simulink model "DYN_03x"  (R2021a)
settings: Solver=FixedStepAuto  StartTime=0.0  StopTime=10  FixedStep=0.001  RelTol=1e-3
(part 2 of 9)

== matlab function DYN_03x/MATLAB Function ==
  data: t input; e input; dde output; de input; Pic input; I1 input; I2 input; I3 input; I4 input; I5 input; I6 input; c input; b input; Fe input
function dde = fcn(t,e,de,Pic,I1,I2,I3,I4,I5,I6,c,b,Fe)
e1 = e(1); e2 = e(2); e3 = e(3);
e4 = e(4); e5 = e(5); e6 = e(6);
de1 = de(1); de2 = de(2); de3 = de(3);
de4 = de(4); de5 = de(5); de6 = de(6);
x1 = Pic(1,1); y1 = Pic(1,2); z1 = Pic(1,3);
x2 = Pic(2,1); y2 = Pic(2,2); z2 = Pic(2,3);
x3 = Pic(3,1); y3 = Pic(3,2); z3 = Pic(3,3);
x4 = Pic(4,1); y4 = Pic(4,2); z4 = Pic(4,3);
x5 = Pic(5,1); y5 = Pic(5,2); z5 = Pic(5,3);
x6 = Pic(6,1); y6 = Pic(6,2); z6 = Pic(6,3);
I1xx = I1(1,1); I1xy = I1(1,2); I1xz = I1(1,3);
I1yx = I1(2,1); I1yy = I1(2,2); I1yz = I1(2,3);
I1zx = I1(3,1); I1zy = I1(3,2); I1zz = I1(3,3);

I2xx = I2(1,1); I2xy = I2(1,2); I2xz = I2(1,3);
I2yx = I2(2,1); I2yy = I2(2,2); I2yz = I2(2,3);
I2zx = I2(3,1); I2zy = I2(3,2); I2zz = I2(3,3);

I3xx = I3(1,1); I3xy = I3(1,2); I3xz = I3(1,3);
I3yx = I3(2,1); I3yy = I3(2,2); I3yz = I3(2,3);
I3zx = I3(3,1); I3zy = I3(3,2); I3zz = I3(3,3);

I4xx = I4(1,1); I4xy = I4(1,2); I4xz = I4(1,3);
I4yx = I4(2,1); I4yy = I4(2,2); I4yz = I4(2,3);
I4zx = I4(3,1); I4zy = I4(3,2); I4zz = I4(3,3);

I5xx = I5(1,1); I5xy = I5(1,2); I5xz = I5(1,3);
I5yx = I5(2,1); I5yy = I5(2,2); I5yz = I5(2,3);
I5zx = I5(3,1); I5zy = I5(3,2); I5zz = I5(3,3);

I6xx = I6(1,1); I6xy = I6(1,2); I6xz = I6(1,3);
I6yx = I6(2,1); I6yy = I6(2,2); I6yz = I6(2,3);
I6zx = I6(3,1); I6zy = I6(3,2); I6zz = I6(3,3);
a1=0.75; a2=2.70; a3=0.90; d1=3.35; d4=2.95; d7=0.80;
m0 = 7.2407; m1 = 5.6511; m2 = 4.6061; m3 = 4.2963; m4 = 1.9151; m5 = 0.3399; m6 = 0.0714;
g = 9.80665;
%% 
M = ...
[I1zz + m5*(a1*sin(e1) + z5*cos(e1)*cos(e4) + a2*sin(e1)*sin(e2) + d4*cos(e2)*cos(e3)*sin(e1) + a3*cos(e2)*sin(e1)*sin(e3) + a3*cos(e3)*sin(e1)*sin(e2) - x5*cos(e1)*cos(e5)*sin(e4) - d4*sin(e1)*sin(e2)*sin(e3) + y5*cos(e1)*sin(e4)*sin(e5) + y5*cos(e2)*cos(e3)*cos(e5)*sin(e1) + x5*cos(e2)*cos(e3)*sin(e1)*sin(e5) - y5*cos(e5)*sin(e1)*sin(e2)*sin(e3) + z5*cos(e2)*sin(e1)*sin(e3)*sin(e4) + z5*cos(e3)*sin(e1)*sin(e2)*sin(e4) - x5*sin(e1)*sin(e2)*sin(e3)*sin(e5) + x5*cos(e2)*cos(e4)*cos(e5)*sin(e1)*sin(e3) + x5*cos(e3)*cos(e4)*cos(e5)*sin(e1)*sin(e2) - y5*cos(e2)*cos(e4)*sin(e1)*sin(e3)*sin(e5) - y5*cos(e3)*cos(e4)*sin(e1)*sin(e2)*sin(e5))^2 + m6*(d4*cos(e1)*sin(e2)*sin(e3) - a2*cos(e1)*sin(e2) - d4*cos(e1)*cos(e2)*cos(e3) - a3*cos(e1)*cos(e2)*sin(e3) - a3*cos(e1)*cos(e3)*sin(e2) - a1*cos(e1) - y6*cos(e4)*cos(e6)*sin(e1) - x6*cos(e4)*sin(e1)*sin(e6) + z6*sin(e1)*sin(e4)*sin(e5) - x6*cos(e5)*cos(e6)*sin(e1)*sin(e4) + z6*cos(e1)*cos(e5)*sin(e2)*sin(e3) + y6*cos(e5)*sin(e1)*sin(e4)*sin(e6) - z6*cos(e1)*cos(e2)*cos(e3)*cos(e5) - y6*cos(e1)*sin(e2)*sin(e3)*sin(e5)*sin(e6) - x6*cos(e1)*cos(e2)*cos(e3)*cos(e6)*sin(e5) + y6*cos(e1)*cos(e2)*cos(e6)*sin(e3)*sin(e4) + y6*cos(e1)*cos(e3)*cos(e6)*sin(e2)*sin(e4) + y6*cos(e1)*cos(e2)*cos(e3)*sin(e5)*sin(e6) + z6*cos(e1)*cos(e2)*cos(e4)*sin(e3)*sin(e5) + z6*cos(e1)*cos(e3)*cos(e4)*sin(e2)*sin(e5) + x6*cos(e1)*cos(e2)*sin(e3)*sin(e4)*sin(e6) + x6*cos(e1)*cos(e3)*sin(e2)*sin(e4)*sin(e6) + x6*cos(e1)*cos(e6)*sin(e2)*sin(e3)*sin(e5) - x6*cos(e1)*cos(e2)*cos(e4)*cos(e5)*cos(e6)*sin(e3) - x6*cos(e1)*cos(e3)*cos(e4)*cos(e5)*cos(e6)*sin(e2) + y6*cos(e1)*cos(e2)*cos(e4)*cos(e5)*sin(e3)*sin(e6) + y6*cos(e1)*cos(e3)*cos(e4)*cos(e5)*sin(e2)*sin(e6))^2 + m6*(y6*cos(e1)*cos(e4)*cos(e6) - a2*sin(e1)*sin(e2) - d4*cos(e2)*cos(e3)*sin(e1) - a1*sin(e1) - a3*cos(e2)*sin(e1)*sin(e3) - a3*cos(e3)*sin(e1)*sin(e2) + x6*cos(e1)*cos(e4)*sin(e6) + d4*sin(e1)*sin(e2)*sin(e3) - z6*cos(e1)*sin(e4)*sin(e5) + x6*cos(e1)*cos(e5)*cos(e6)*sin(e4) - z6*cos(e2)*cos(e3)*cos(e5)*sin(e1) - y6*cos(e1)*cos(e5)*sin(e4)*sin(e6) + z6*cos(e5)*sin(e1)*sin(e2)*sin(e3) + x6*cos(e2)*sin(e1)*sin(e3)*sin(e4)*sin(e6) + x6*cos(e3)*sin(e1)*sin(e2)*sin(e4)*sin(e6) + x6*cos(e6)*sin(e1)*sin(e2)*sin(e3)*sin(e5) - y6*sin(e1)*sin(e2)*sin(e3)*sin(e5)*sin(e6) - x6*cos(e2)*cos(e3)*cos(e6)*sin(e1)*sin(e5) + y6*cos(e2)*cos(e6)*sin(e1)*sin(e3)*sin(e4) + y6*cos(e3)*cos(e6)*sin(e1)*sin(e2)*sin(e4) + y6*cos(e2)*cos(e3)*sin(e1)*sin(e5)*sin(e6) + z6*cos(e2)*cos(e4)*sin(e1)*sin(e3)*sin(e5) + z6*cos(e3)*cos(e4)*sin(e1)*sin(e2)*sin(e5) - x6*cos(e2)*cos(e4)*cos(e5)*cos(e6)*sin(e1)*sin(e3) - x6*cos(e3)*cos(e4)*cos(e5)*cos(e6)*sin(e1)*sin(e2) + y6*cos(e2)*cos(e4)*cos(e5)*sin(e1)*sin(e3)*sin(e6) + y6*cos(e3)*cos(e4)*cos(e5)*sin(e1)*sin(e2)*sin(e6))^2 + m3*(sin(e1)*(a1 + y3*cos(e2 + e3) + x3*sin(e2 + e3) + a2*sin(e2)) + z3*cos(e2 + e3)^2*cos(e1) + z3*sin(e2 + e3)^2*cos(e1))^2 + m3*(z3*cos(e2 + e3)^2*sin(e1) - cos(e1)*(a1 + y3*cos(e2 + e3) + x3*sin(e2 + e3) + a2*sin(e2)) + z3*sin(e2 + e3)^2*sin(e1))^2 + m5*(a1*cos(e1) + a2*cos(e1)*sin(e2) - z5*cos(e4)*sin(e1) + d4*cos(e1)*cos(e2)*cos(e3) + a3*cos(e1)*cos(e2)*sin(e3) + a3*cos(e1)*cos(e3)*sin(e2) - d4*cos(e1)*sin(e2)*sin(e3) + x5*cos(e5)*sin(e1)*sin(e4) - y5*sin(e1)*sin(e4)*sin(e5) + x5*cos(e1)*cos(e2)*cos(e3)*sin(e5) - y5*cos(e1)*cos(e5)*sin(e2)*sin(e3) + z5*cos(e1)*cos(e2)*sin(e3)*sin(e4) + z5*cos(e1)*cos(e3)*sin(e2)*sin(e4) - x5*cos(e1)*sin(e2)*sin(e3)*sin(e5) + y5*cos(e1)*cos(e2)*cos(e3)*cos(e5) + x5*cos(e1)*cos(e2)*cos(e4)*cos(e5)*sin(e3) + x5*cos(e1)*cos(e3)*cos(e4)*cos(e5)*sin(e2) - y5*cos(e1)*cos(e2)*cos(e4)*sin(e3)*sin(e5) - y5*cos(e1)*cos(e3)*cos(e4)*sin(e2)*sin(e5))^2 + m4*(a1*sin(e1) - y4*cos(e1)*cos(e4) + a2*sin(e1)*sin(e2) - x4*cos(e1)*sin(e4) + d4*cos(e2)*cos(e3)*sin(e1) + a3*cos(e2)*sin(e1)*sin(e3) + a3*cos(e3)*sin(e1)*sin(e2) + z4*cos(e2)*cos(e3)*sin(e1) - d4*sin(e1)*sin(e2)*sin(e3) - z4*sin(e1)*sin(e2)*sin(e3) + x4*cos(e2)*cos(e4)*sin(e1)*sin(e3) + x4*cos(e3)*cos(e4)*sin(e1)*sin(e2) - y4*cos(e2)*sin(e1)*sin(e3)*sin(e4) - y4*cos(e3)*sin(e1)*sin(e2)*sin(e4))^2 + I3xx*cos(e2 + e3)^2 + I3yy*sin(e2 + e3)^2 + I4zz*sin(e2 + e3)^2 + m2*(a1*cos(e1) - z2*sin(e1) + y2*cos(e1)*cos(e2) + x2*cos(e1)*sin(e2))^2 + I5xx*(sin(e2 + e3)*sin(e5) - cos(e2 + e3)*cos(e4)*cos(e5))^2 + I5yy*(sin(e2 + e3)*cos(e5) + cos(e2 + e3)*cos(e4)*sin(e5))^2 + I6zz*(sin(e2 + e3)*cos(e5) + cos(e2 + e3)*cos(e4)*sin(e5))^2 + m2*(a1*sin(e1) + z2*cos(e1) + y2*cos(e2)*sin(e1) + x2*sin(e1)*sin(e2))^2 + I2xx*cos(e2)^2 + m1*(y1*cos(e1) + x1*sin(e1))^2 + m1*(x1*cos(e1) - y1*sin(e1))^2 + I2yy*sin(e2)^2 + I6xx*(cos(e2 + e3)*sin(e4)*sin(e6) + sin(e2 + e3)*cos(e6)*sin(e5) - cos(e2 + e3)*cos(e4)*cos(e5)*cos(e6))^2 + m4*(a1*cos(e1) + a2*cos(e1)*sin(e2) + y4*cos(e4)*sin(e1) + x4*sin(e1)*sin(e4) + d4*cos(e1)*cos(e2)*cos(e3) + a3*cos(e1)*cos(e2)*sin(e3) + a3*cos(e1)*cos(e3)*sin(e2) + z4*cos(e1)*cos(e2)*cos(e3) - d4*cos(e1)*sin(e2)*sin(e3) - z4*cos(e1)*sin(e2)*sin(e3) + x4*cos(e1)*cos(e2)*cos(e4)*sin(e3) + x4*cos(e1)*cos(e3)*cos(e4)*sin(e2) - y4*cos(e1)*cos(e2)*sin(e3)*sin(e4) - y4*cos(e1)*cos(e3)*sin(e2)*sin(e4))^2 + I6yy*(cos(e2 + e3)*cos(e6)*sin(e4) - sin(e2 + e3)*sin(e5)*sin(e6) + cos(e2 + e3)*cos(e4)*cos(e5)*sin(e6))^2 + I4xx*cos(e2 + e3)^2*cos(e4)^2 + I4yy*cos(e2 + e3)^2*sin(e4)^2 + I5zz*cos(e2 + e3)^2*sin(e4)^2,m2*y2*z2*sin(e2) - m2*x2*z2*cos(e2) - a2*m3*z3*cos(e2) + a2*m4*y4*cos(e2)*cos(e4) - a2*m5*z5*cos(e2)*cos(e4) + a2*m4*x4*cos(e2)*sin(e4) - m4*x4*y4*cos(e2)*cos(e3) - m3*x3*z3*cos(e2)*cos(e3) + m3*y3*z3*cos(e2)*sin(e3) + m3*y3*z3*cos(e3)*sin(e2) + m4*x4*y4*sin(e2)*sin(e3) + m3*x3*z3*sin(e2)*sin(e3) - I4xx*cos(e2)*cos(e3)*cos(e4)*sin(e4) + I6xx*cos(e2)*cos(e3)*cos(e4)*sin(e4) + I4yy*cos(e2)*cos(e3)*cos(e4)*sin(e4) - I5yy*cos(e2)*cos(e3)*cos(e4)*sin(e4) + I5zz*cos(e2)*cos(e3)*cos(e4)*sin(e4) - I6zz*cos(e2)*cos(e3)*cos(e4)*sin(e4) + I4xx*cos(e4)*sin(e2)*sin(e3)*sin(e4) - I6xx*cos(e4)*sin(e2)*sin(e3)*sin(e4) - I4yy*cos(e4)*sin(e2)*sin(e3)*sin(e4) + I5yy*cos(e4)*sin(e2)*sin(e3)*sin(e4) - I5zz*cos(e4)*sin(e2)*sin(e3)*sin(e4) + I6zz*cos(e4)*sin(e2)*sin(e3)*sin(e4) - a3*m5*z5*cos(e2)*cos(e3)*cos(e4) - I5xx*cos(e2)*cos(e3)*cos(e4)*cos(e5)^2*sin(e4) - I6xx*cos(e2)*cos(e3)*cos(e4)*cos(e6)^2*sin(e4) + I5yy*cos(e2)*cos(e3)*cos(e4)*cos(e5)^2*sin(e4) - I6yy*cos(e2)*cos(e3)*cos(e4)*cos(e5)^2*sin(e4) + I6yy*cos(e2)*cos(e3)*cos(e4)*cos(e6)^2*sin(e4) + I6zz*cos(e2)*cos(e3)*cos(e4)*cos(e5)^2*sin(e4) + a3*m4*x4*cos(e2)*cos(e3)*sin(e4) + a2*m5*x5*cos(e2)*cos(e5)*sin(e4) + a2*m6*x6*cos(e2)*cos(e4)*sin(e6) - d4*m4*y4*cos(e2)*cos(e4)*sin(e3) - d4*m4*y4*cos(e3)*cos(e4)*sin(e2) + d4*m5*z5*cos(e2)*cos(e4)*sin(e3) + d4*m5*z5*cos(e3)*cos(e4)*sin(e2) + m6*x6*y6*cos(e2)*cos(e3)*cos(e5) + m5*x5*z5*cos(e2)*cos(e3)*cos(e5) - a3*m4*y4*cos(e4)*sin(e2)*sin(e3) - a2*m5*y5*cos(e2)*sin(e4)*sin(e5) + a3*m5*z5*cos(e4)*sin(e2)*sin(e3) - a2*m6*z6*cos(e2)*sin(e4)*sin(e5) - d4*m4*x4*cos(e2)*sin(e3)*sin(e4) - d4*m4*x4*cos(e3)*sin(e2)*sin(e4) + I5xx*cos(e4)*cos(e5)^2*sin(e2)*sin(e3)*sin(e4) + I6xx*cos(e4)*cos(e6)^2*sin(e2)*sin(e3)*sin(e4) - I5yy*cos(e4)*cos(e5)^2*sin(e2)*sin(e3)*sin(e4) + I6yy*cos(e4)*cos(e5)^2*sin(e2)*sin(e3)*sin(e4) - I6yy*cos(e4)*cos(e6)^2*sin(e2)*sin(e3)*sin(e4) - I6zz*cos(e4)*cos(e5)^2*sin(e2)*sin(e3)*sin(e4) - m4*y4*z4*cos(e2)*cos(e4)*sin(e3) - m4*y4*z4*cos(e3)*cos(e4)*sin(e2) - m5*y5*z5*cos(e2)*cos(e3)*sin(e5) - a3*m4*x4*sin(e2)*sin(e3)*sin(e4) + m5*x5*y5*cos(e2)*sin(e3)*sin(e4) + m5*x5*y5*cos(e3)*sin(e2)*sin(e4) - m6*x6*y6*cos(e5)*sin(e2)*sin(e3) - m4*x4*z4*cos(e2)*sin(e3)*sin(e4) - m4*x4*z4*cos(e3)*sin(e2)*sin(e4) - m5*x5*z5*cos(e5)*sin(e2)*sin(e3) + m5*y5*z5*sin(e2)*sin(e3)*sin(e5) + 2*m4*x4*y4*cos(e2)*cos(e3)*cos(e4)^2 - 2*m4*x4*y4*cos(e4)^2*sin(e2)*sin(e3) + I6xx*cos(e2)*cos(e3)*cos(e5)*cos(e6)*sin(e6) - I6yy*cos(e2)*cos(e3)*cos(e5)*cos(e6)*sin(e6) + I5xx*cos(e2)*cos(e5)*sin(e3)*sin(e4)*sin(e5) + I5xx*cos(e3)*cos(e5)*sin(e2)*sin(e4)*sin(e5) - I6xx*cos(e5)*cos(e6)*sin(e2)*sin(e3)*sin(e6) - I5yy*cos(e2)*cos(e5)*sin(e3)*sin(e4)*sin(e5) - I5yy*cos(e3)*cos(e5)*sin(e2)*sin(e4)*sin(e5) + I6yy*cos(e2)*cos(e5)*sin(e3)*sin(e4)*sin(e5) + I6yy*cos(e3)*cos(e5)*sin(e2)*sin(e4)*sin(e5) + I6yy*cos(e5)*cos(e6)*sin(e2)*sin(e3)*sin(e6) - I6zz*cos(e2)*cos(e5)*sin(e3)*sin(e4)*sin(e5) - I6zz*cos(e3)*cos(e5)*sin(e2)*sin(e4)*sin(e5) + m4*x4^2*cos(e2)*cos(e3)*cos(e4)*sin(e4) - m6*x6^2*cos(e2)*cos(e3)*cos(e4)*sin(e4) - m4*y4^2*cos(e2)*cos(e3)*cos(e4)*sin(e4) + m5*y5^2*cos(e2)*cos(e3)*cos(e4)*sin(e4) - m5*z5^2*cos(e2)*cos(e3)*cos(e4)*sin(e4) + m6*z6^2*cos(e2)*cos(e3)*cos(e4)*sin(e4) - m4*x4^2*cos(e4)*sin(e2)*sin(e3)*sin(e4) + m6*x6^2*cos(e4)*sin(e2)*sin(e3)*sin(e4) + m4*y4^2*cos(e4)*sin(e2)*sin(e3)*sin(e4) - m5*y5^2*cos(e4)*sin(e2)*sin(e3)*sin(e4) + m5*z5^2*cos(e4)*sin(e2)*sin(e3)*sin(e4) - m6*z6^2*cos(e4)*sin(e2)*sin(e3)*sin(e4) + a3*m4*y4*cos(e2)*cos(e3)*cos(e4) + a2*m6*y6*cos(e2)*cos(e4)*cos(e6) + m5*x5*z5*cos(e2)*cos(e4)*sin(e3)*sin(e5) + m5*x5*z5*cos(e3)*cos(e4)*sin(e2)*sin(e5) + m6*x6*z6*cos(e2)*cos(e6)*sin(e3)*sin(e4) + m6*x6*z6*cos(e3)*cos(e6)*sin(e2)*sin(e4) + m6*x6*z6*cos(e2)*cos(e3)*sin(e5)*sin(e6) + a3*m5*y5*sin(e2)*sin(e3)*sin(e4)*sin(e5) + a3*m6*z6*sin(e2)*sin(e3)*sin(e4)*sin(e5) - m6*y6*z6*cos(e2)*sin(e3)*sin(e4)*sin(e6) - m6*y6*z6*cos(e3)*sin(e2)*sin(e4)*sin(e6) - m6*y6*z6*cos(e6)*sin(e2)*sin(e3)*sin(e5) - m5*x5^2*cos(e4)*cos(e5)^2*sin(e2)*sin(e3)*sin(e4) - m6*x6^2*cos(e4)*cos(e6)^2*sin(e2)*sin(e3)*sin(e4) + m5*y5^2*cos(e4)*cos(e5)^2*sin(e2)*sin(e3)*sin(e4) - m6*y6^2*cos(e4)*cos(e5)^2*sin(e2)*sin(e3)*sin(e4) + m6*y6^2*cos(e4)*cos(e6)^2*sin(e2)*sin(e3)*sin(e4) + m6*z6^2*cos(e4)*cos(e5)^2*sin(e2)*sin(e3)*sin(e4) - m6*x6*z6*sin(e2)*sin(e3)*sin(e5)*sin(e6) - I6xx*cos(e2)*cos(e3)*cos(e4)*cos(e5)^2*cos(e6)^2*sin(e4) + I6yy*cos(e2)*cos(e3)*cos(e4)*cos(e5)^2*cos(e6)^2*sin(e4) - 2*m6*x6*y6*cos(e2)*cos(e3)*cos(e4)^2*cos(e5) - 2*m6*x6*y6*cos(e2)*cos(e3)*cos(e5)*cos(e6)^2 - 2*m5*x5*z5*cos(e2)*cos(e3)*cos(e4)^2*cos(e5) + I6xx*cos(e4)*cos(e5)^2*cos(e6)^2*sin(e2)*sin(e3)*sin(e4) - I6yy*cos(e4)*cos(e5)^2*cos(e6)^2*sin(e2)*sin(e3)*sin(e4) + 2*m5*y5*z5*cos(e2)*cos(e3)*cos(e4)^2*sin(e5) - 2*m5*x5*y5*cos(e2)*cos(e5)^2*sin(e3)*sin(e4) - 2*m5*x5*y5*cos(e3)*cos(e5)^2*sin(e2)*sin(e4) + 2*m6*x6*y6*cos(e4)^2*cos(e5)*sin(e2)*sin(e3) + 2*m6*x6*y6*cos(e5)*cos(e6)^2*sin(e2)*sin(e3) + 2*m5*x5*z5*cos(e4)^2*cos(e5)*sin(e2)*sin(e3) - 2*m5*y5*z5*cos(e4)^2*sin(e2)*sin(e3)*sin(e5) + I6xx*cos(e2)*cos(e4)*cos(e6)*sin(e3)*sin(e5)*sin(e6) + I6xx*cos(e3)*cos(e4)*cos(e6)*sin(e2)*sin(e5)*sin(e6) - I6yy*cos(e2)*cos(e4)*cos(e6)*sin(e3)*sin(e5)*sin(e6) - I6yy*cos(e3)*cos(e4)*cos(e6)*sin(e2)*sin(e5)*sin(e6) - m6*x6^2*cos(e2)*cos(e3)*cos(e5)*cos(e6)*sin(e6) + m6*y6^2*cos(e2)*cos(e3)*cos(e5)*cos(e6)*sin(e6) - m5*x5^2*cos(e2)*cos(e5)*sin(e3)*sin(e4)*sin(e5) - m5*x5^2*cos(e3)*cos(e5)*sin(e2)*sin(e4)*sin(e5) + m6*x6^2*cos(e5)*cos(e6)*sin(e2)*sin(e3)*sin(e6) + m5*y5^2*cos(e2)*cos(e5)*sin(e3)*sin(e4)*sin(e5) + m5*y5^2*cos(e3)*cos(e5)*sin(e2)*sin(e4)*sin(e5) - m6*y6^2*cos(e2)*cos(e5)*sin(e3)*sin(e4)*sin(e5) - m6*y6^2*cos(e3)*cos(e5)*sin(e2)*sin(e4)*sin(e5) - m6*y6^2*cos(e5)*cos(e6)*sin(e2)*sin(e3)*sin(e6) + m6*z6^2*cos(e2)*cos(e5)*sin(e3)*sin(e4)*sin(e5) + m6*z6^2*cos(e3)*cos(e5)*sin(e2)*sin(e4)*sin(e5) + a3*m6*y6*cos(e2)*cos(e3)*cos(e4)*cos(e6) - 2*I6xx*cos(e2)*cos(e3)*cos(e4)^2*cos(e5)*cos(e6)*sin(e6) + 2*I6yy*cos(e2)*cos(e3)*cos(e4)^2*cos(e5)*cos(e6)*sin(e6) + a3*m5*x5*cos(e2)*cos(e3)*cos(e5)*sin(e4) + a3*m6*x6*cos(e2)*cos(e3)*cos(e4)*sin(e6) + a2*m6*x6*cos(e2)*cos(e5)*cos(e6)*sin(e4) - d4*m6*y6*cos(e2)*cos(e4)*cos(e6)*sin(e3) - d4*m6*y6*cos(e3)*cos(e4)*cos(e6)*sin(e2) - a3*m5*y5*cos(e2)*cos(e3)*sin(e4)*sin(e5) - a3*m6*y6*cos(e4)*cos(e6)*sin(e2)*sin(e3) - a2*m6*y6*cos(e2)*cos(e5)*sin(e4)*sin(e6) - a3*m6*z6*cos(e2)*cos(e3)*sin(e4)*sin(e5) - d4*m5*x5*cos(e2)*cos(e5)*sin(e3)*sin(e4) - d4*m5*x5*cos(e3)*cos(e5)*sin(e2)*sin(e4) - d4*m6*x6*cos(e2)*cos(e4)*sin(e3)*sin(e6) - d4*m6*x6*cos(e3)*cos(e4)*sin(e2)*sin(e6) + I6xx*cos(e2)*cos(e5)*cos(e6)^2*sin(e3)*sin(e4)*sin(e5) + I6xx*cos(e3)*cos(e5)*cos(e6)^2*sin(e2)*sin(e4)*sin(e5) + 2*I6xx*cos(e4)^2*cos(e5)*cos(e6)*sin(e2)*sin(e3)*sin(e6) - I6yy*cos(e2)*cos(e5)*cos(e6)^2*sin(e3)*sin(e4)*sin(e5) - I6yy*cos(e3)*cos(e5)*cos(e6)^2*sin(e2)*sin(e4)*sin(e5) - 2*I6yy*cos(e4)^2*cos(e5)*cos(e6)*sin(e2)*sin(e3)*sin(e6) + m5*y5*z5*cos(e2)*cos(e4)*cos(e5)*sin(e3) + m5*y5*z5*cos(e3)*cos(e4)*cos(e5)*sin(e2) + m6*y6*z6*cos(e2)*cos(e3)*cos(e6)*sin(e5) - a3*m5*x5*cos(e5)*sin(e2)*sin(e3)*sin(e4) - a3*m6*x6*cos(e4)*sin(e2)*sin(e3)*sin(e6) + d4*m5*y5*cos(e2)*sin(e3)*sin(e4)*sin(e5) + d4*m5*y5*cos(e3)*sin(e2)*sin(e4)*sin(e5) + d4*m6*z6*cos(e2)*sin(e3)*sin(e4)*sin(e5) + d4*m6*z6*cos(e3)*sin(e2)*sin(e4)*sin(e5) + m5*x5^2*cos(e2)*cos(e3)*cos(e4)*cos(e5)^2*sin(e4) + m6*x6^2*cos(e2)*cos(e3)*cos(e4)*cos(e6)^2*sin(e4) - m5*y5^2*cos(e2)*cos(e3)*cos(e4)*cos(e5)^2*sin(e4) + m6*y6^2*cos(e2)*cos(e3)*cos(e4)*cos(e5)^2*sin(e4) - m6*y6^2*cos(e2)*cos(e3)*cos(e4)*cos(e6)^2*sin(e4) + m6*x6*y6*cos(e2)*cos(e4)*sin(e3)*sin(e5) + m6*x6*y6*cos(e3)*cos(e4)*sin(e2)*sin(e5) - m6*z6^2*cos(e2)*cos(e3)*cos(e4)*cos(e5)^2*sin(e4) - 2*m6*y6*z6*cos(e2)*cos(e3)*cos(e4)^2*cos(e6)*sin(e5) + m6*x6^2*cos(e2)*cos(e3)*cos(e4)*cos(e5)^2*cos(e6)^2*sin(e4) - m6*y6^2*cos(e2)*cos(e3)*cos(e4)*cos(e5)^2*cos(e6)^2*sin(e4) - 2*m6*x6*y6*cos(e2)*cos(e4)*cos(e6)^2*sin(e3)*sin(e5) - 2*m6*x6*y6*cos(e3)*cos(e4)*cos(e6)^2*sin(e2)*sin(e5) - 2*m6*x6*z6*cos(e2)*cos(e3)*cos(e4)^2*sin(e5)*sin(e6) - 2*m6*x6*z6*cos(e2)*cos(e5)^2*cos(e6)*sin(e3)*sin(e4) - 2*m6*x6*z6*cos(e3)*cos(e5)^2*cos(e6)*sin(e2)*sin(e4) + 2*m6*y6*z6*cos(e2)*cos(e5)^2*sin(e3)*sin(e4)*sin(e6) + 2*m6*y6*z6*cos(e3)*cos(e5)^2*sin(e2)*sin(e4)*sin(e6) + 2*m6*y6*z6*cos(e4)^2*cos(e6)*sin(e2)*sin(e3)*sin(e5) - m6*x6^2*cos(e4)*cos(e5)^2*cos(e6)^2*sin(e2)*sin(e3)*sin(e4) + m6*y6^2*cos(e4)*cos(e5)^2*cos(e6)^2*sin(e2)*sin(e3)*sin(e4) + 2*m6*x6*z6*cos(e4)^2*sin(e2)*sin(e3)*sin(e5)*sin(e6) + 4*m6*x6*y6*cos(e2)*cos(e3)*cos(e4)^2*cos(e5)*cos(e6)^2 - m6*x6^2*cos(e2)*cos(e4)*cos(e6)*sin(e3)*sin(e5)*sin(e6) - m6*x6^2*cos(e3)*cos(e4)*cos(e6)*sin(e2)*sin(e5)*sin(e6) - 4*m6*x6*y6*cos(e4)^2*cos(e5)*cos(e6)^2*sin(e2)*sin(e3) + m6*y6^2*cos(e2)*cos(e4)*cos(e6)*sin(e3)*sin(e5)*sin(e6) + m6*y6^2*cos(e3)*cos(e4)*cos(e6)*sin(e2)*sin(e5)*sin(e6) + a3*m6*x6*cos(e2)*cos(e3)*cos(e5)*cos(e6)*sin(e4) - a3*m6*y6*cos(e2)*cos(e3)*cos(e5)*sin(e4)*sin(e6) - d4*m6*x6*cos(e2)*cos(e5)*cos(e6)*sin(e3)*sin(e4) - d4*m6*x6*cos(e3)*cos(e5)*cos(e6)*sin(e2)*sin(e4) - m6*y6*z6*cos(e2)*cos(e4)*cos(e5)*cos(e6)*sin(e3) - m6*y6*z6*cos(e3)*cos(e4)*cos(e5)*cos(e6)*sin(e2) - a3*m6*x6*cos(e5)*cos(e6)*sin(e2)*sin(e3)*sin(e4) + d4*m6*y6*cos(e2)*cos(e5)*sin(e3)*sin(e4)*sin(e6) + d4*m6*y6*cos(e3)*cos(e5)*sin(e2)*sin(e4)*sin(e6) + 2*m6*x6^2*cos(e2)*cos(e3)*cos(e4)^2*cos(e5)*cos(e6)*sin(e6) - 2*m6*y6^2*cos(e2)*cos(e3)*cos(e4)^2*cos(e5)*cos(e6)*sin(e6) - m6*x6*z6*cos(e2)*cos(e4)*cos(e5)*sin(e3)*sin(e6) - m6*x6*z6*cos(e3)*cos(e4)*cos(e5)*sin(e2)*sin(e6) + a3*m6*y6*cos(e5)*sin(e2)*sin(e3)*sin(e4)*sin(e6) - m6*x6^2*cos(e2)*cos(e5)*cos(e6)^2*sin(e3)*sin(e4)*sin(e5) - m6*x6^2*cos(e3)*cos(e5)*cos(e6)^2*sin(e2)*sin(e4)*sin(e5) - 2*m6*x6^2*cos(e4)^2*cos(e5)*cos(e6)*sin(e2)*sin(e3)*sin(e6) + m6*y6^2*cos(e2)*cos(e5)*cos(e6)^2*sin(e3)*sin(e4)*sin(e5) + m6*y6^2*cos(e3)*cos(e5)*cos(e6)^2*sin(e2)*sin(e4)*sin(e5) + 2*m6*y6^2*cos(e4)^2*cos(e5)*cos(e6)*sin(e2)*sin(e3)*sin(e6) - 2*m5*x5*y5*cos(e2)*cos(e3)*cos(e4)*cos(e5)*sin(e4)*sin(e5) - 2*m6*x6*y6*cos(e2)*cos(e3)*cos(e4)*cos(e6)*sin(e4)*sin(e6) + 2*m5*x5*y5*cos(e4)*cos(e5)*sin(e2)*sin(e3)*sin(e4)*sin(e5) + 2*m6*x6*y6*cos(e4)*cos(e6)*sin(e2)*sin(e3)*sin(e4)*sin(e6) - 2*m6*x6*z6*cos(e2)*cos(e3)*cos(e4)*cos(e5)*cos(e6)*sin(e4)*sin(e5) + 2*m6*y6*z6*cos(e2)*cos(e3)*cos(e4)*cos(e5)*sin(e4)*sin(e5)*sin(e6) + 2*m6*x6*y6*cos(e2)*cos(e5)*cos(e6)*sin(e3)*sin(e4)*sin(e5)*sin(e6) + 2*m6*x6*y6*cos(e3)*cos(e5)*cos(e6)*sin(e2)*sin(e4)*sin(e5)*sin(e6) + 2*m6*x6*z6*cos(e4)*cos(e5)*cos(e6)*sin(e2)*sin(e3)*sin(e4)*sin(e5) - 2*m6*y6*z6*cos(e4)*cos(e5)*sin(e2)*sin(e3)*sin(e4)*sin(e5)*sin(e6) - 2*m6*x6*y6*cos(e2)*cos(e3)*cos(e4)*cos(e5)^2*cos(e6)*sin(e4)*sin(e6) + 2*m6*x6*y6*cos(e4)*cos(e5)^2*cos(e6)*sin(e2)*sin(e3)*sin(e4)*sin(e6),m3*y3*z3*cos(e2)*sin(e3) - m3*x3*z3*cos(e2)*cos(e3) - m4*x4*y4*cos(e2)*cos(e3) + m3*y3*z3*cos(e3)*sin(e2) + m4*x4*y4*sin(e2)*sin(e3) + m3*x3*z3*sin(e2)*sin(e3) - I4xx*cos(e2)*cos(e3)*cos(e4)*sin(e4) + I6xx*cos(e2)*cos(e3)*cos(e4)*sin(e4) + I4yy*cos(e2)*cos(e3)*cos(e4)*sin(e4) - I5yy*cos(e2)*cos(e3)*cos(e4)*sin(e4) + I5zz*cos(e2)*cos(e3)*cos(e4)*sin(e4) - I6zz*cos(e2)*cos(e3)*cos(e4)*sin(e4) + I4xx*cos(e4)*sin(e2)*sin(e3)*sin(e4) - I6xx*cos(e4)*sin(e2)*sin(e3)*sin(e4) - I4yy*cos(e4)*sin(e2)*sin(e3)*sin(e4) + I5yy*cos(e4)*sin(e2)*sin(e3)*sin(e4) - I5zz*cos(e4)*sin(e2)*sin(e3)*sin(e4) + I6zz*cos(e4)*sin(e2)*sin(e3)*sin(e4) - a3*m5*z5*cos(e2)*cos(e3)*cos(e4) - I5xx*cos(e2)*cos(e3)*cos(e4)*cos(e5)^2*sin(e4) - I6xx*cos(e2)*cos(e3)*cos(e4)*cos(e6)^2*sin(e4) + I5yy*cos(e2)*cos(e3)*cos(e4)*cos(e5)^2*sin(e4) - I6yy*cos(e2)*cos(e3)*cos(e4)*cos(e5)^2*sin(e4) + I6yy*cos(e2)*cos(e3)*cos(e4)*cos(e6)^2*sin(e4) + I6zz*cos(e2)*cos(e3)*cos(e4)*cos(e5)^2*sin(e4) + a3*m4*x4*cos(e2)*cos(e3)*sin(e4) - d4*m4*y4*cos(e2)*cos(e4)*sin(e3) - d4*m4*y4*cos(e3)*cos(e4)*sin(e2) + d4*m5*z5*cos(e2)*cos(e4)*sin(e3) + d4*m5*z5*cos(e3)*cos(e4)*sin(e2) + m6*x6*y6*cos(e2)*cos(e3)*cos(e5) + m5*x5*z5*cos(e2)*cos(e3)*cos(e5) - a3*m4*y4*cos(e4)*sin(e2)*sin(e3) + a3*m5*z5*cos(e4)*sin(e2)*sin(e3) - d4*m4*x4*cos(e2)*sin(e3)*sin(e4) - d4*m4*x4*cos(e3)*sin(e2)*sin(e4) + I5xx*cos(e4)*cos(e5)^2*sin(e2)*sin(e3)*sin(e4) + I6xx*cos(e4)*cos(e6)^2*sin(e2)*sin(e3)*sin(e4) - I5yy*cos(e4)*cos(e5)^2*sin(e2)*sin(e3)*sin(e4) + I6yy*cos(e4)*cos(e5)^2*sin(e2)*sin(e3)*sin(e4) - I6yy*cos(e4)*cos(e6)^2*sin(e2)*sin(e3)*sin(e4) - I6zz*cos(e4)*cos(e5)^2*sin(e2)*sin(e3)*sin(e4) - m4*y4*z4*cos(e2)*cos(e4)*sin(e3) - m4*y4*z4*cos(e3)*cos(e4)*sin(e2) - m5*y5*z5*cos(e2)*cos(e3)*sin(e5) - a3*m4*x4*sin(e2)*sin(e3)*sin(e4) + m5*x5*y5*cos(e2)*sin(e3)*sin(e4) + m5*x5*y5*cos(e3)*sin(e2)*sin(e4) - m6*x6*y6*cos(e5)*sin(e2)*sin(e3) - m4*x4*z4*cos(e2)*sin(e3)*sin(e4) - m4*x4*z4*cos(e3)*sin(e2)*sin(e4) - m5*x5*z5*cos(e5)*sin(e2)*sin(e3) + m5*y5*z5*sin(e2)*sin(e3)*sin(e5) + 2*m4*x4*y4*cos(e2)*cos(e3)*cos(e4)^2 - 2*m4*x4*y4*cos(e4)^2*sin(e2)*sin(e3) + I6xx*cos(e2)*cos(e3)*cos(e5)*cos(e6)*sin(e6) - I6yy*cos(e2)*cos(e3)*cos(e5)*cos(e6)*sin(e6) + I5xx*cos(e2)*cos(e5)*sin(e3)*sin(e4)*sin(e5) + I5xx*cos(e3)*cos(e5)*sin(e2)*sin(e4)*sin(e5) - I6xx*cos(e5)*cos(e6)*sin(e2)*sin(e3)*sin(e6) - I5yy*cos(e2)*cos(e5)*sin(e3)*sin(e4)*sin(e5) - I5yy*cos(e3)*cos(e5)*sin(e2)*sin(e4)*sin(e5) + I6yy*cos(e2)*cos(e5)*sin(e3)*sin(e4)*sin(e5) + I6yy*cos(e3)*cos(e5)*sin(e2)*sin(e4)*sin(e5) + I6yy*cos(e5)*cos(e6)*sin(e2)*sin(e3)*sin(e6) - I6zz*cos(e2)*cos(e5)*sin(e3)*sin(e4)*sin(e5) - I6zz*cos(e3)*cos(e5)*sin(e2)*sin(e4)*sin(e5) + m4*x4^2*cos(e2)*cos(e3)*cos(e4)*sin(e4) - m6*x6^2*cos(e2)*cos(e3)*cos(e4)*sin(e4) - m4*y4^2*cos(e2)*cos(e3)*cos(e4)*sin(e4) + m5*y5^2*cos(e2)*cos(e3)*cos(e4)*sin(e4) - m5*z5^2*cos(e2)*cos(e3)*cos(e4)*sin(e4) + m6*z6^2*cos(e2)*cos(e3)*cos(e4)*sin(e4) - m4*x4^2*cos(e4)*sin(e2)*sin(e3)*sin(e4) + m6*x6^2*cos(e4)*sin(e2)*sin(e3)*sin(e4) + m4*y4^2*cos(e4)*sin(e2)*sin(e3)*sin(e4) - m5*y5^2*cos(e4)*sin(e2)*sin(e3)*sin(e4) + m5*z5^2*cos(e4)*sin(e2)*sin(e3)*sin(e4) - m6*z6^2*cos(e4)*sin(e2)*sin(e3)*sin(e4) + a3*m4*y4*cos(e2)*cos(e3)*cos(e4) + m5*x5*z5*cos(e2)*cos(e4)*sin(e3)*sin(e5) + m5*x5*z5*cos(e3)*cos(e4)*sin(e2)*sin(e5) + m6*x6*z6*cos(e2)*cos(e6)*sin(e3)*sin(e4) + m6*x6*z6*cos(e3)*cos(e6)*sin(e2)*sin(e4) + m6*x6*z6*cos(e2)*cos(e3)*sin(e5)*sin(e6) + a3*m5*y5*sin(e2)*sin(e3)*sin(e4)*sin(e5) + a3*m6*z6*sin(e2)*sin(e3)*sin(e4)*sin(e5) - m6*y6*z6*cos(e2)*sin(e3)*sin(e4)*sin(e6) - m6*y6*z6*cos(e3)*sin(e2)*sin(e4)*sin(e6) - m6*y6*z6*cos(e6)*sin(e2)*sin(e3)*sin(e5) - m5*x5^2*cos(e4)*cos(e5)^2*sin(e2)*sin(e3)*sin(e4) - m6*x6^2*cos(e4)*cos(e6)^2*sin(e2)*sin(e3)*sin(e4) + m5*y5^2*cos(e4)*cos(e5)^2*sin(e2)*sin(e3)*sin(e4) - m6*y6^2*cos(e4)*cos(e5)^2*sin(e2)*sin(e3)*sin(e4) + m6*y6^2*cos(e4)*cos(e6)^2*sin(e2)*sin(e3)*sin(e4) + m6*z6^2*cos(e4)*cos(e5)^2*sin(e2)*sin(e3)*sin(e4) - m6*x6*z6*sin(e2)*sin(e3)*sin(e5)*sin(e6) - I6xx*cos(e2)*cos(e3)*cos(e4)*cos(e5)^2*cos(e6)^2*sin(e4) + I6yy*cos(e2)*cos(e3)*cos(e4)*cos(e5)^2*cos(e6)^2*sin(e4) - 2*m6*x6*y6*cos(e2)*cos(e3)*cos(e4)^2*cos(e5) - 2*m6*x6*y6*cos(e2)*cos(e3)*cos(e5)*cos(e6)^2 - 2*m5*x5*z5*cos(e2)*cos(e3)*cos(e4)^2*cos(e5) + I6xx*cos(e4)*cos(e5)^2*cos(e6)^2*sin(e2)*sin(e3)*sin(e4) - I6yy*cos(e4)*cos(e5)^2*cos(e6)^2*sin(e2)*sin(e3)*sin(e4) + 2*m5*y5*z5*cos(e2)*cos(e3)*cos(e4)^2*sin(e5) - 2*m5*x5*y5*cos(e2)*cos(e5)^2*sin(e3)*sin(e4) - 2*m5*x5*y5*cos(e3)*cos(e5)^2*sin(e2)*sin(e4) + 2*m6*x6*y6*cos(e4)^2*cos(e5)*sin(e2)*sin(e3) + 2*m6*x6*y6*cos(e5)*cos(e6)^2*sin(e2)*sin(e3) + 2*m5*x5*z5*cos(e4)^2*cos(e5)*sin(e2)*sin(e3) - 2*m5*y5*z5*cos(e4)^2*sin(e2)*sin(e3)*sin(e5) + I6xx*cos(e2)*cos(e4)*cos(e6)*sin(e3)*sin(e5)*sin(e6) + I6xx*cos(e3)*cos(e4)*cos(e6)*sin(e2)*sin(e5)*sin(e6) - I6yy*cos(e2)*cos(e4)*cos(e6)*sin(e3)*sin(e5)*sin(e6) - I6yy*cos(e3)*cos(e4)*cos(e6)*sin(e2)*sin(e5)*sin(e6) - m6*x6^2*cos(e2)*cos(e3)*cos(e5)*cos(e6)*sin(e6) + m6*y6^2*cos(e2)*cos(e3)*cos(e5)*cos(e6)*sin(e6) - m5*x5^2*cos(e2)*cos(e5)*sin(e3)*sin(e4)*sin(e5) - m5*x5^2*cos(e3)*cos(e5)*sin(e2)*sin(e4)*sin(e5) + m6*x6^2*cos(e5)*cos(e6)*sin(e2)*sin(e3)*sin(e6) + m5*y5^2*cos(e2)*cos(e5)*sin(e3)*sin(e4)*sin(e5) + m5*y5^2*cos(e3)*cos(e5)*sin(e2)*sin(e4)*sin(e5) - m6*y6^2*cos(e2)*cos(e5)*sin(e3)*sin(e4)*sin(e5) - m6*y6^2*cos(e3)*cos(e5)*sin(e2)*sin(e4)*sin(e5) - m6*y6^2*cos(e5)*cos(e6)*sin(e2)*sin(e3)*sin(e6) + m6*z6^2*cos(e2)*cos(e5)*sin(e3)*sin(e4)*sin(e5) + m6*z6^2*cos(e3)*cos(e5)*sin(e2)*sin(e4)*sin(e5) + a3*m6*y6*cos(e2)*cos(e3)*cos(e4)*cos(e6) - 2*I6xx*cos(e2)*cos(e3)*cos(e4)^2*cos(e5)*cos(e6)*sin(e6) + 2*I6yy*cos(e2)*cos(e3)*cos(e4)^2*cos(e5)*cos(e6)*sin(e6) + a3*m5*x5*cos(e2)*cos(e3)*cos(e5)*sin(e4) + a3*m6*x6*cos(e2)*cos(e3)*cos(e4)*sin(e6) - d4*m6*y6*cos(e2)*cos(e4)*cos(e6)*sin(e3) - d4*m6*y6*cos(e3)*cos(e4)*cos(e6)*sin(e2) - a3*m5*y5*cos(e2)*cos(e3)*sin(e4)*sin(e5) - a3*m6*y6*cos(e4)*cos(e6)*sin(e2)*sin(e3) - a3*m6*z6*cos(e2)*cos(e3)*sin(e4)*sin(e5) - d4*m5*x5*cos(e2)*cos(e5)*sin(e3)*sin(e4) - d4*m5*x5*cos(e3)*cos(e5)*sin(e2)*sin(e4) - d4*m6*x6*cos(e2)*cos(e4)*sin(e3)*sin(e6) - d4*m6*x6*cos(e3)*cos(e4)*sin(e2)*sin(e6) + I6xx*cos(e2)*cos(e5)*cos(e6)^2*sin(e3)*sin(e4)*sin(e5) + I6xx*cos(e3)*cos(e5)*cos(e6)^2*sin(e2)*sin(e4)*sin(e5) + 2*I6xx*cos(e4)^2*cos(e5)*cos(e6)*sin(e2)*sin(e3)*sin(e6) - I6yy*cos(e2)*cos(e5)*cos(e6)^2*sin(e3)*sin(e4)*sin(e5) - I6yy*cos(e3)*cos(e5)*cos(e6)^2*sin(e2)*sin(e4)*sin(e5) - 2*I6yy*cos(e4)^2*cos(e5)*cos(e6)*sin(e2)*sin(e3)*sin(e6) + m5*y5*z5*cos(e2)*cos(e4)*cos(e5)*sin(e3) + m5*y5*z5*cos(e3)*cos(e4)*cos(e5)*sin(e2) + m6*y6*z6*cos(e2)*cos(e3)*cos(e6)*sin(e5) - a3*m5*x5*cos(e5)*sin(e2)*sin(e3)*sin(e4) - a3*m6*x6*cos(e4)*sin(e2)*sin(e3)*sin(e6) + d4*m5*y5*cos(e2)*sin(e3)*sin(e4)*sin(e5) + d4*m5*y5*cos(e3)*sin(e2)*sin(e4)*sin(e5) + d4*m6*z6*cos(e2)*sin(e3)*sin(e4)*sin(e5) + d4*m6*z6*cos(e3)*sin(e2)*sin(e4)*sin(e5) + m5*x5^2*cos(e2)*cos(e3)*cos(e4)*cos(e5)^2*sin(e4) + m6*x6^2*cos(e2)*cos(e3)*cos(e4)*cos(e6)^2*sin(e4) - m5*y5^2*cos(e2)*cos(e3)*cos(e4)*cos(e5)^2*sin(e4) + m6*y6^2*cos(e2)*cos(e3)*cos(e4)*cos(e5)^2*sin(e4) - m6*y6^2*cos(e2)*cos(e3)*cos(e4)*cos(e6)^2*sin(e4) + m6*x6*y6*cos(e2)*cos(e4)*sin(e3)*sin(e5) + m6*x6*y6*cos(e3)*cos(e4)*sin(e2)*sin(e5) - m6*z6^2*cos(e2)*cos(e3)*cos(e4)*cos(e5)^2*sin(e4) - 2*m6*y6*z6*cos(e2)*cos(e3)*cos(e4)^2*cos(e6)*sin(e5) + m6*x6^2*cos(e2)*cos(e3)*cos(e4)*cos(e5)^2*cos(e6)^2*sin(e4) - m6*y6^2*cos(e2)*cos(e3)*cos(e4)*cos(e5)^2*cos(e6)^2*sin(e4) - 2*m6*x6*y6*cos(e2)*cos(e4)*cos(e6)^2*sin(e3)*sin(e5) - 2*m6*x6*y6*cos(e3)*cos(e4)*cos(e6)^2*sin(e2)*sin(e5) - 2*m6*x6*z6*cos(e2)*cos(e3)*cos(e4)^2*sin(e5)*sin(e6) - 2*m6*x6*z6*cos(e2)*cos(e5)^2*cos(e6)*sin(e3)*sin(e4) - 2*m6*x6*z6*cos(e3)*cos(e5)^2*cos(e6)*sin(e2)*sin(e4) + 2*m6*y6*z6*cos(e2)*cos(e5)^2*sin(e3)*sin(e4)*sin(e6) + 2*m6*y6*z6*cos(e3)*cos(e5)^2*sin(e2)*sin(e4)*sin(e6) + 2*m6*y6*z6*cos(e4)^2*cos(e6)*sin(e2)*sin(e3)*sin(e5) - m6*x6^2*cos(e4)*cos(e5)^2*cos(e6)^2*sin(e2)*sin(e3)*sin(e4) + m6*y6^2*cos(e4)*cos(e5)^2*cos(e6)^2*sin(e2)*sin(e3)*sin(e4) + 2*m6*x6*z6*cos(e4)^2*sin(e2)*sin(e3)*sin(e5)*sin(e6) + 4*m6*x6*y6*cos(e2)*cos(e3)*cos(e4)^2*cos(e5)*cos(e6)^2 - m6*x6^2*cos(e2)*cos(e4)*cos(e6)*sin(e3)*sin(e5)*sin(e6) - m6*x6^2*cos(e3)*cos(e4)*cos(e6)*sin(e2)*sin(e5)*sin(e6) - 4*m6*x6*y6*cos(e4)^2*cos(e5)*cos(e6)^2*sin(e2)*sin(e3) + m6*y6^2*cos(e2)*cos(e4)*cos(e6)*sin(e3)*sin(e5)*sin(e6) + m6*y6^2*cos(e3)*cos(e4)*cos(e6)*sin(e2)*sin(e5)*sin(e6) + a3*m6*x6*cos(e2)*cos(e3)*cos(e5)*cos(e6)*sin(e4) - a3*m6*y6*cos(e2)*cos(e3)*cos(e5)*sin(e4)*sin(e6) - d4*m6*x6*cos(e2)*cos(e5)*cos(e6)*sin(e3)*sin(e4) - d4*m6*x6*cos(e3)*cos(e5)*cos(e6)*sin(e2)*sin(e4) - m6*y6*z6*cos(e2)*cos(e4)*cos(e5)*cos(e6)*sin(e3) - m6*y6*z6*cos(e3)*cos(e4)*cos(e5)*cos(e6)*sin(e2) - a3*m6*x6*cos(e5)*cos(e6)*sin(e2)*sin(e3)*sin(e4) + d4*m6*y6*cos(e2)*cos(e5)*sin(e3)*sin(e4)*sin(e6) + d4*m6*y6*cos(e3)*cos(e5)*sin(e2)*sin(e4)*sin(e6) + 2*m6*x6^2*cos(e2)*cos(e3)*cos(e4)^2*cos(e5)*cos(e6)*sin(e6) - 2*m6*y6^2*cos(e2)*cos(e3)*cos(e4)^2*cos(e5)*cos(e6)*sin(e6) - m6*x6*z6*cos(e2)*cos(e4)*cos(e5)*sin(e3)*sin(e6) - m6*x6*z6*cos(e3)*cos(e4)*cos(e5)*sin(e2)*sin(e6) + a3*m6*y6*cos(e5)*sin(e2)*sin(e3)*sin(e4)*sin(e6) - m6*x6^2*cos(e2)*cos(e5)*cos(e6)^2*sin(e3)*sin(e4)*sin(e5) - m6*x6^2*cos(e3)*cos(e5)*cos(e6)^2*sin(e2)*sin(e4)*sin(e5) - 2*m6*x6^2*cos(e4)^2*cos(e5)*cos(e6)*sin(e2)*sin(e3)*sin(e6) + m6*y6^2*cos(e2)*cos(e5)*cos(e6)^2*sin(e3)*sin(e4)*sin(e5) + m6*y6^2*cos(e3)*cos(e5)*cos(e6)^2*sin(e2)*sin(e4)*sin(e5) + 2*m6*y6^2*cos(e4)^2*cos(e5)*cos(e6)*sin(e2)*sin(e3)*sin(e6) - 2*m5*x5*y5*cos(e2)*cos(e3)*cos(e4)*cos(e5)*sin(e4)*sin(e5) - 2*m6*x6*y6*cos(e2)*cos(e3)*cos(e4)*cos(e6)*sin(e4)*sin(e6) + 2*m5*x5*y5*cos(e4)*cos(e5)*sin(e2)*sin(e3)*sin(e4)*sin(e5) + 2*m6*x6*y6*cos(e4)*cos(e6)*sin(e2)*sin(e3)*sin(e4)*sin(e6) - 2*m6*x6*z6*cos(e2)*cos(e3)*cos(e4)*cos(e5)*cos(e6)*sin(e4)*sin(e5) + 2*m6*y6*z6*cos(e2)*cos(e3)*cos(e4)*cos(e5)*sin(e4)*sin(e5)*sin(e6) + 2*m6*x6*y6*cos(e2)*cos(e5)*cos(e6)*sin(e3)*sin(e4)*sin(e5)*sin(e6) + 2*m6*x6*y6*cos(e3)*cos(e5)*cos(e6)*sin(e2)*sin(e4)*sin(e5)*sin(e6) + 2*m6*x6*z6*cos(e4)*cos(e5)*cos(e6)*sin(e2)*sin(e3)*sin(e4)*sin(e5) - 2*m6*y6*z6*cos(e4)*cos(e5)*sin(e2)*sin(e3)*sin(e4)*sin(e5)*sin(e6) - 2*m6*x6*y6*cos(e2)*cos(e3)*cos(e4)*cos(e5)^2*cos(e6)*sin(e4)*sin(e6) + 2*m6*x6*y6*cos(e4)*cos(e5)^2*cos(e6)*sin(e2)*sin(e3)*sin(e4)*sin(e6),I5xx*cos(e2)*cos(e5)^2*sin(e3) - I5xx*cos(e3)*sin(e2) - I6yy*cos(e2)*sin(e3) - I6yy*cos(e3)*sin(e2) - I4zz*cos(e2)*sin(e3) - I4zz*cos(e3)*sin(e2) - m4*x4^2*cos(e2)*sin(e3) - m4*x4^2*cos(e3)*sin(e2) - m6*x6^2*cos(e2)*sin(e3) - m6*x6^2*cos(e3)*sin(e2) - m4*y4^2*cos(e2)*sin(e3) - m4*y4^2*cos(e3)*sin(e2) - m5*y5^2*cos(e2)*sin(e3) - m5*y5^2*cos(e3)*sin(e2) - m5*z5^2*cos(e2)*sin(e3) - m5*z5^2*cos(e3)*sin(e2) - m6*z6^2*cos(e2)*sin(e3) - m6*z6^2*cos(e3)*sin(e2) - a1*m4*x4*cos(e4) - I5xx*cos(e2)*sin(e3) + I5xx*cos(e3)*cos(e5)^2*sin(e2) - I6xx*cos(e2)*cos(e6)^2*sin(e3) - I6xx*cos(e3)*cos(e6)^2*sin(e2) - I5yy*cos(e2)*cos(e5)^2*sin(e3) - I5yy*cos(e3)*cos(e5)^2*sin(e2) + I6yy*cos(e2)*cos(e5)^2*sin(e3) + I6yy*cos(e3)*cos(e5)^2*sin(e2) + I6yy*cos(e2)*cos(e6)^2*sin(e3) + I6yy*cos(e3)*cos(e6)^2*sin(e2) - I6zz*cos(e2)*cos(e5)^2*sin(e3) - I6zz*cos(e3)*cos(e5)^2*sin(e2) + a1*m4*y4*sin(e4) - a1*m5*z5*sin(e4) - a1*m5*x5*cos(e4)*cos(e5) - a2*m4*x4*cos(e4)*sin(e2) + a1*m5*y5*cos(e4)*sin(e5) + a1*m6*y6*cos(e6)*sin(e4) + a1*m6*z6*cos(e4)*sin(e5) + a1*m6*x6*sin(e4)*sin(e6) + a2*m4*y4*sin(e2)*sin(e4) - a2*m5*z5*sin(e2)*sin(e4) - m5*x5^2*cos(e2)*cos(e5)^2*sin(e3) - m5*x5^2*cos(e3)*cos(e5)^2*sin(e2) + m6*x6^2*cos(e2)*cos(e6)^2*sin(e3) + m6*x6^2*cos(e3)*cos(e6)^2*sin(e2) + m5*y5^2*cos(e2)*cos(e5)^2*sin(e3) + m5*y5^2*cos(e3)*cos(e5)^2*sin(e2) - m6*y6^2*cos(e2)*cos(e5)^2*sin(e3) - m6*y6^2*cos(e3)*cos(e5)^2*sin(e2) - m6*y6^2*cos(e2)*cos(e6)^2*sin(e3) - m6*y6^2*cos(e3)*cos(e6)^2*sin(e2) + m6*z6^2*cos(e2)*cos(e5)^2*sin(e3) + m6*z6^2*cos(e3)*cos(e5)^2*sin(e2) + I6xx*cos(e2)*cos(e5)^2*cos(e6)^2*sin(e3) + I6xx*cos(e3)*cos(e5)^2*cos(e6)^2*sin(e2) - I6yy*cos(e2)*cos(e5)^2*cos(e6)^2*sin(e3) - I6yy*cos(e3)*cos(e5)^2*cos(e6)^2*sin(e2) - d4*m4*x4*cos(e2)*cos(e3)*cos(e4) - a3*m4*x4*cos(e2)*cos(e4)*sin(e3) - a3*m4*x4*cos(e3)*cos(e4)*sin(e2) - a2*m5*x5*cos(e4)*cos(e5)*sin(e2) + a1*m6*y6*cos(e4)*cos(e5)*sin(e6) + d4*m4*y4*cos(e2)*cos(e3)*sin(e4) - d4*m5*z5*cos(e2)*cos(e3)*sin(e4) + m5*x5*y5*cos(e2)*cos(e3)*cos(e4) - m4*x4*z4*cos(e2)*cos(e3)*cos(e4) + a3*m4*y4*cos(e2)*sin(e3)*sin(e4) + a3*m4*y4*cos(e3)*sin(e2)*sin(e4) + a2*m5*y5*cos(e4)*sin(e2)*sin(e5) + a2*m6*y6*cos(e6)*sin(e2)*sin(e4) - a3*m5*z5*cos(e2)*sin(e3)*sin(e4) - a3*m5*z5*cos(e3)*sin(e2)*sin(e4) + a2*m6*z6*cos(e4)*sin(e2)*sin(e5) + d4*m4*x4*cos(e4)*sin(e2)*sin(e3) + m4*y4*z4*cos(e2)*cos(e3)*sin(e4) + a2*m6*x6*sin(e2)*sin(e4)*sin(e6) - d4*m4*y4*sin(e2)*sin(e3)*sin(e4) + d4*m5*z5*sin(e2)*sin(e3)*sin(e4) - m5*x5*y5*cos(e4)*sin(e2)*sin(e3) + m4*x4*z4*cos(e4)*sin(e2)*sin(e3) - m4*y4*z4*sin(e2)*sin(e3)*sin(e4) - m6*x6^2*cos(e2)*cos(e5)^2*cos(e6)^2*sin(e3) - m6*x6^2*cos(e3)*cos(e5)^2*cos(e6)^2*sin(e2) + m6*y6^2*cos(e2)*cos(e5)^2*cos(e6)^2*sin(e3) + m6*y6^2*cos(e3)*cos(e5)^2*cos(e6)^2*sin(e2) + I5xx*cos(e2)*cos(e3)*cos(e4)*cos(e5)*sin(e5) - I5yy*cos(e2)*cos(e3)*cos(e4)*cos(e5)*sin(e5) + I6yy*cos(e2)*cos(e3)*cos(e4)*cos(e5)*sin(e5) - I6zz*cos(e2)*cos(e3)*cos(e4)*cos(e5)*sin(e5) - I5xx*cos(e4)*cos(e5)*sin(e2)*sin(e3)*sin(e5) + I5yy*cos(e4)*cos(e5)*sin(e2)*sin(e3)*sin(e5) - I6yy*cos(e4)*cos(e5)*sin(e2)*sin(e3)*sin(e5) + I6zz*cos(e4)*cos(e5)*sin(e2)*sin(e3)*sin(e5) - a1*m6*x6*cos(e4)*cos(e5)*cos(e6) - m5*x5*z5*cos(e2)*cos(e3)*sin(e4)*sin(e5) - m6*x6*z6*cos(e4)*cos(e6)*sin(e2)*sin(e3) - d4*m6*x6*sin(e2)*sin(e3)*sin(e4)*sin(e6) + m5*y5*z5*cos(e5)*sin(e2)*sin(e3)*sin(e4) + m6*y6*z6*cos(e4)*sin(e2)*sin(e3)*sin(e6) + m6*x6*y6*sin(e2)*sin(e3)*sin(e4)*sin(e5) + m5*x5*z5*sin(e2)*sin(e3)*sin(e4)*sin(e5) - 2*m5*x5*y5*cos(e2)*cos(e3)*cos(e4)*cos(e5)^2 + 2*m5*x5*y5*cos(e4)*cos(e5)^2*sin(e2)*sin(e3) - I6xx*cos(e2)*cos(e3)*cos(e6)*sin(e4)*sin(e5)*sin(e6) + I6yy*cos(e2)*cos(e3)*cos(e6)*sin(e4)*sin(e5)*sin(e6) - m5*x5^2*cos(e2)*cos(e3)*cos(e4)*cos(e5)*sin(e5) + m5*y5^2*cos(e2)*cos(e3)*cos(e4)*cos(e5)*sin(e5) - m6*y6^2*cos(e2)*cos(e3)*cos(e4)*cos(e5)*sin(e5) + m6*z6^2*cos(e2)*cos(e3)*cos(e4)*cos(e5)*sin(e5) + I6xx*cos(e6)*sin(e2)*sin(e3)*sin(e4)*sin(e5)*sin(e6) - I6yy*cos(e6)*sin(e2)*sin(e3)*sin(e4)*sin(e5)*sin(e6) + m5*x5^2*cos(e4)*cos(e5)*sin(e2)*sin(e3)*sin(e5) - m5*y5^2*cos(e4)*cos(e5)*sin(e2)*sin(e3)*sin(e5) + m6*y6^2*cos(e4)*cos(e5)*sin(e2)*sin(e3)*sin(e5) - m6*z6^2*cos(e4)*cos(e5)*sin(e2)*sin(e3)*sin(e5) - d4*m5*x5*cos(e2)*cos(e3)*cos(e4)*cos(e5) + I6xx*cos(e2)*cos(e3)*cos(e4)*cos(e5)*cos(e6)^2*sin(e5) - I6yy*cos(e2)*cos(e3)*cos(e4)*cos(e5)*cos(e6)^2*sin(e5) - a3*m5*x5*cos(e2)*cos(e4)*cos(e5)*sin(e3) - a3*m5*x5*cos(e3)*cos(e4)*cos(e5)*sin(e2) - a2*m6*x6*cos(e4)*cos(e5)*cos(e6)*sin(e2) + d4*m5*y5*cos(e2)*cos(e3)*cos(e4)*sin(e5) + d4*m6*y6*cos(e2)*cos(e3)*cos(e6)*sin(e4) + d4*m6*z6*cos(e2)*cos(e3)*cos(e4)*sin(e5) + m6*x6*z6*cos(e2)*cos(e3)*cos(e4)*cos(e6) + a3*m5*y5*cos(e2)*cos(e4)*sin(e3)*sin(e5) + a3*m5*y5*cos(e3)*cos(e4)*sin(e2)*sin(e5) + a3*m6*y6*cos(e2)*cos(e6)*sin(e3)*sin(e4) + a3*m6*y6*cos(e3)*cos(e6)*sin(e2)*sin(e4) + a2*m6*y6*cos(e4)*cos(e5)*sin(e2)*sin(e6) + a3*m6*z6*cos(e2)*cos(e4)*sin(e3)*sin(e5) + a3*m6*z6*cos(e3)*cos(e4)*sin(e2)*sin(e5) + d4*m5*x5*cos(e4)*cos(e5)*sin(e2)*sin(e3) + d4*m6*x6*cos(e2)*cos(e3)*sin(e4)*sin(e6) - I6xx*cos(e4)*cos(e5)*cos(e6)^2*sin(e2)*sin(e3)*sin(e5) + I6yy*cos(e4)*cos(e5)*cos(e6)^2*sin(e2)*sin(e3)*sin(e5) - m5*y5*z5*cos(e2)*cos(e3)*cos(e5)*sin(e4) - m6*y6*z6*cos(e2)*cos(e3)*cos(e4)*sin(e6) + a3*m6*x6*cos(e2)*sin(e3)*sin(e4)*sin(e6) + a3*m6*x6*cos(e3)*sin(e2)*sin(e4)*sin(e6) - d4*m5*y5*cos(e4)*sin(e2)*sin(e3)*sin(e5) - d4*m6*y6*cos(e6)*sin(e2)*sin(e3)*sin(e4) - d4*m6*z6*cos(e4)*sin(e2)*sin(e3)*sin(e5) + 2*m5*x5*y5*cos(e2)*cos(e5)*sin(e3)*sin(e5) + 2*m5*x5*y5*cos(e3)*cos(e5)*sin(e2)*sin(e5) - m6*x6*y6*cos(e2)*cos(e3)*sin(e4)*sin(e5) - 2*m6*x6*y6*cos(e2)*cos(e6)*sin(e3)*sin(e6) - 2*m6*x6*y6*cos(e3)*cos(e6)*sin(e2)*sin(e6) - 2*m6*x6*z6*cos(e2)*cos(e3)*cos(e4)*cos(e5)^2*cos(e6) + 2*m6*y6*z6*cos(e2)*cos(e3)*cos(e4)*cos(e5)^2*sin(e6) + 2*m6*x6*y6*cos(e2)*cos(e3)*cos(e6)^2*sin(e4)*sin(e5) + 2*m6*x6*y6*cos(e2)*cos(e5)^2*cos(e6)*sin(e3)*sin(e6) + 2*m6*x6*y6*cos(e3)*cos(e5)^2*cos(e6)*sin(e2)*sin(e6) + 2*m6*x6*z6*cos(e4)*cos(e5)^2*cos(e6)*sin(e2)*sin(e3) - 2*m6*y6*z6*cos(e4)*cos(e5)^2*sin(e2)*sin(e3)*sin(e6) - 2*m6*x6*y6*cos(e6)^2*sin(e2)*sin(e3)*sin(e4)*sin(e5) + m6*x6^2*cos(e2)*cos(e3)*cos(e6)*sin(e4)*sin(e5)*sin(e6) - m6*y6^2*cos(e2)*cos(e3)*cos(e6)*sin(e4)*sin(e5)*sin(e6) - d4*m6*x6*cos(e2)*cos(e3)*cos(e4)*cos(e5)*cos(e6) - a3*m6*x6*cos(e2)*cos(e4)*cos(e5)*cos(e6)*sin(e3) - a3*m6*x6*cos(e3)*cos(e4)*cos(e5)*cos(e6)*sin(e2) + d4*m6*y6*cos(e2)*cos(e3)*cos(e4)*cos(e5)*sin(e6) - m6*x6^2*cos(e6)*sin(e2)*sin(e3)*sin(e4)*sin(e5)*sin(e6) + m6*y6^2*cos(e6)*sin(e2)*sin(e3)*sin(e4)*sin(e5)*sin(e6) + a3*m6*y6*cos(e2)*cos(e4)*cos(e5)*sin(e3)*sin(e6) + a3*m6*y6*cos(e3)*cos(e4)*cos(e5)*sin(e2)*sin(e6) + d4*m6*x6*cos(e4)*cos(e5)*cos(e6)*sin(e2)*sin(e3) + m6*y6*z6*cos(e2)*cos(e3)*cos(e5)*cos(e6)*sin(e4) - d4*m6*y6*cos(e4)*cos(e5)*sin(e2)*sin(e3)*sin(e6) - m6*x6^2*cos(e2)*cos(e3)*cos(e4)*cos(e5)*cos(e6)^2*sin(e5) + m6*y6^2*cos(e2)*cos(e3)*cos(e4)*cos(e5)*cos(e6)^2*sin(e5) + m6*x6*z6*cos(e2)*cos(e3)*cos(e5)*sin(e4)*sin(e6) + 2*m6*x6*z6*cos(e2)*cos(e5)*cos(e6)*sin(e3)*sin(e5) + 2*m6*x6*z6*cos(e3)*cos(e5)*cos(e6)*sin(e2)*sin(e5) - m6*y6*z6*cos(e5)*cos(e6)*sin(e2)*sin(e3)*sin(e4) - 2*m6*y6*z6*cos(e2)*cos(e5)*sin(e3)*sin(e5)*sin(e6) - 2*m6*y6*z6*cos(e3)*cos(e5)*sin(e2)*sin(e5)*sin(e6) + m6*x6^2*cos(e4)*cos(e5)*cos(e6)^2*sin(e2)*sin(e3)*sin(e5) - m6*y6^2*cos(e4)*cos(e5)*cos(e6)^2*sin(e2)*sin(e3)*sin(e5) - m6*x6*z6*cos(e5)*sin(e2)*sin(e3)*sin(e4)*sin(e6) + 2*m6*x6*y6*cos(e2)*cos(e3)*cos(e4)*cos(e5)*cos(e6)*sin(e5)*sin(e6) - 2*m6*x6*y6*cos(e4)*cos(e5)*cos(e6)*sin(e2)*sin(e3)*sin(e5)*sin(e6),I6xx*cos(e2)*cos(e3)*sin(e4) + I5zz*cos(e2)*cos(e3)*sin(e4) - I6xx*sin(e2)*sin(e3)*sin(e4) - I5zz*sin(e2)*sin(e3)*sin(e4) + m5*x5^2*cos(e2)*cos(e3)*sin(e4) + m5*y5^2*cos(e2)*cos(e3)*sin(e4) + m6*y6^2*cos(e2)*cos(e3)*sin(e4) + m6*z6^2*cos(e2)*cos(e3)*sin(e4) - m5*x5^2*sin(e2)*sin(e3)*sin(e4) - m5*y5^2*sin(e2)*sin(e3)*sin(e4) - m6*y6^2*sin(e2)*sin(e3)*sin(e4) - m6*z6^2*sin(e2)*sin(e3)*sin(e4) - I6xx*cos(e2)*cos(e3)*cos(e6)^2*sin(e4) + I6yy*cos(e2)*cos(e3)*cos(e6)^2*sin(e4) + a1*m5*y5*cos(e5)*sin(e4) + a1*m6*z6*cos(e5)*sin(e4) + a1*m5*x5*sin(e4)*sin(e5) + I6xx*cos(e6)^2*sin(e2)*sin(e3)*sin(e4) - I6yy*cos(e6)^2*sin(e2)*sin(e3)*sin(e4) + a1*m6*x6*cos(e6)*sin(e4)*sin(e5) + a2*m5*y5*cos(e5)*sin(e2)*sin(e4) + a2*m6*z6*cos(e5)*sin(e2)*sin(e4) + m5*y5*z5*cos(e2)*cos(e5)*sin(e3) + m5*y5*z5*cos(e3)*cos(e5)*sin(e2) + a2*m5*x5*sin(e2)*sin(e4)*sin(e5) - a1*m6*y6*sin(e4)*sin(e5)*sin(e6) + m6*x6^2*cos(e2)*cos(e3)*cos(e6)^2*sin(e4) - m6*y6^2*cos(e2)*cos(e3)*cos(e6)^2*sin(e4) + m6*x6*y6*cos(e2)*sin(e3)*sin(e5) + m6*x6*y6*cos(e3)*sin(e2)*sin(e5) + m5*x5*z5*cos(e2)*sin(e3)*sin(e5) + m5*x5*z5*cos(e3)*sin(e2)*sin(e5) - m6*x6^2*cos(e6)^2*sin(e2)*sin(e3)*sin(e4) + m6*y6^2*cos(e6)^2*sin(e2)*sin(e3)*sin(e4) + I6xx*cos(e2)*cos(e6)*sin(e3)*sin(e5)*sin(e6) + I6xx*cos(e3)*cos(e6)*sin(e2)*sin(e5)*sin(e6) - I6yy*cos(e2)*cos(e6)*sin(e3)*sin(e5)*sin(e6) - I6yy*cos(e3)*cos(e6)*sin(e2)*sin(e5)*sin(e6) + m5*x5*z5*cos(e4)*cos(e5)*sin(e2)*sin(e3) - m6*x6*z6*cos(e2)*cos(e5)*sin(e3)*sin(e6) - m6*x6*z6*cos(e3)*cos(e5)*sin(e2)*sin(e6) - a2*m6*y6*sin(e2)*sin(e4)*sin(e5)*sin(e6) - d4*m5*x5*sin(e2)*sin(e3)*sin(e4)*sin(e5) - m5*y5*z5*cos(e4)*sin(e2)*sin(e3)*sin(e5) - 2*m6*x6*y6*cos(e2)*cos(e6)^2*sin(e3)*sin(e5) - 2*m6*x6*y6*cos(e3)*cos(e6)^2*sin(e2)*sin(e5) - I6xx*cos(e2)*cos(e3)*cos(e4)*cos(e5)*cos(e6)*sin(e6) + I6yy*cos(e2)*cos(e3)*cos(e4)*cos(e5)*cos(e6)*sin(e6) + I6xx*cos(e4)*cos(e5)*cos(e6)*sin(e2)*sin(e3)*sin(e6) - I6yy*cos(e4)*cos(e5)*cos(e6)*sin(e2)*sin(e3)*sin(e6) - m6*x6^2*cos(e2)*cos(e6)*sin(e3)*sin(e5)*sin(e6) - m6*x6^2*cos(e3)*cos(e6)*sin(e2)*sin(e5)*sin(e6) + m6*y6^2*cos(e2)*cos(e6)*sin(e3)*sin(e5)*sin(e6) + m6*y6^2*cos(e3)*cos(e6)*sin(e2)*sin(e5)*sin(e6) + d4*m5*y5*cos(e2)*cos(e3)*cos(e5)*sin(e4) + d4*m6*z6*cos(e2)*cos(e3)*cos(e5)*sin(e4) - m6*x6*y6*cos(e2)*cos(e3)*cos(e4)*cos(e5) - m5*x5*z5*cos(e2)*cos(e3)*cos(e4)*cos(e5) + a3*m5*y5*cos(e2)*cos(e5)*sin(e3)*sin(e4) + a3*m5*y5*cos(e3)*cos(e5)*sin(e2)*sin(e4) + a3*m6*z6*cos(e2)*cos(e5)*sin(e3)*sin(e4) + a3*m6*z6*cos(e3)*cos(e5)*sin(e2)*sin(e4) + d4*m5*x5*cos(e2)*cos(e3)*sin(e4)*sin(e5) + m5*y5*z5*cos(e2)*cos(e3)*cos(e4)*sin(e5) - m6*y6*z6*cos(e2)*cos(e5)*cos(e6)*sin(e3) - m6*y6*z6*cos(e3)*cos(e5)*cos(e6)*sin(e2) + a3*m5*x5*cos(e2)*sin(e3)*sin(e4)*sin(e5) + a3*m5*x5*cos(e3)*sin(e2)*sin(e4)*sin(e5) + a2*m6*x6*cos(e6)*sin(e2)*sin(e4)*sin(e5) - d4*m5*y5*cos(e5)*sin(e2)*sin(e3)*sin(e4) - d4*m6*z6*cos(e5)*sin(e2)*sin(e3)*sin(e4) + m6*x6*y6*cos(e4)*cos(e5)*sin(e2)*sin(e3) + 2*m6*x6*y6*cos(e2)*cos(e3)*cos(e4)*cos(e5)*cos(e6)^2 - 2*m6*x6*y6*cos(e4)*cos(e5)*cos(e6)^2*sin(e2)*sin(e3) + m6*x6^2*cos(e2)*cos(e3)*cos(e4)*cos(e5)*cos(e6)*sin(e6) - m6*y6^2*cos(e2)*cos(e3)*cos(e4)*cos(e5)*cos(e6)*sin(e6) - m6*x6^2*cos(e4)*cos(e5)*cos(e6)*sin(e2)*sin(e3)*sin(e6) + m6*y6^2*cos(e4)*cos(e5)*cos(e6)*sin(e2)*sin(e3)*sin(e6) + d4*m6*x6*cos(e2)*cos(e3)*cos(e6)*sin(e4)*sin(e5) - m6*y6*z6*cos(e2)*cos(e3)*cos(e4)*cos(e6)*sin(e5) + a3*m6*x6*cos(e2)*cos(e6)*sin(e3)*sin(e4)*sin(e5) + a3*m6*x6*cos(e3)*cos(e6)*sin(e2)*sin(e4)*sin(e5) - d4*m6*y6*cos(e2)*cos(e3)*sin(e4)*sin(e5)*sin(e6) - 2*m6*x6*y6*cos(e2)*cos(e3)*cos(e6)*sin(e4)*sin(e6) - m6*x6*z6*cos(e2)*cos(e3)*cos(e4)*sin(e5)*sin(e6) - a3*m6*y6*cos(e2)*sin(e3)*sin(e4)*sin(e5)*sin(e6) - a3*m6*y6*cos(e3)*sin(e2)*sin(e4)*sin(e5)*sin(e6) - d4*m6*x6*cos(e6)*sin(e2)*sin(e3)*sin(e4)*sin(e5) + m6*y6*z6*cos(e4)*cos(e6)*sin(e2)*sin(e3)*sin(e5) + d4*m6*y6*sin(e2)*sin(e3)*sin(e4)*sin(e5)*sin(e6) + 2*m6*x6*y6*cos(e6)*sin(e2)*sin(e3)*sin(e4)*sin(e6) + m6*x6*z6*cos(e4)*sin(e2)*sin(e3)*sin(e5)*sin(e6),a1*m6*y6*cos(e4)*sin(e6) - I6zz*cos(e3)*cos(e5)*sin(e2) - m6*x6^2*cos(e2)*cos(e5)*sin(e3) - m6*x6^2*cos(e3)*cos(e5)*sin(e2) - m6*y6^2*cos(e2)*cos(e5)*sin(e3) - m6*y6^2*cos(e3)*cos(e5)*sin(e2) - a1*m6*x6*cos(e4)*cos(e6) - I6zz*cos(e2)*cos(e5)*sin(e3) - I6zz*cos(e2)*cos(e3)*cos(e4)*sin(e5) + I6zz*cos(e4)*sin(e2)*sin(e3)*sin(e5) - a2*m6*x6*cos(e4)*cos(e6)*sin(e2) + a1*m6*y6*cos(e5)*cos(e6)*sin(e4) + a1*m6*x6*cos(e5)*sin(e4)*sin(e6) + a2*m6*y6*cos(e4)*sin(e2)*sin(e6) - m6*x6^2*cos(e2)*cos(e3)*cos(e4)*sin(e5) - m6*y6^2*cos(e2)*cos(e3)*cos(e4)*sin(e5) + m6*x6^2*cos(e4)*sin(e2)*sin(e3)*sin(e5) + m6*y6^2*cos(e4)*sin(e2)*sin(e3)*sin(e5) + m6*x6*z6*cos(e2)*cos(e3)*sin(e4)*sin(e6) + m6*x6*z6*cos(e2)*cos(e6)*sin(e3)*sin(e5) + m6*x6*z6*cos(e3)*cos(e6)*sin(e2)*sin(e5) - m6*y6*z6*cos(e6)*sin(e2)*sin(e3)*sin(e4) - m6*y6*z6*cos(e2)*sin(e3)*sin(e5)*sin(e6) - m6*y6*z6*cos(e3)*sin(e2)*sin(e5)*sin(e6) - m6*x6*z6*sin(e2)*sin(e3)*sin(e4)*sin(e6) - d4*m6*x6*cos(e2)*cos(e3)*cos(e4)*cos(e6) - a3*m6*x6*cos(e2)*cos(e4)*cos(e6)*sin(e3) - a3*m6*x6*cos(e3)*cos(e4)*cos(e6)*sin(e2) + d4*m6*y6*cos(e2)*cos(e3)*cos(e4)*sin(e6) + a3*m6*y6*cos(e2)*cos(e4)*sin(e3)*sin(e6) + a3*m6*y6*cos(e3)*cos(e4)*sin(e2)*sin(e6) + a2*m6*y6*cos(e5)*cos(e6)*sin(e2)*sin(e4) + d4*m6*x6*cos(e4)*cos(e6)*sin(e2)*sin(e3) + m6*y6*z6*cos(e2)*cos(e3)*cos(e6)*sin(e4) + a2*m6*x6*cos(e5)*sin(e2)*sin(e4)*sin(e6) - d4*m6*y6*cos(e4)*sin(e2)*sin(e3)*sin(e6) + d4*m6*y6*cos(e2)*cos(e3)*cos(e5)*cos(e6)*sin(e4) - m6*x6*z6*cos(e2)*cos(e3)*cos(e4)*cos(e5)*cos(e6) + a3*m6*y6*cos(e2)*cos(e5)*cos(e6)*sin(e3)*sin(e4) + a3*m6*y6*cos(e3)*cos(e5)*cos(e6)*sin(e2)*sin(e4) + d4*m6*x6*cos(e2)*cos(e3)*cos(e5)*sin(e4)*sin(e6) + m6*y6*z6*cos(e2)*cos(e3)*cos(e4)*cos(e5)*sin(e6) + a3*m6*x6*cos(e2)*cos(e5)*sin(e3)*sin(e4)*sin(e6) + a3*m6*x6*cos(e3)*cos(e5)*sin(e2)*sin(e4)*sin(e6) - d4*m6*y6*cos(e5)*cos(e6)*sin(e2)*sin(e3)*sin(e4) + m6*x6*z6*cos(e4)*cos(e5)*cos(e6)*sin(e2)*sin(e3) - d4*m6*x6*cos(e5)*sin(e2)*sin(e3)*sin(e4)*sin(e6) - m6*y6*z6*cos(e4)*cos(e5)*sin(e2)*sin(e3)*sin(e6);
 m2*y2*z2*sin(e2) - m2*x2*z2*cos(e2) - a2*m3*z3*cos(e2) + a2*m4*y4*cos(e2)*cos(e4) - a2*m5*z5*cos(e2)*cos(e4) + a2*m4*x4*cos(e2)*sin(e4) - m4*x4*y4*cos(e2)*cos(e3) - m3*x3*z3*cos(e2)*cos(e3) + m3*y3*z3*cos(e2)*sin(e3) + m3*y3*z3*cos(e3)*sin(e2) + m4*x4*y4*sin(e2)*sin(e3) + m3*x3*z3*sin(e2)*sin(e3) - I4xx*cos(e2)*cos(e3)*cos(e4)*sin(e4) + I6xx*cos(e2)*cos(e3)*cos(e4)*sin(e4) + I4yy*cos(e2)*cos(e3)*cos(e4)*sin(e4) - I5yy*cos(e2)*cos(e3)*cos(e4)*sin(e4) + I5zz*cos(e2)*cos(e3)*cos(e4)*sin(e4) - I6zz*cos(e2)*cos(e3)*cos(e4)*sin(e4) + I4xx*cos(e4)*sin(e2)*sin(e3)*sin(e4) - I6xx*cos(e4)*sin(e2)*sin(e3)*sin(e4) - I4yy*cos(e4)*sin(e2)*sin(e3)*sin(e4) + I5yy*cos(e4)*sin(e2)*sin(e3)*sin(e4) - I5zz*cos(e4)*sin(e2)*sin(e3)*sin(e4) + I6zz*cos(e4)*sin(e2)*sin(e3)*sin(e4) - a3*m5*z5*cos(e2)*cos(e3)*cos(e4) - I5xx*cos(e2)*cos(e3)*cos(e4)*cos(e5)^2*sin(e4) - I6xx*cos(e2)*cos(e3)*cos(e4)*cos(e6)^2*sin(e4) + I5yy*cos(e2)*cos(e3)*cos(e4)*cos(e5)^2*sin(e4) - I6yy*cos(e2)*cos(e3)*cos(e4)*cos(e5)^2*sin(e4) + I6yy*cos(e2)*cos(e3)*cos(e4)*cos(e6)^2*sin(e4) + I6zz*cos(e2)*cos(e3)*cos(e4)*cos(e5)^2*sin(e4) + a3*m4*x4*cos(e2)*cos(e3)*sin(e4) + a2*m5*x5*cos(e2)*cos(e5)*sin(e4) + a2*m6*x6*cos(e2)*cos(e4)*sin(e6) - d4*m4*y4*cos(e2)*cos(e4)*sin(e3) - d4*m4*y4*cos(e3)*cos(e4)*sin(e2) + d4*m5*z5*cos(e2)*cos(e4)*sin(e3) + d4*m5*z5*cos(e3)*cos(e4)*sin(e2) + m6*x6*y6*cos(e2)*cos(e3)*cos(e5) + m5*x5*z5*cos(e2)*cos(e3)*cos(e5) - a3*m4*y4*cos(e4)*sin(e2)*sin(e3) - a2*m5*y5*cos(e2)*sin(e4)*sin(e5) + a3*m5*z5*cos(e4)*sin(e2)*sin(e3) - a2*m6*z6*cos(e2)*sin(e4)*sin(e5) - d4*m4*x4*cos(e2)*sin(e3)*sin(e4) - d4*m4*x4*cos(e3)*sin(e2)*sin(e4) + I5xx*cos(e4)*cos(e5)^2*sin(e2)*sin(e3)*sin(e4) + I6xx*cos(e4)*cos(e6)^2*sin(e2)*sin(e3)*sin(e4) - I5yy*cos(e4)*cos(e5)^2*sin(e2)*sin(e3)*sin(e4) + I6yy*cos(e4)*cos(e5)^2*sin(e2)*sin(e3)*sin(e4) - I6yy*cos(e4)*cos(e6)^2*sin(e2)*sin(e3)*sin(e4) - I6zz*cos(e4)*cos(e5)^2*sin(e2)*sin(e3)*sin(e4) - m4*y4*z4*cos(e2)*cos(e4)*sin(e3) - m4*y4*z4*cos(e3)*cos(e4)*sin(e2) - m5*y5*z5*cos(e2)*cos(e3)*sin(e5) - a3*m4*x4*sin(e2)*sin(e3)*sin(e4) + m5*x5*y5*cos(e2)*sin(e3)*sin(e4) + m5*x5*y5*cos(e3)*sin(e2)*sin(e4) - m6*x6*y6*cos(e5)*sin(e2)*sin(e3) - m4*x4*z4*cos(e2)*sin(e3)*sin(e4) - m4*x4*z4*cos(e3)*sin(e2)*sin(e4) - m5*x5*z5*cos(e5)*sin(e2)*sin(e3) + m5*y5*z5*sin(e2)*sin(e3)*sin(e5) + 2*m4*x4*y4*cos(e2)*cos(e3)*cos(e4)^2 - 2*m4*x4*y4*cos(e4)^2*sin(e2)*sin(e3) + I6xx*cos(e2)*cos(e3)*cos(e5)*cos(e6)*sin(e6) - I6yy*cos(e2)*cos(e3)*cos(e5)*cos(e6)*sin(e6) + I5xx*cos(e2)*cos(e5)*sin(e3)*sin(e4)*sin(e5) + I5xx*cos(e3)*cos(e5)*sin(e2)*sin(e4)*sin(e5) - I6xx*cos(e5)*cos(e6)*sin(e2)*sin(e3)*sin(e6) - I5yy*cos(e2)*cos(e5)*sin(e3)*sin(e4)*sin(e5) - I5yy*cos(e3)*cos(e5)*sin(e2)*sin(e4)*sin(e5) + I6yy*cos(e2)*cos(e5)*sin(e3)*sin(e4)*sin(e5) + I6yy*cos(e3)*cos(e5)*sin(e2)*sin(e4)*sin(e5) + I6yy*cos(e5)*cos(e6)*sin(e2)*sin(e3)*sin(e6) - I6zz*cos(e2)*cos(e5)*sin(e3)*sin(e4)*sin(e5) - I6zz*cos(e3)*cos(e5)*sin(e2)*sin(e4)*sin(e5) + m4*x4^2*cos(e2)*cos(e3)*cos(e4)*sin(e4) - m6*x6^2*cos(e2)*cos(e3)*cos(e4)*sin(e4) - m4*y4^2*cos(e2)*cos(e3)*cos(e4)*sin(e4) + m5*y5^2*cos(e2)*cos(e3)*cos(e4)*sin(e4) - m5*z5^2*cos(e2)*cos(e3)*cos(e4)*sin(e4) + m6*z6^2*cos(e2)*cos(e3)*cos(e4)*sin(e4) - m4*x4^2*cos(e4)*sin(e2)*sin(e3)*sin(e4) + m6*x6^2*cos(e4)*sin(e2)*sin(e3)*sin(e4) + m4*y4^2*cos(e4)*sin(e2)*sin(e3)*sin(e4) - m5*y5^2*cos(e4)*sin(e2)*sin(e3)*sin(e4) + m5*z5^2*cos(e4)*sin(e2)*sin(e3)*sin(e4) - m6*z6^2*cos(e4)*sin(e2)*sin(e3)*sin(e4) + a3*m4*y4*cos(e2)*cos(e3)*cos(e4) + a2*m6*y6*cos(e2)*cos(e4)*cos(e6) + m5*x5*z5*cos(e2)*cos(e4)*sin(e3)*sin(e5) + m5*x5*z5*cos(e3)*cos(e4)*sin(e2)*sin(e5) + m6*x6*z6*cos(e2)*cos(e6)*sin(e3)*sin(e4) + m6*x6*z6*cos(e3)*cos(e6)*sin(e2)*sin(e4) + m6*x6*z6*cos(e2)*cos(e3)*sin(e5)*sin(e6) + a3*m5*y5*sin(e2)*sin(e3)*sin(e4)*sin(e5) + a3*m6*z6*sin(e2)*sin(e3)*sin(e4)*sin(e5) - m6*y6*z6*cos(e2)*sin(e3)*sin(e4)*sin(e6) - m6*y6*z6*cos(e3)*sin(e2)*sin(e4)*sin(e6) - m6*y6*z6*cos(e6)*sin(e2)*sin(e3)*sin(e5) - m5*x5^2*cos(e4)*cos(e5)^2*sin(e2)*sin(e3)*sin(e4) - m6*x6^2*cos(e4)*cos(e6)^2*sin(e2)*sin(e3)*sin(e4) + m5*y5^2*cos(e4)*cos(e5)^2*sin(e2)*sin(e3)*sin(e4) - m6*y6^2*cos(e4)*cos(e5)^2*sin(e2)*sin(e3)*sin(e4) + m6*y6^2*cos(e4)*cos(e6)^2*sin(e2)*sin(e3)*sin(e4) + m6*z6^2*cos(e4)*cos(e5)^2*sin(e2)*sin(e3)*sin(e4) - m6*x6*z6*sin(e2)*sin(e3)*sin(e5)*sin(e6) - I6xx*cos(e2)*cos(e3)*cos(e4)*cos(e5)^2*cos(e6)^2*sin(e4) + I6yy*cos(e2)*cos(e3)*cos(e4)*cos(e5)^2*cos(e6)^2*sin(e4) - 2*m6*x6*y6*cos(e2)*cos(e3)*cos(e4)^2*cos(e5) - 2*m6*x6*y6*cos(e2)*cos(e3)*cos(e5)*cos(e6)^2 - 2*m5*x5*z5*cos(e2)*cos(e3)*cos(e4)^2*cos(e5) + I6xx*cos(e4)*cos(e5)^2*cos(e6)^2*sin(e2)*sin(e3)*sin(e4) - I6yy*cos(e4)*cos(e5)^2*cos(e6)^2*sin(e2)*sin(e3)*sin(e4) + 2*m5*y5*z5*cos(e2)*cos(e3)*cos(e4)^2*sin(e5) - 2*m5*x5*y5*cos(e2)*cos(e5)^2*sin(e3)*sin(e4) - 2*m5*x5*y5*cos(e3)*cos(e5)^2*sin(e2)*sin(e4) + 2*m6*x6*y6*cos(e4)^2*cos(e5)*sin(e2)*sin(e3) + 2*m6*x6*y6*cos(e5)*cos(e6)^2*sin(e2)*sin(e3) + 2*m5*x5*z5*cos(e4)^2*cos(e5)*sin(e2)*sin(e3) - 2*m5*y5*z5*cos(e4)^2*sin(e2)*sin(e3)*sin(e5) + I6xx*cos(e2)*cos(e4)*cos(e6)*sin(e3)*sin(e5)*sin(e6) + I6xx*cos(e3)*cos(e4)*cos(e6)*sin(e2)*sin(e5)*sin(e6) - I6yy*cos(e2)*cos(e4)*cos(e6)*sin(e3)*sin(e5)*sin(e6) - I6yy*cos(e3)*cos(e4)*cos(e6)*sin(e2)*sin(e5)*sin(e6) - m6*x6^2*cos(e2)*cos(e3)*cos(e5)*cos(e6)*sin(e6) + m6*y6^2*cos(e2)*cos(e3)*cos(e5)*cos(e6)*sin(e6) - m5*x5^2*cos(e2)*cos(e5)*sin(e3)*sin(e4)*sin(e5) - m5*x5^2*cos(e3)*cos(e5)*sin(e2)*sin(e4)*sin(e5) + m6*x6^2*cos(e5)*cos(e6)*sin(e2)*sin(e3)*sin(e6) + m5*y5^2*cos(e2)*cos(e5)*sin(e3)*sin(e4)*sin(e5) + m5*y5^2*cos(e3)*cos(e5)*sin(e2)*sin(e4)*sin(e5) - m6*y6^2*cos(e2)*cos(e5)*sin(e3)*sin(e4)*sin(e5) - m6*y6^2*cos(e3)*cos(e5)*sin(e2)*sin(e4)*sin(e5) - m6*y6^2*cos(e5)*cos(e6)*sin(e2)*sin(e3)*sin(e6) + m6*z6^2*cos(e2)*cos(e5)*sin(e3)*sin(e4)*sin(e5) + m6*z6^2*cos(e3)*cos(e5)*sin(e2)*sin(e4)*sin(e5) + a3*m6*y6*cos(e2)*cos(e3)*cos(e4)*cos(e6) - 2*I6xx*cos(e2)*cos(e3)*cos(e4)^2*cos(e5)*cos(e6)*sin(e6) + 2*I6yy*cos(e2)*cos(e3)*cos(e4)^2*cos(e5)*cos(e6)*sin(e6) + a3*m5*x5*cos(e2)*cos(e3)*cos(e5)*sin(e4) + a3*m6*x6*cos(e2)*cos(e3)*cos(e4)*sin(e6) + a2*m6*x6*cos(e2)*cos(e5)*cos(e6)*sin(e4) - d4*m6*y6*cos(e2)*cos(e4)*cos(e6)*sin(e3) - d4*m6*y6*cos(e3)*cos(e4)*cos(e6)*sin(e2) - a3*m5*y5*cos(e2)*cos(e3)*sin(e4)*sin(e5) - a3*m6*y6*cos(e4)*cos(e6)*sin(e2)*sin(e3) - a2*m6*y6*cos(e2)*cos(e5)*sin(e4)*sin(e6) - a3*m6*z6*cos(e2)*cos(e3)*sin(e4)*sin(e5) - d4*m5*x5*cos(e2)*cos(e5)*sin(e3)*sin(e4) - d4*m5*x5*cos(e3)*cos(e5)*sin(e2)*sin(e4) - d4*m6*x6*cos(e2)*cos(e4)*sin(e3)*sin(e6) - d4*m6*x6*cos(e3)*cos(e4)*sin(e2)*sin(e6) + I6xx*cos(e2)*cos(e5)*cos(e6)^2*sin(e3)*sin(e4)*sin(e5) + I6xx*cos(e3)*cos(e5)*cos(e6)^2*sin(e2)*sin(e4)*sin(e5) + 2*I6xx*cos(e4)^2*cos(e5)*cos(e6)*sin(e2)*sin(e3)*sin(e6) - I6yy*cos(e2)*cos(e5)*cos(e6)^2*sin(e3)*sin(e4)*sin(e5) - I6yy*cos(e3)*cos(e5)*cos(e6)^2*sin(e2)*sin(e4)*sin(e5) - 2*I6yy*cos(e4)^2*cos(e5)*cos(e6)*sin(e2)*sin(e3)*sin(e6) + m5*y5*z5*cos(e2)*cos(e4)*cos(e5)*sin(e3) + m5*y5*z5*cos(e3)*cos(e4)*cos(e5)*sin(e2) + m6*y6*z6*cos(e2)*cos(e3)*cos(e6)*sin(e5) - a3*m5*x5*cos(e5)*sin(e2)*sin(e3)*sin(e4) - a3*m6*x6*cos(e4)*sin(e2)*sin(e3)*sin(e6) + d4*m5*y5*cos(e2)*sin(e3)*sin(e4)*sin(e5) + d4*m5*y5*cos(e3)*sin(e2)*sin(e4)*sin(e5) + d4*m6*z6*cos(e2)*sin(e3)*sin(e4)*sin(e5) + d4*m6*z6*cos(e3)*sin(e2)*sin(e4)*sin(e5) + m5*x5^2*cos(e2)*cos(e3)*cos(e4)*cos(e5)^2*sin(e4) + m6*x6^2*cos(e2)*cos(e3)*cos(e4)*cos(e6)^2*sin(e4) - m5*y5^2*cos(e2)*cos(e3)*cos(e4)*cos(e5)^2*sin(e4) + m6*y6^2*cos(e2)*cos(e3)*cos(e4)*cos(e5)^2*sin(e4) - m6*y6^2*cos(e2)*cos(e3)*cos(e4)*cos(e6)^2*sin(e4) + m6*x6*y6*cos(e2)*cos(e4)*sin(e3)*sin(e5) + m6*x6*y6*cos(e3)*cos(e4)*sin(e2)*sin(e5) - m6*z6^2*cos(e2)*cos(e3)*cos(e4)*cos(e5)^2*sin(e4) - 2*m6*y6*z6*cos(e2)*cos(e3)*cos(e4)^2*cos(e6)*sin(e5) + m6*x6^2*cos(e2)*cos(e3)*cos(e4)*cos(e5)^2*cos(e6)^2*sin(e4) - m6*y6^2*cos(e2)*cos(e3)*cos(e4)*cos(e5)^2*cos(e6)^2*sin(e4) - 2*m6*x6*y6*cos(e2)*cos(e4)*cos(e6)^2*sin(e3)*sin(e5) - 2*m6*x6*y6*cos(e3)*cos(e4)*cos(e6)^2*sin(e2)*sin(e5) - 2*m6*x6*z6*cos(e2)*cos(e3)*cos(e4)^2*sin(e5)*sin(e6) - 2*m6*x6*z6*cos(e2)*cos(e5)^2*cos(e6)*sin(e3)*sin(e4) - 2*m6*x6*z6*cos(e3)*cos(e5)^2*cos(e6)*sin(e2)*sin(e4) + 2*m6*y6*z6*cos(e2)*cos(e5)^2*sin(e3)*sin(e4)*sin(e6) + 2*m6*y6*z6*cos(e3)*cos(e5)^2*sin(e2)*sin(e4)*sin(e6) + 2*m6*y6*z6*cos(e4)^2*cos(e6)*sin(e2)*sin(e3)*sin(e5) - m6*x6^2*cos(e4)*cos(e5)^2*cos(e6)^2*sin(e2)*sin(e3)*sin(e4) + m6*y6^2*cos(e4)*cos(e5)^2*cos(e6)^2*sin(e2)*sin(e3)*sin(e4) + 2*m6*x6*z6*cos(e4)^2*sin(e2)*sin(e3)*sin(e5)*sin(e6) + 4*m6*x6*y6*cos(e2)*cos(e3)*cos(e4)^2*cos(e5)*cos(e6)^2 - m6*x6^2*cos(e2)*cos(e4)*cos(e6)*sin(e3)*sin(e5)*sin(e6) - m6*x6^2*cos(e3)*cos(e4)*cos(e6)*sin(e2)*sin(e5)*sin(e6) - 4*m6*x6*y6*cos(e4)^2*cos(e5)*cos(e6)^2*sin(e2)*sin(e3) + m6*y6^2*cos(e2)*cos(e4)*cos(e6)*sin(e3)*sin(e5)*sin(e6) + m6*y6^2*cos(e3)*cos(e4)*cos(e6)*sin(e2)*sin(e5)*sin(e6) + a3*m6*x6*cos(e2)*cos(e3)*cos(e5)*cos(e6)*sin(e4) - a3*m6*y6*cos(e2)*cos(e3)*cos(e5)*sin(e4)*sin(e6) - d4*m6*x6*cos(e2)*cos(e5)*cos(e6)*sin(e3)*sin(e4) - d4*m6*x6*cos(e3)*cos(e5)*cos(e6)*sin(e2)*sin(e4) - m6*y6*z6*cos(e2)*cos(e4)*cos(e5)*cos(e6)*sin(e3) - m6*y6*z6*cos(e3)*cos(e4)*cos(e5)*cos(e6)*sin(e2) - a3*m6*x6*cos(e5)*cos(e6)*sin(e2)*sin(e3)*sin(e4) + d4*m6*y6*cos(e2)*cos(e5)*sin(e3)*sin(e4)*sin(e6) + d4*m6*y6*cos(e3)*cos(e5)*sin(e2)*sin(e4)*sin(e6) + 2*m6*x6^2*cos(e2)*cos(e3)*cos(e4)^2*cos(e5)*cos(e6)*sin(e6) - 2*m6*y6^2*cos(e2)*cos(e3)*cos(e4)^2*cos(e5)*cos(e6)*sin(e6) - m6*x6*z6*cos(e2)*cos(e4)*cos(e5)*sin(e3)*sin(e6) - m6*x6*z6*cos(e3)*cos(e4)*cos(e5)*sin(e2)*sin(e6) + a3*m6*y6*cos(e5)*sin(e2)*sin(e3)*sin(e4)*sin(e6) - m6*x6^2*cos(e2)*cos(e5)*cos(e6)^2*sin(e3)*sin(e4)*sin(e5) - m6*x6^2*cos(e3)*cos(e5)*cos(e6)^2*sin(e2)*sin(e4)*sin(e5) - 2*m6*x6^2*cos(e4)^2*cos(e5)*cos(e6)*sin(e2)*sin(e3)*sin(e6) + m6*y6^2*cos(e2)*cos(e5)*cos(e6)^2*sin(e3)*sin(e4)*sin(e5) + m6*y6^2*cos(e3)*cos(e5)*cos(e6)^2*sin(e2)*sin(e4)*sin(e5) + 2*m6*y6^2*cos(e4)^2*cos(e5)*cos(e6)*sin(e2)*sin(e3)*sin(e6) - 2*m5*x5*y5*cos(e2)*cos(e3)*cos(e4)*cos(e5)*sin(e4)*sin(e5) - 2*m6*x6*y6*cos(e2)*cos(e3)*cos(e4)*cos(e6)*sin(e4)*sin(e6) + 2*m5*x5*y5*cos(e4)*cos(e5)*sin(e2)*sin(e3)*sin(e4)*sin(e5) + 2*m6*x6*y6*cos(e4)*cos(e6)*sin(e2)*sin(e3)*sin(e4)*sin(e6) - 2*m6*x6*z6*cos(e2)*cos(e3)*cos(e4)*cos(e5)*cos(e6)*sin(e4)*sin(e5) + 2*m6*y6*z6*cos(e2)*cos(e3)*cos(e4)*cos(e5)*sin(e4)*sin(e5)*sin(e6) + 2*m6*x6*y6*cos(e2)*cos(e5)*cos(e6)*sin(e3)*sin(e4)*sin(e5)*sin(e6) + 2*m6*x6*y6*cos(e3)*cos(e5)*cos(e6)*sin(e2)*sin(e4)*sin(e5)*sin(e6) + 2*m6*x6*z6*cos(e4)*cos(e5)*cos(e6)*sin(e2)*sin(e3)*sin(e4)*sin(e5) - 2*m6*y6*z6*cos(e4)*cos(e5)*sin(e2)*sin(e3)*sin(e4)*sin(e5)*sin(e6) - 2*m6*x6*y6*cos(e2)*cos(e3)*cos(e4)*cos(e5)^2*cos(e6)*sin(e4)*sin(e6) + 2*m6*x6*y6*cos(e4)*cos(e5)^2*cos(e6)*sin(e2)*sin(e3)*sin(e4)*sin(e6),I4xx + I5yy + I2zz + I3zz + I6zz + a2^2*m3 + a2^2*m4 + a2^2*m5 + a3^2*m4 + a2^2*m6 + a3^2*m5 + a3^2*m6 + d4^2*m4 + d4^2*m5 + d4^2*m6 + m2*x2^2 + m3*x3^2 + m5*x5^2 + m6*x6^2 + m2*y2^2 + m3*y3^2 + m4*y4^2 + m6*y6^2 + m4*z4^2 + m5*z5^2 - I4xx*cos(e4)^2 + I5xx*cos(e5)^2 + I6xx*cos(e4)^2 + I4yy*cos(e4)^2 - I5yy*cos(e4)^2 - I5yy*cos(e5)^2 + I6yy*cos(e5)^2 + I5zz*cos(e4)^2 - I6zz*cos(e4)^2 - I6zz*cos(e5)^2 + 2*d4*m4*z4 + m4*x4^2*cos(e4)^2 - m5*x5^2*cos(e5)^2 - m6*x6^2*cos(e4)^2 - m4*y4^2*cos(e4)^2 + m5*y5^2*cos(e4)^2 + m5*y5^2*cos(e5)^2 - m6*y6^2*cos(e5)^2 - m5*z5^2*cos(e4)^2 + m6*z6^2*cos(e4)^2 + m6*z6^2*cos(e5)^2 - I5xx*cos(e4)^2*cos(e5)^2 - I6xx*cos(e4)^2*cos(e6)^2 + I6xx*cos(e5)^2*cos(e6)^2 + I5yy*cos(e4)^2*cos(e5)^2 - I6yy*cos(e4)^2*cos(e5)^2 + I6yy*cos(e4)^2*cos(e6)^2 - I6yy*cos(e5)^2*cos(e6)^2 + I6zz*cos(e4)^2*cos(e5)^2 - I6xx*cos(e4)^2*cos(e5)^2*cos(e6)^2 + I6yy*cos(e4)^2*cos(e5)^2*cos(e6)^2 + 2*a2*a3*m4*cos(e3) + 2*a2*a3*m5*cos(e3) + 2*a2*a3*m6*cos(e3) - 2*a2*d4*m4*sin(e3) - 2*a2*d4*m5*sin(e3) - 2*a2*d4*m6*sin(e3) + 2*a2*m3*x3*cos(e3) + 2*a3*m4*x4*cos(e4) + 2*d4*m5*y5*cos(e5) + 2*d4*m6*z6*cos(e5) - 2*a2*m3*y3*sin(e3) - 2*a3*m4*y4*sin(e4) - 2*a2*m4*z4*sin(e3) + 2*a3*m5*z5*sin(e4) + 2*d4*m5*x5*sin(e5) + m5*x5^2*cos(e4)^2*cos(e5)^2 + m6*x6^2*cos(e4)^2*cos(e6)^2 - m6*x6^2*cos(e5)^2*cos(e6)^2 - m5*y5^2*cos(e4)^2*cos(e5)^2 + m6*y6^2*cos(e4)^2*cos(e5)^2 - m6*y6^2*cos(e4)^2*cos(e6)^2 + m6*y6^2*cos(e5)^2*cos(e6)^2 - m4*x4*y4*sin(2*e4) + m5*x5*y5*sin(2*e5) - m6*z6^2*cos(e4)^2*cos(e5)^2 + m6*x6^2*cos(e4)^2*cos(e5)^2*cos(e6)^2 - m6*y6^2*cos(e4)^2*cos(e5)^2*cos(e6)^2 + 2*a2*m4*x4*cos(e3)*cos(e4) + 2*a3*m5*x5*cos(e4)*cos(e5) - 2*a2*m4*y4*cos(e3)*sin(e4) - 2*a2*m5*y5*cos(e5)*sin(e3) - 2*a3*m5*y5*cos(e4)*sin(e5) - 2*a3*m6*y6*cos(e6)*sin(e4) + 2*a2*m5*z5*cos(e3)*sin(e4) - 2*a2*m6*z6*cos(e5)*sin(e3) - 2*a3*m6*z6*cos(e4)*sin(e5) + 2*d4*m6*x6*cos(e6)*sin(e5) - 2*a2*m5*x5*sin(e3)*sin(e5) - 2*a3*m6*x6*sin(e4)*sin(e6) - 2*d4*m6*y6*sin(e5)*sin(e6) - 2*a2*m5*y5*cos(e3)*cos(e4)*sin(e5) - 2*a2*m6*y6*cos(e3)*cos(e6)*sin(e4) - 2*a3*m6*y6*cos(e4)*cos(e5)*sin(e6) - 2*a2*m6*z6*cos(e3)*cos(e4)*sin(e5) - 2*a2*m6*x6*cos(e3)*sin(e4)*sin(e6) - 2*a2*m6*x6*cos(e6)*sin(e3)*sin(e5) + 2*m6*x6*y6*cos(e4)*cos(e5)*sin(e4) + 2*m5*x5*z5*cos(e4)*cos(e5)*sin(e4) + 2*m6*x6*z6*cos(e5)*cos(e6)*sin(e5) + 2*a2*m6*y6*sin(e3)*sin(e5)*sin(e6) - 2*m5*y5*z5*cos(e4)*sin(e4)*sin(e5) - 2*m6*y6*z6*cos(e5)*sin(e5)*sin(e6) - 2*m5*x5*y5*cos(e4)^2*cos(e5)*sin(e5) - 2*m6*x6*y6*cos(e4)^2*cos(e6)*sin(e6) + 2*m6*x6*y6*cos(e5)^2*cos(e6)*sin(e6) + 2*I6xx*cos(e4)*cos(e5)*cos(e6)*sin(e4)*sin(e6) - 2*I6yy*cos(e4)*cos(e5)*cos(e6)*sin(e4)*sin(e6) + 2*a2*m5*x5*cos(e3)*cos(e4)*cos(e5) + 2*a3*m6*x6*cos(e4)*cos(e5)*cos(e6) + 2*m6*y6*z6*cos(e4)*cos(e6)*sin(e4)*sin(e5) + 2*m6*x6*z6*cos(e4)*sin(e4)*sin(e5)*sin(e6) - 4*m6*x6*y6*cos(e4)*cos(e5)*cos(e6)^2*sin(e4) - 2*m6*x6*z6*cos(e4)^2*cos(e5)*cos(e6)*sin(e5) + 2*m6*y6*z6*cos(e4)^2*cos(e5)*sin(e5)*sin(e6) - 2*m6*x6^2*cos(e4)*cos(e5)*cos(e6)*sin(e4)*sin(e6) - 2*m6*x6*y6*cos(e4)^2*cos(e5)^2*cos(e6)*sin(e6) + 2*m6*y6^2*cos(e4)*cos(e5)*cos(e6)*sin(e4)*sin(e6) + 2*a2*m6*x6*cos(e3)*cos(e4)*cos(e5)*cos(e6) - 2*a2*m6*y6*cos(e3)*cos(e4)*cos(e5)*sin(e6),I4xx + I5yy + I3zz + I6zz + a3^2*m4 + a3^2*m5 + a3^2*m6 + d4^2*m4 + d4^2*m5 + d4^2*m6 + m3*x3^2 + m5*x5^2 + m6*x6^2 + m3*y3^2 + m4*y4^2 + m6*y6^2 + m4*z4^2 + m5*z5^2 - I4xx*cos(e4)^2 + I5xx*cos(e5)^2 + I6xx*cos(e4)^2 + I4yy*cos(e4)^2 - I5yy*cos(e4)^2 - I5yy*cos(e5)^2 + I6yy*cos(e5)^2 + I5zz*cos(e4)^2 - I6zz*cos(e4)^2 - I6zz*cos(e5)^2 + 2*d4*m4*z4 + m4*x4^2*cos(e4)^2 - m5*x5^2*cos(e5)^2 - m6*x6^2*cos(e4)^2 - m4*y4^2*cos(e4)^2 + m5*y5^2*cos(e4)^2 + m5*y5^2*cos(e5)^2 - m6*y6^2*cos(e5)^2 - m5*z5^2*cos(e4)^2 + m6*z6^2*cos(e4)^2 + m6*z6^2*cos(e5)^2 - I5xx*cos(e4)^2*cos(e5)^2 - I6xx*cos(e4)^2*cos(e6)^2 + I6xx*cos(e5)^2*cos(e6)^2 + I5yy*cos(e4)^2*cos(e5)^2 - I6yy*cos(e4)^2*cos(e5)^2 + I6yy*cos(e4)^2*cos(e6)^2 - I6yy*cos(e5)^2*cos(e6)^2 + I6zz*cos(e4)^2*cos(e5)^2 - I6xx*cos(e4)^2*cos(e5)^2*cos(e6)^2 + I6yy*cos(e4)^2*cos(e5)^2*cos(e6)^2 + a2*a3*m4*cos(e3) + a2*a3*m5*cos(e3) + a2*a3*m6*cos(e3) - a2*d4*m4*sin(e3) - a2*d4*m5*sin(e3) - a2*d4*m6*sin(e3) + a2*m3*x3*cos(e3) + 2*a3*m4*x4*cos(e4) + 2*d4*m5*y5*cos(e5) + 2*d4*m6*z6*cos(e5) - a2*m3*y3*sin(e3) - 2*a3*m4*y4*sin(e4) - a2*m4*z4*sin(e3) + 2*a3*m5*z5*sin(e4) + 2*d4*m5*x5*sin(e5) + m5*x5^2*cos(e4)^2*cos(e5)^2 + m6*x6^2*cos(e4)^2*cos(e6)^2 - m6*x6^2*cos(e5)^2*cos(e6)^2 - m5*y5^2*cos(e4)^2*cos(e5)^2 + m6*y6^2*cos(e4)^2*cos(e5)^2 - m6*y6^2*cos(e4)^2*cos(e6)^2 + m6*y6^2*cos(e5)^2*cos(e6)^2 - m4*x4*y4*sin(2*e4) + m5*x5*y5*sin(2*e5) - m6*z6^2*cos(e4)^2*cos(e5)^2 + m6*x6^2*cos(e4)^2*cos(e5)^2*cos(e6)^2 - m6*y6^2*cos(e4)^2*cos(e5)^2*cos(e6)^2 + a2*m4*x4*cos(e3)*cos(e4) + 2*a3*m5*x5*cos(e4)*cos(e5) - a2*m4*y4*cos(e3)*sin(e4) - a2*m5*y5*cos(e5)*sin(e3) - 2*a3*m5*y5*cos(e4)*sin(e5) - 2*a3*m6*y6*cos(e6)*sin(e4) + a2*m5*z5*cos(e3)*sin(e4) - a2*m6*z6*cos(e5)*sin(e3) - 2*a3*m6*z6*cos(e4)*sin(e5) + 2*d4*m6*x6*cos(e6)*sin(e5) - a2*m5*x5*sin(e3)*sin(e5) - 2*a3*m6*x6*sin(e4)*sin(e6) - 2*d4*m6*y6*sin(e5)*sin(e6) - a2*m5*y5*cos(e3)*cos(e4)*sin(e5) - a2*m6*y6*cos(e3)*cos(e6)*sin(e4) - 2*a3*m6*y6*cos(e4)*cos(e5)*sin(e6) - a2*m6*z6*cos(e3)*cos(e4)*sin(e5) - a2*m6*x6*cos(e3)*sin(e4)*sin(e6) - a2*m6*x6*cos(e6)*sin(e3)*sin(e5) + 2*m6*x6*y6*cos(e4)*cos(e5)*sin(e4) + 2*m5*x5*z5*cos(e4)*cos(e5)*sin(e4) + 2*m6*x6*z6*cos(e5)*cos(e6)*sin(e5) + a2*m6*y6*sin(e3)*sin(e5)*sin(e6) - 2*m5*y5*z5*cos(e4)*sin(e4)*sin(e5) - 2*m6*y6*z6*cos(e5)*sin(e5)*sin(e6) - 2*m5*x5*y5*cos(e4)^2*cos(e5)*sin(e5) - 2*m6*x6*y6*cos(e4)^2*cos(e6)*sin(e6) + 2*m6*x6*y6*cos(e5)^2*cos(e6)*sin(e6) + 2*I6xx*cos(e4)*cos(e5)*cos(e6)*sin(e4)*sin(e6) - 2*I6yy*cos(e4)*cos(e5)*cos(e6)*sin(e4)*sin(e6) + a2*m5*x5*cos(e3)*cos(e4)*cos(e5) + 2*a3*m6*x6*cos(e4)*cos(e5)*cos(e6) + 2*m6*y6*z6*cos(e4)*cos(e6)*sin(e4)*sin(e5) + 2*m6*x6*z6*cos(e4)*sin(e4)*sin(e5)*sin(e6) - 4*m6*x6*y6*cos(e4)*cos(e5)*cos(e6)^2*sin(e4) - 2*m6*x6*z6*cos(e4)^2*cos(e5)*cos(e6)*sin(e5) + 2*m6*y6*z6*cos(e4)^2*cos(e5)*sin(e5)*sin(e6) - 2*m6*x6^2*cos(e4)*cos(e5)*cos(e6)*sin(e4)*sin(e6) - 2*m6*x6*y6*cos(e4)^2*cos(e5)^2*cos(e6)*sin(e6) + 2*m6*y6^2*cos(e4)*cos(e5)*cos(e6)*sin(e4)*sin(e6) + a2*m6*x6*cos(e3)*cos(e4)*cos(e5)*cos(e6) - a2*m6*y6*cos(e3)*cos(e4)*cos(e5)*sin(e6),I5yy*cos(e5)*sin(e4)*sin(e5) - I5xx*cos(e5)*sin(e4)*sin(e5) - I6yy*cos(e5)*sin(e4)*sin(e5) + I6zz*cos(e5)*sin(e4)*sin(e5) + d4*m4*y4*cos(e4) - d4*m5*z5*cos(e4) + d4*m4*x4*sin(e4) + m4*y4*z4*cos(e4) - m5*x5*y5*sin(e4) + m4*x4*z4*sin(e4) + m5*x5^2*cos(e5)*sin(e4)*sin(e5) - m5*y5^2*cos(e5)*sin(e4)*sin(e5) + m6*y6^2*cos(e5)*sin(e4)*sin(e5) - m6*z6^2*cos(e5)*sin(e4)*sin(e5) + d4*m6*y6*cos(e4)*cos(e6) - a2*m4*y4*cos(e4)*sin(e3) + a2*m5*z5*cos(e4)*sin(e3) + d4*m5*x5*cos(e5)*sin(e4) + d4*m6*x6*cos(e4)*sin(e6) - I6xx*cos(e5)*cos(e6)^2*sin(e4)*sin(e5) + I6yy*cos(e5)*cos(e6)^2*sin(e4)*sin(e5) - m5*y5*z5*cos(e4)*cos(e5) - a2*m4*x4*sin(e3)*sin(e4) - d4*m5*y5*sin(e4)*sin(e5) - d4*m6*z6*sin(e4)*sin(e5) - m6*x6*y6*cos(e4)*sin(e5) - m5*x5*z5*cos(e4)*sin(e5) - m6*x6*z6*cos(e6)*sin(e4) + m6*y6*z6*sin(e4)*sin(e6) + 2*m5*x5*y5*cos(e5)^2*sin(e4) - I6xx*cos(e4)*cos(e6)*sin(e5)*sin(e6) + I6yy*cos(e4)*cos(e6)*sin(e5)*sin(e6) - a2*m6*y6*cos(e4)*cos(e6)*sin(e3) + d4*m6*x6*cos(e5)*cos(e6)*sin(e4) + m6*y6*z6*cos(e4)*cos(e5)*cos(e6) - a2*m5*x5*cos(e5)*sin(e3)*sin(e4) - a2*m6*x6*cos(e4)*sin(e3)*sin(e6) - d4*m6*y6*cos(e5)*sin(e4)*sin(e6) + m6*x6*z6*cos(e4)*cos(e5)*sin(e6) + a2*m5*y5*sin(e3)*sin(e4)*sin(e5) + a2*m6*z6*sin(e3)*sin(e4)*sin(e5) + m6*x6^2*cos(e5)*cos(e6)^2*sin(e4)*sin(e5) - m6*y6^2*cos(e5)*cos(e6)^2*sin(e4)*sin(e5) + 2*m6*x6*y6*cos(e4)*cos(e6)^2*sin(e5) + 2*m6*x6*z6*cos(e5)^2*cos(e6)*sin(e4) - 2*m6*y6*z6*cos(e5)^2*sin(e4)*sin(e6) + m6*x6^2*cos(e4)*cos(e6)*sin(e5)*sin(e6) - m6*y6^2*cos(e4)*cos(e6)*sin(e5)*sin(e6) - a2*m6*x6*cos(e5)*cos(e6)*sin(e3)*sin(e4) + a2*m6*y6*cos(e5)*sin(e3)*sin(e4)*sin(e6) - 2*m6*x6*y6*cos(e5)*cos(e6)*sin(e4)*sin(e5)*sin(e6),I6xx*cos(e4) + I5zz*cos(e4) + m5*x5^2*cos(e4) + m5*y5^2*cos(e4) + m6*y6^2*cos(e4) + m6*z6^2*cos(e4) - I6xx*cos(e4)*cos(e6)^2 + I6yy*cos(e4)*cos(e6)^2 + a3*m5*x5*cos(e5) - a3*m5*y5*sin(e5) - a3*m6*z6*sin(e5) + m6*x6^2*cos(e4)*cos(e6)^2 - m6*y6^2*cos(e4)*cos(e6)^2 + a2*m5*x5*cos(e3)*cos(e5) + a3*m6*x6*cos(e5)*cos(e6) + d4*m5*y5*cos(e4)*cos(e5) + d4*m6*z6*cos(e4)*cos(e5) - a2*m5*y5*cos(e3)*sin(e5) - a3*m6*y6*cos(e5)*sin(e6) - a2*m6*z6*cos(e3)*sin(e5) + d4*m5*x5*cos(e4)*sin(e5) + m6*x6*y6*cos(e5)*sin(e4) + m5*x5*z5*cos(e5)*sin(e4) - m5*y5*z5*sin(e4)*sin(e5) + I6xx*cos(e5)*cos(e6)*sin(e4)*sin(e6) - I6yy*cos(e5)*cos(e6)*sin(e4)*sin(e6) - a2*m5*y5*cos(e4)*cos(e5)*sin(e3) - a2*m6*y6*cos(e3)*cos(e5)*sin(e6) - a2*m6*z6*cos(e4)*cos(e5)*sin(e3) + d4*m6*x6*cos(e4)*cos(e6)*sin(e5) - a2*m5*x5*cos(e4)*sin(e3)*sin(e5) - d4*m6*y6*cos(e4)*sin(e5)*sin(e6) - 2*m6*x6*y6*cos(e4)*cos(e6)*sin(e6) + m6*y6*z6*cos(e6)*sin(e4)*sin(e5) + m6*x6*z6*sin(e4)*sin(e5)*sin(e6) - 2*m6*x6*y6*cos(e5)*cos(e6)^2*sin(e4) - m6*x6^2*cos(e5)*cos(e6)*sin(e4)*sin(e6) + m6*y6^2*cos(e5)*cos(e6)*sin(e4)*sin(e6) + a2*m6*x6*cos(e3)*cos(e5)*cos(e6) - a2*m6*x6*cos(e4)*cos(e6)*sin(e3)*sin(e5) + a2*m6*y6*cos(e4)*sin(e3)*sin(e5)*sin(e6),I6zz*sin(e4)*sin(e5) + m6*x6^2*sin(e4)*sin(e5) + m6*y6^2*sin(e4)*sin(e5) - a3*m6*y6*cos(e6)*sin(e5) + d4*m6*x6*cos(e6)*sin(e4) + m6*y6*z6*cos(e4)*cos(e6) - a3*m6*x6*sin(e5)*sin(e6) - d4*m6*y6*sin(e4)*sin(e6) + m6*x6*z6*cos(e4)*sin(e6) + d4*m6*y6*cos(e4)*cos(e5)*cos(e6) - a2*m6*y6*cos(e3)*cos(e6)*sin(e5) + d4*m6*x6*cos(e4)*cos(e5)*sin(e6) - a2*m6*x6*cos(e6)*sin(e3)*sin(e4) - a2*m6*x6*cos(e3)*sin(e5)*sin(e6) + m6*x6*z6*cos(e5)*cos(e6)*sin(e4) + a2*m6*y6*sin(e3)*sin(e4)*sin(e6) - m6*y6*z6*cos(e5)*sin(e4)*sin(e6) - a2*m6*y6*cos(e4)*cos(e5)*cos(e6)*sin(e3) - a2*m6*x6*cos(e4)*cos(e5)*sin(e3)*sin(e6);
 m3*y3*z3*cos(e2)*sin(e3) - m3*x3*z3*cos(e2)*cos(e3) - m4*x4*y4*cos(e2)*cos(e3) + m3*y3*z3*cos(e3)*sin(e2) + m4*x4*y4*sin(e2)*sin(e3) + m3*x3*z3*sin(e2)*sin(e3) - I4xx*cos(e2)*cos(e3)*cos(e4)*sin(e4) + I6xx*cos(e2)*cos(e3)*cos(e4)*sin(e4) + I4yy*cos(e2)*cos(e3)*cos(e4)*sin(e4) - I5yy*cos(e2)*cos(e3)*cos(e4)*sin(e4) + I5zz*cos(e2)*cos(e3)*cos(e4)*sin(e4) - I6zz*cos(e2)*cos(e3)*cos(e4)*sin(e4) + I4xx*cos(e4)*sin(e2)*sin(e3)*sin(e4) - I6xx*cos(e4)*sin(e2)*sin(e3)*sin(e4) - I4yy*cos(e4)*sin(e2)*sin(e3)*sin(e4) + I5yy*cos(e4)*sin(e2)*sin(e3)*sin(e4) - I5zz*cos(e4)*sin(e2)*sin(e3)*sin(e4) + I6zz*cos(e4)*sin(e2)*sin(e3)*sin(e4) - a3*m5*z5*cos(e2)*cos(e3)*cos(e4) - I5xx*cos(e2)*cos(e3)*cos(e4)*cos(e5)^2*sin(e4) - I6xx*cos(e2)*cos(e3)*cos(e4)*cos(e6)^2*sin(e4) + I5yy*cos(e2)*cos(e3)*cos(e4)*cos(e5)^2*sin(e4) - I6yy*cos(e2)*cos(e3)*cos(e4)*cos(e5)^2*sin(e4) + I6yy*cos(e2)*cos(e3)*cos(e4)*cos(e6)^2*sin(e4) + I6zz*cos(e2)*cos(e3)*cos(e4)*cos(e5)^2*sin(e4) + a3*m4*x4*cos(e2)*cos(e3)*sin(e4) - d4*m4*y4*cos(e2)*cos(e4)*sin(e3) - d4*m4*y4*cos(e3)*cos(e4)*sin(e2) + d4*m5*z5*cos(e2)*cos(e4)*sin(e3) + d4*m5*z5*cos(e3)*cos(e4)*sin(e2) + m6*x6*y6*cos(e2)*cos(e3)*cos(e5) + m5*x5*z5*cos(e2)*cos(e3)*cos(e5) - a3*m4*y4*cos(e4)*sin(e2)*sin(e3) + a3*m5*z5*cos(e4)*sin(e2)*sin(e3) - d4*m4*x4*cos(e2)*sin(e3)*sin(e4) - d4*m4*x4*cos(e3)*sin(e2)*sin(e4) + I5xx*cos(e4)*cos(e5)^2*sin(e2)*sin(e3)*sin(e4) + I6xx*cos(e4)*cos(e6)^2*sin(e2)*sin(e3)*sin(e4) - I5yy*cos(e4)*cos(e5)^2*sin(e2)*sin(e3)*sin(e4) + I6yy*cos(e4)*cos(e5)^2*sin(e2)*sin(e3)*sin(e4) - I6yy*cos(e4)*cos(e6)^2*sin(e2)*sin(e3)*sin(e4) - I6zz*cos(e4)*cos(e5)^2*sin(e2)*sin(e3)*sin(e4) - m4*y4*z4*cos(e2)*cos(e4)*sin(e3) - m4*y4*z4*cos(e3)*cos(e4)*sin(e2) - m5*y5*z5*cos(e2)*cos(e3)*sin(e5) - a3*m4*x4*sin(e2)*sin(e3)*sin(e4) + m5*x5*y5*cos(e2)*sin(e3)*sin(e4) + m5*x5*y5*cos(e3)*sin(e2)*sin(e4) - m6*x6*y6*cos(e5)*sin(e2)*sin(e3) - m4*x4*z4*cos(e2)*sin(e3)*sin(e4) - m4*x4*z4*cos(e3)*sin(e2)*sin(e4) - m5*x5*z5*cos(e5)*sin(e2)*sin(e3) + m5*y5*z5*sin(e2)*sin(e3)*sin(e5) + 2*m4*x4*y4*cos(e2)*cos(e3)*cos(e4)^2 - 2*m4*x4*y4*cos(e4)^2*sin(e2)*sin(e3) + I6xx*cos(e2)*cos(e3)*cos(e5)*cos(e6)*sin(e6) - I6yy*cos(e2)*cos(e3)*cos(e5)*cos(e6)*sin(e6) + I5xx*cos(e2)*cos(e5)*sin(e3)*sin(e4)*sin(e5) + I5xx*cos(e3)*cos(e5)*sin(e2)*sin(e4)*sin(e5) - I6xx*cos(e5)*cos(e6)*sin(e2)*sin(e3)*sin(e6) - I5yy*cos(e2)*cos(e5)*sin(e3)*sin(e4)*sin(e5) - I5yy*cos(e3)*cos(e5)*sin(e2)*sin(e4)*sin(e5) + I6yy*cos(e2)*cos(e5)*sin(e3)*sin(e4)*sin(e5) + I6yy*cos(e3)*cos(e5)*sin(e2)*sin(e4)*sin(e5) + I6yy*cos(e5)*cos(e6)*sin(e2)*sin(e3)*sin(e6) - I6zz*cos(e2)*cos(e5)*sin(e3)*sin(e4)*sin(e5) - I6zz*cos(e3)*cos(e5)*sin(e2)*sin(e4)*sin(e5) + m4*x4^2*cos(e2)*cos(e3)*cos(e4)*sin(e4) - m6*x6^2*cos(e2)*cos(e3)*cos(e4)*sin(e4) - m4*y4^2*cos(e2)*cos(e3)*cos(e4)*sin(e4) + m5*y5^2*cos(e2)*cos(e3)*cos(e4)*sin(e4) - m5*z5^2*cos(e2)*cos(e3)*cos(e4)*sin(e4) + m6*z6^2*cos(e2)*cos(e3)*cos(e4)*sin(e4) - m4*x4^2*cos(e4)*sin(e2)*sin(e3)*sin(e4) + m6*x6^2*cos(e4)*sin(e2)*sin(e3)*sin(e4) + m4*y4^2*cos(e4)*sin(e2)*sin(e3)*sin(e4) - m5*y5^2*cos(e4)*sin(e2)*sin(e3)*sin(e4) + m5*z5^2*cos(e4)*sin(e2)*sin(e3)*sin(e4) - m6*z6^2*cos(e4)*sin(e2)*sin(e3)*sin(e4) + a3*m4*y4*cos(e2)*cos(e3)*cos(e4) + m5*x5*z5*cos(e2)*cos(e4)*sin(e3)*sin(e5) + m5*x5*z5*cos(e3)*cos(e4)*sin(e2)*sin(e5) + m6*x6*z6*cos(e2)*cos(e6)*sin(e3)*sin(e4) + m6*x6*z6*cos(e3)*cos(e6)*sin(e2)*sin(e4) + m6*x6*z6*cos(e2)*cos(e3)*sin(e5)*sin(e6) + a3*m5*y5*sin(e2)*sin(e3)*sin(e4)*sin(e5) + a3*m6*z6*sin(e2)*sin(e3)*sin(e4)*sin(e5) - m6*y6*z6*cos(e2)*sin(e3)*sin(e4)*sin(e6) - m6*y6*z6*cos(e3)*sin(e2)*sin(e4)*sin(e6) - m6*y6*z6*cos(e6)*sin(e2)*sin(e3)*sin(e5) - m5*x5^2*cos(e4)*cos(e5)^2*sin(e2)*sin(e3)*sin(e4) - m6*x6^2*cos(e4)*cos(e6)^2*sin(e2)*sin(e3)*sin(e4) + m5*y5^2*cos(e4)*cos(e5)^2*sin(e2)*sin(e3)*sin(e4) - m6*y6^2*cos(e4)*cos(e5)^2*sin(e2)*sin(e3)*sin(e4) + m6*y6^2*cos(e4)*cos(e6)^2*sin(e2)*sin(e3)*sin(e4) + m6*z6^2*cos(e4)*cos(e5)^2*sin(e2)*sin(e3)*sin(e4) - m6*x6*z6*sin(e2)*sin(e3)*sin(e5)*sin(e6) - I6xx*cos(e2)*cos(e3)*cos(e4)*cos(e5)^2*cos(e6)^2*sin(e4) + I6yy*cos(e2)*cos(e3)*cos(e4)*cos(e5)^2*cos(e6)^2*sin(e4) - 2*m6*x6*y6*cos(e2)*cos(e3)*cos(e4)^2*cos(e5) - 2*m6*x6*y6*cos(e2)*cos(e3)*cos(e5)*cos(e6)^2 - 2*m5*x5*z5*cos(e2)*cos(e3)*cos(e4)^2*cos(e5) + I6xx*cos(e4)*cos(e5)^2*cos(e6)^2*sin(e2)*sin(e3)*sin(e4) - I6yy*cos(e4)*cos(e5)^2*cos(e6)^2*sin(e2)*sin(e3)*sin(e4) + 2*m5*y5*z5*cos(e2)*cos(e3)*cos(e4)^2*sin(e5) - 2*m5*x5*y5*cos(e2)*cos(e5)^2*sin(e3)*sin(e4) - 2*m5*x5*y5*cos(e3)*cos(e5)^2*sin(e2)*sin(e4) + 2*m6*x6*y6*cos(e4)^2*cos(e5)*sin(e2)*sin(e3) + 2*m6*x6*y6*cos(e5)*cos(e6)^2*sin(e2)*sin(e3) + 2*m5*x5*z5*cos(e4)^2*cos(e5)*sin(e2)*sin(e3) - 2*m5*y5*z5*cos(e4)^2*sin(e2)*sin(e3)*sin(e5) + I6xx*cos(e2)*cos(e4)*cos(e6)*sin(e3)*sin(e5)*sin(e6) + I6xx*cos(e3)*cos(e4)*cos(e6)*sin(e2)*sin(e5)*sin(e6) - I6yy*cos(e2)*cos(e4)*cos(e6)*sin(e3)*sin(e5)*sin(e6) - I6yy*cos(e3)*cos(e4)*cos(e6)*sin(e2)*sin(e5)*sin(e6) - m6*x6^2*cos(e2)*cos(e3)*cos(e5)*cos(e6)*sin(e6) + m6*y6^2*cos(e2)*cos(e3)*cos(e5)*cos(e6)*sin(e6) - m5*x5^2*cos(e2)*cos(e5)*sin(e3)*sin(e4)*sin(e5) - m5*x5^2*cos(e3)*cos(e5)*sin(e2)*sin(e4)*sin(e5) + m6*x6^2*cos(e5)*cos(e6)*sin(e2)*sin(e3)*sin(e6) + m5*y5^2*cos(e2)*cos(e5)*sin(e3)*sin(e4)*sin(e5) + m5*y5^2*cos(e3)*cos(e5)*sin(e2)*sin(e4)*sin(e5) - m6*y6^2*cos(e2)*cos(e5)*sin(e3)*sin(e4)*sin(e5) - m6*y6^2*cos(e3)*cos(e5)*sin(e2)*sin(e4)*sin(e5) - m6*y6^2*cos(e5)*cos(e6)*sin(e2)*sin(e3)*sin(e6) + m6*z6^2*cos(e2)*cos(e5)*sin(e3)*sin(e4)*sin(e5) + m6*z6^2*cos(e3)*cos(e5)*sin(e2)*sin(e4)*sin(e5) + a3*m6*y6*cos(e2)*cos(e3)*cos(e4)*cos(e6) - 2*I6xx*cos(e2)*cos(e3)*cos(e4)^2*cos(e5)*cos(e6)*sin(e6) + 2*I6yy*cos(e2)*cos(e3)*cos(e4)^2*cos(e5)*cos(e6)*sin(e6) + a3*m5*x5*cos(e2)*cos(e3)*cos(e5)*sin(e4) + a3*m6*x6*cos(e2)*cos(e3)*cos(e4)*sin(e6) - d4*m6*y6*cos(e2)*cos(e4)*cos(e6)*sin(e3) - d4*m6*y6*cos(e3)*cos(e4)*cos(e6)*sin(e2) - a3*m5*y5*cos(e2)*cos(e3)*sin(e4)*sin(e5) - a3*m6*y6*cos(e4)*cos(e6)*sin(e2)*sin(e3) - a3*m6*z6*cos(e2)*cos(e3)*sin(e4)*sin(e5) - d4*m5*x5*cos(e2)*cos(e5)*sin(e3)*sin(e4) - d4*m5*x5*cos(e3)*cos(e5)*sin(e2)*sin(e4) - d4*m6*x6*cos(e2)*cos(e4)*sin(e3)*sin(e6) - d4*m6*x6*cos(e3)*cos(e4)*sin(e2)*sin(e6) + I6xx*cos(e2)*cos(e5)*cos(e6)^2*sin(e3)*sin(e4)*sin(e5) + I6xx*cos(e3)*cos(e5)*cos(e6)^2*sin(e2)*sin(e4)*sin(e5) + 2*I6xx*cos(e4)^2*cos(e5)*cos(e6)*sin(e2)*sin(e3)*sin(e6) - I6yy*cos(e2)*cos(e5)*cos(e6)^2*sin(e3)*sin(e4)*sin(e5) - I6yy*cos(e3)*cos(e5)*cos(e6)^2*sin(e2)*sin(e4)*sin(e5) - 2*I6yy*cos(e4)^2*cos(e5)*cos(e6)*sin(e2)*sin(e3)*sin(e6) + m5*y5*z5*cos(e2)*cos(e4)*cos(e5)*sin(e3) + m5*y5*z5*cos(e3)*cos(e4)*cos(e5)*sin(e2) + m6*y6*z6*cos(e2)*cos(e3)*cos(e6)*sin(e5) - a3*m5*x5*cos(e5)*sin(e2)*sin(e3)*sin(e4) - a3*m6*x6*cos(e4)*sin(e2)*sin(e3)*sin(e6) + d4*m5*y5*cos(e2)*sin(e3)*sin(e4)*sin(e5) + d4*m5*y5*cos(e3)*sin(e2)*sin(e4)*sin(e5) + d4*m6*z6*cos(e2)*sin(e3)*sin(e4)*sin(e5) + d4*m6*z6*cos(e3)*sin(e2)*sin(e4)*sin(e5) + m5*x5^2*cos(e2)*cos(e3)*cos(e4)*cos(e5)^2*sin(e4) + m6*x6^2*cos(e2)*cos(e3)*cos(e4)*cos(e6)^2*sin(e4) - m5*y5^2*cos(e2)*cos(e3)*cos(e4)*cos(e5)^2*sin(e4) + m6*y6^2*cos(e2)*cos(e3)*cos(e4)*cos(e5)^2*sin(e4) - m6*y6^2*cos(e2)*cos(e3)*cos(e4)*cos(e6)^2*sin(e4) + m6*x6*y6*cos(e2)*cos(e4)*sin(e3)*sin(e5) + m6*x6*y6*cos(e3)*cos(e4)*sin(e2)*sin(e5) - m6*z6^2*cos(e2)*cos(e3)*cos(e4)*cos(e5)^2*sin(e4) - 2*m6*y6*z6*cos(e2)*cos(e3)*cos(e4)^2*cos(e6)*sin(e5) + m6*x6^2*cos(e2)*cos(e3)*cos(e4)*cos(e5)^2*cos(e6)^2*sin(e4) - m6*y6^2*cos(e2)*cos(e3)*cos(e4)*cos(e5)^2*cos(e6)^2*sin(e4) - 2*m6*x6*y6*cos(e2)*cos(e4)*cos(e6)^2*sin(e3)*sin(e5) - 2*m6*x6*y6*cos(e3)*cos(e4)*cos(e6)^2*sin(e2)*sin(e5) - 2*m6*x6*z6*cos(e2)*cos(e3)*cos(e4)^2*sin(e5)*sin(e6) - 2*m6*x6*z6*cos(e2)*cos(e5)^2*cos(e6)*sin(e3)*sin(e4) - 2*m6*x6*z6*cos(e3)*cos(e5)^2*cos(e6)*sin(e2)*sin(e4) + 2*m6*y6*z6*cos(e2)*cos(e5)^2*sin(e3)*sin(e4)*sin(e6) + 2*m6*y6*z6*cos(e3)*cos(e5)^2*sin(e2)*sin(e4)*sin(e6) + 2*m6*y6*z6*cos(e4)^2*cos(e6)*sin(e2)*sin(e3)*sin(e5) - m6*x6^2*cos(e4)*cos(e5)^2*cos(e6)^2*sin(e2)*sin(e3)*sin(e4) + m6*y6^2*cos(e4)*cos(e5)^2*cos(e6)^2*sin(e2)*sin(e3)*sin(e4) + 2*m6*x6*z6*cos(e4)^2*sin(e2)*sin(e3)*sin(e5)*sin(e6) + 4*m6*x6*y6*cos(e2)*cos(e3)*cos(e4)^2*cos(e5)*cos(e6)^2 - m6*x6^2*cos(e2)*cos(e4)*cos(e6)*sin(e3)*sin(e5)*sin(e6) - m6*x6^2*cos(e3)*cos(e4)*cos(e6)*sin(e2)*sin(e5)*sin(e6) - 4*m6*x6*y6*cos(e4)^2*cos(e5)*cos(e6)^2*sin(e2)*sin(e3) + m6*y6^2*cos(e2)*cos(e4)*cos(e6)*sin(e3)*sin(e5)*sin(e6) + m6*y6^2*cos(e3)*cos(e4)*cos(e6)*sin(e2)*sin(e5)*sin(e6) + a3*m6*x6*cos(e2)*cos(e3)*cos(e5)*cos(e6)*sin(e4) - a3*m6*y6*cos(e2)*cos(e3)*cos(e5)*sin(e4)*sin(e6) - d4*m6*x6*cos(e2)*cos(e5)*cos(e6)*sin(e3)*sin(e4) - d4*m6*x6*cos(e3)*cos(e5)*cos(e6)*sin(e2)*sin(e4) - m6*y6*z6*cos(e2)*cos(e4)*cos(e5)*cos(e6)*sin(e3) - m6*y6*z6*cos(e3)*cos(e4)*cos(e5)*cos(e6)*sin(e2) - a3*m6*x6*cos(e5)*cos(e6)*sin(e2)*sin(e3)*sin(e4) + d4*m6*y6*cos(e2)*cos(e5)*sin(e3)*sin(e4)*sin(e6) + d4*m6*y6*cos(e3)*cos(e5)*sin(e2)*sin(e4)*sin(e6) + 2*m6*x6^2*cos(e2)*cos(e3)*cos(e4)^2*cos(e5)*cos(e6)*sin(e6) - 2*m6*y6^2*cos(e2)*cos(e3)*cos(e4)^2*cos(e5)*cos(e6)*sin(e6) - m6*x6*z6*cos(e2)*cos(e4)*cos(e5)*sin(e3)*sin(e6) - m6*x6*z6*cos(e3)*cos(e4)*cos(e5)*sin(e2)*sin(e6) + a3*m6*y6*cos(e5)*sin(e2)*sin(e3)*sin(e4)*sin(e6) - m6*x6^2*cos(e2)*cos(e5)*cos(e6)^2*sin(e3)*sin(e4)*sin(e5) - m6*x6^2*cos(e3)*cos(e5)*cos(e6)^2*sin(e2)*sin(e4)*sin(e5) - 2*m6*x6^2*cos(e4)^2*cos(e5)*cos(e6)*sin(e2)*sin(e3)*sin(e6) + m6*y6^2*cos(e2)*cos(e5)*cos(e6)^2*sin(e3)*sin(e4)*sin(e5) + m6*y6^2*cos(e3)*cos(e5)*cos(e6)^2*sin(e2)*sin(e4)*sin(e5) + 2*m6*y6^2*cos(e4)^2*cos(e5)*cos(e6)*sin(e2)*sin(e3)*sin(e6) - 2*m5*x5*y5*cos(e2)*cos(e3)*cos(e4)*cos(e5)*sin(e4)*sin(e5) - 2*m6*x6*y6*cos(e2)*cos(e3)*cos(e4)*cos(e6)*sin(e4)*sin(e6) + 2*m5*x5*y5*cos(e4)*cos(e5)*sin(e2)*sin(e3)*sin(e4)*sin(e5) + 2*m6*x6*y6*cos(e4)*cos(e6)*sin(e2)*sin(e3)*sin(e4)*sin(e6) - 2*m6*x6*z6*cos(e2)*cos(e3)*cos(e4)*cos(e5)*cos(e6)*sin(e4)*sin(e5) + 2*m6*y6*z6*cos(e2)*cos(e3)*cos(e4)*cos(e5)*sin(e4)*sin(e5)*sin(e6) + 2*m6*x6*y6*cos(e2)*cos(e5)*cos(e6)*sin(e3)*sin(e4)*sin(e5)*sin(e6) + 2*m6*x6*y6*cos(e3)*cos(e5)*cos(e6)*sin(e2)*sin(e4)*sin(e5)*sin(e6) + 2*m6*x6*z6*cos(e4)*cos(e5)*cos(e6)*sin(e2)*sin(e3)*sin(e4)*sin(e5) - 2*m6*y6*z6*cos(e4)*cos(e5)*sin(e2)*sin(e3)*sin(e4)*sin(e5)*sin(e6) - 2*m6*x6*y6*cos(e2)*cos(e3)*cos(e4)*cos(e5)^2*cos(e6)*sin(e4)*sin(e6) + 2*m6*x6*y6*cos(e4)*cos(e5)^2*cos(e6)*sin(e2)*sin(e3)*sin(e4)*sin(e6),I4xx + I5yy + I3zz + I6zz + a3^2*m4 + a3^2*m5 + a3^2*m6 + d4^2*m4 + d4^2*m5 + d4^2*m6 + m3*x3^2 + m5*x5^2 + m6*x6^2 + m3*y3^2 + m4*y4^2 + m6*y6^2 + m4*z4^2 + m5*z5^2 - I4xx*cos(e4)^2 + I5xx*cos(e5)^2 + I6xx*cos(e4)^2 + I4yy*cos(e4)^2 - I5yy*cos(e4)^2 - I5yy*cos(e5)^2 + I6yy*cos(e5)^2 + I5zz*cos(e4)^2 - I6zz*cos(e4)^2 - I6zz*cos(e5)^2 + 2*d4*m4*z4 + m4*x4^2*cos(e4)^2 - m5*x5^2*cos(e5)^2 - m6*x6^2*cos(e4)^2 - m4*y4^2*cos(e4)^2 + m5*y5^2*cos(e4)^2 + m5*y5^2*cos(e5)^2 - m6*y6^2*cos(e5)^2 - m5*z5^2*cos(e4)^2 + m6*z6^2*cos(e4)^2 + m6*z6^2*cos(e5)^2 - I5xx*cos(e4)^2*cos(e5)^2 - I6xx*cos(e4)^2*cos(e6)^2 + I6xx*cos(e5)^2*cos(e6)^2 + I5yy*cos(e4)^2*cos(e5)^2 - I6yy*cos(e4)^2*cos(e5)^2 + I6yy*cos(e4)^2*cos(e6)^2 - I6yy*cos(e5)^2*cos(e6)^2 + I6zz*cos(e4)^2*cos(e5)^2 - I6xx*cos(e4)^2*cos(e5)^2*cos(e6)^2 + I6yy*cos(e4)^2*cos(e5)^2*cos(e6)^2 + a2*a3*m4*cos(e3) + a2*a3*m5*cos(e3) + a2*a3*m6*cos(e3) - a2*d4*m4*sin(e3) - a2*d4*m5*sin(e3) - a2*d4*m6*sin(e3) + a2*m3*x3*cos(e3) + 2*a3*m4*x4*cos(e4) + 2*d4*m5*y5*cos(e5) + 2*d4*m6*z6*cos(e5) - a2*m3*y3*sin(e3) - 2*a3*m4*y4*sin(e4) - a2*m4*z4*sin(e3) + 2*a3*m5*z5*sin(e4) + 2*d4*m5*x5*sin(e5) + m5*x5^2*cos(e4)^2*cos(e5)^2 + m6*x6^2*cos(e4)^2*cos(e6)^2 - m6*x6^2*cos(e5)^2*cos(e6)^2 - m5*y5^2*cos(e4)^2*cos(e5)^2 + m6*y6^2*cos(e4)^2*cos(e5)^2 - m6*y6^2*cos(e4)^2*cos(e6)^2 + m6*y6^2*cos(e5)^2*cos(e6)^2 - m4*x4*y4*sin(2*e4) + m5*x5*y5*sin(2*e5) - m6*z6^2*cos(e4)^2*cos(e5)^2 + m6*x6^2*cos(e4)^2*cos(e5)^2*cos(e6)^2 - m6*y6^2*cos(e4)^2*cos(e5)^2*cos(e6)^2 + a2*m4*x4*cos(e3)*cos(e4) + 2*a3*m5*x5*cos(e4)*cos(e5) - a2*m4*y4*cos(e3)*sin(e4) - a2*m5*y5*cos(e5)*sin(e3) - 2*a3*m5*y5*cos(e4)*sin(e5) - 2*a3*m6*y6*cos(e6)*sin(e4) + a2*m5*z5*cos(e3)*sin(e4) - a2*m6*z6*cos(e5)*sin(e3) - 2*a3*m6*z6*cos(e4)*sin(e5) + 2*d4*m6*x6*cos(e6)*sin(e5) - a2*m5*x5*sin(e3)*sin(e5) - 2*a3*m6*x6*sin(e4)*sin(e6) - 2*d4*m6*y6*sin(e5)*sin(e6) - a2*m5*y5*cos(e3)*cos(e4)*sin(e5) - a2*m6*y6*cos(e3)*cos(e6)*sin(e4) - 2*a3*m6*y6*cos(e4)*cos(e5)*sin(e6) - a2*m6*z6*cos(e3)*cos(e4)*sin(e5) - a2*m6*x6*cos(e3)*sin(e4)*sin(e6) - a2*m6*x6*cos(e6)*sin(e3)*sin(e5) + 2*m6*x6*y6*cos(e4)*cos(e5)*sin(e4) + 2*m5*x5*z5*cos(e4)*cos(e5)*sin(e4) + 2*m6*x6*z6*cos(e5)*cos(e6)*sin(e5) + a2*m6*y6*sin(e3)*sin(e5)*sin(e6) - 2*m5*y5*z5*cos(e4)*sin(e4)*sin(e5) - 2*m6*y6*z6*cos(e5)*sin(e5)*sin(e6) - 2*m5*x5*y5*cos(e4)^2*cos(e5)*sin(e5) - 2*m6*x6*y6*cos(e4)^2*cos(e6)*sin(e6) + 2*m6*x6*y6*cos(e5)^2*cos(e6)*sin(e6) + 2*I6xx*cos(e4)*cos(e5)*cos(e6)*sin(e4)*sin(e6) - 2*I6yy*cos(e4)*cos(e5)*cos(e6)*sin(e4)*sin(e6) + a2*m5*x5*cos(e3)*cos(e4)*cos(e5) + 2*a3*m6*x6*cos(e4)*cos(e5)*cos(e6) + 2*m6*y6*z6*cos(e4)*cos(e6)*sin(e4)*sin(e5) + 2*m6*x6*z6*cos(e4)*sin(e4)*sin(e5)*sin(e6) - 4*m6*x6*y6*cos(e4)*cos(e5)*cos(e6)^2*sin(e4) - 2*m6*x6*z6*cos(e4)^2*cos(e5)*cos(e6)*sin(e5) + 2*m6*y6*z6*cos(e4)^2*cos(e5)*sin(e5)*sin(e6) - 2*m6*x6^2*cos(e4)*cos(e5)*cos(e6)*sin(e4)*sin(e6) - 2*m6*x6*y6*cos(e4)^2*cos(e5)^2*cos(e6)*sin(e6) + 2*m6*y6^2*cos(e4)*cos(e5)*cos(e6)*sin(e4)*sin(e6) + a2*m6*x6*cos(e3)*cos(e4)*cos(e5)*cos(e6) - a2*m6*y6*cos(e3)*cos(e4)*cos(e5)*sin(e6),I4xx + I5yy + I3zz + I6zz + a3^2*m4 + a3^2*m5 + a3^2*m6 + d4^2*m4 + d4^2*m5 + d4^2*m6 + m3*x3^2 + m5*x5^2 + m6*x6^2 + m3*y3^2 + m4*y4^2 + m6*y6^2 + m4*z4^2 + m5*z5^2 - I4xx*cos(e4)^2 + I5xx*cos(e5)^2 + I6xx*cos(e4)^2 + I4yy*cos(e4)^2 - I5yy*cos(e4)^2 - I5yy*cos(e5)^2 + I6yy*cos(e5)^2 + I5zz*cos(e4)^2 - I6zz*cos(e4)^2 - I6zz*cos(e5)^2 + 2*d4*m4*z4 + m4*x4^2*cos(e4)^2 - m5*x5^2*cos(e5)^2 - m6*x6^2*cos(e4)^2 - m4*y4^2*cos(e4)^2 + m5*y5^2*cos(e4)^2 + m5*y5^2*cos(e5)^2 - m6*y6^2*cos(e5)^2 - m5*z5^2*cos(e4)^2 + m6*z6^2*cos(e4)^2 + m6*z6^2*cos(e5)^2 - I5xx*cos(e4)^2*cos(e5)^2 - I6xx*cos(e4)^2*cos(e6)^2 + I6xx*cos(e5)^2*cos(e6)^2 + I5yy*cos(e4)^2*cos(e5)^2 - I6yy*cos(e4)^2*cos(e5)^2 + I6yy*cos(e4)^2*cos(e6)^2 - I6yy*cos(e5)^2*cos(e6)^2 + I6zz*cos(e4)^2*cos(e5)^2 - I6xx*cos(e4)^2*cos(e5)^2*cos(e6)^2 + I6yy*cos(e4)^2*cos(e5)^2*cos(e6)^2 + 2*a3*m4*x4*cos(e4) + 2*d4*m5*y5*cos(e5) + 2*d4*m6*z6*cos(e5) - 2*a3*m4*y4*sin(e4) + 2*a3*m5*z5*sin(e4) + 2*d4*m5*x5*sin(e5) + m5*x5^2*cos(e4)^2*cos(e5)^2 + m6*x6^2*cos(e4)^2*cos(e6)^2 - m6*x6^2*cos(e5)^2*cos(e6)^2 - m5*y5^2*cos(e4)^2*cos(e5)^2 + m6*y6^2*cos(e4)^2*cos(e5)^2 - m6*y6^2*cos(e4)^2*cos(e6)^2 + m6*y6^2*cos(e5)^2*cos(e6)^2 - m4*x4*y4*sin(2*e4) + m5*x5*y5*sin(2*e5) - m6*z6^2*cos(e4)^2*cos(e5)^2 + m6*x6^2*cos(e4)^2*cos(e5)^2*cos(e6)^2 - m6*y6^2*cos(e4)^2*cos(e5)^2*cos(e6)^2 + 2*a3*m5*x5*cos(e4)*cos(e5) - 2*a3*m5*y5*cos(e4)*sin(e5) - 2*a3*m6*y6*cos(e6)*sin(e4) - 2*a3*m6*z6*cos(e4)*sin(e5) + 2*d4*m6*x6*cos(e6)*sin(e5) - 2*a3*m6*x6*sin(e4)*sin(e6) - 2*d4*m6*y6*sin(e5)*sin(e6) - 2*a3*m6*y6*cos(e4)*cos(e5)*sin(e6) + 2*m6*x6*y6*cos(e4)*cos(e5)*sin(e4) + 2*m5*x5*z5*cos(e4)*cos(e5)*sin(e4) + 2*m6*x6*z6*cos(e5)*cos(e6)*sin(e5) - 2*m5*y5*z5*cos(e4)*sin(e4)*sin(e5) - 2*m6*y6*z6*cos(e5)*sin(e5)*sin(e6) - 2*m5*x5*y5*cos(e4)^2*cos(e5)*sin(e5) - 2*m6*x6*y6*cos(e4)^2*cos(e6)*sin(e6) + 2*m6*x6*y6*cos(e5)^2*cos(e6)*sin(e6) + 2*I6xx*cos(e4)*cos(e5)*cos(e6)*sin(e4)*sin(e6) - 2*I6yy*cos(e4)*cos(e5)*cos(e6)*sin(e4)*sin(e6) + 2*a3*m6*x6*cos(e4)*cos(e5)*cos(e6) + 2*m6*y6*z6*cos(e4)*cos(e6)*sin(e4)*sin(e5) + 2*m6*x6*z6*cos(e4)*sin(e4)*sin(e5)*sin(e6) - 4*m6*x6*y6*cos(e4)*cos(e5)*cos(e6)^2*sin(e4) - 2*m6*x6*z6*cos(e4)^2*cos(e5)*cos(e6)*sin(e5) + 2*m6*y6*z6*cos(e4)^2*cos(e5)*sin(e5)*sin(e6) - 2*m6*x6^2*cos(e4)*cos(e5)*cos(e6)*sin(e4)*sin(e6) - 2*m6*x6*y6*cos(e4)^2*cos(e5)^2*cos(e6)*sin(e6) + 2*m6*y6^2*cos(e4)*cos(e5)*cos(e6)*sin(e4)*sin(e6),I5yy*cos(e5)*sin(e4)*sin(e5) - I5xx*cos(e5)*sin(e4)*sin(e5) - I6yy*cos(e5)*sin(e4)*sin(e5) + I6zz*cos(e5)*sin(e4)*sin(e5) + d4*m4*y4*cos(e4) - d4*m5*z5*cos(e4) + d4*m4*x4*sin(e4) + m4*y4*z4*cos(e4) - m5*x5*y5*sin(e4) + m4*x4*z4*sin(e4) + m5*x5^2*cos(e5)*sin(e4)*sin(e5) - m5*y5^2*cos(e5)*sin(e4)*sin(e5) + m6*y6^2*cos(e5)*sin(e4)*sin(e5) - m6*z6^2*cos(e5)*sin(e4)*sin(e5) + d4*m6*y6*cos(e4)*cos(e6) + d4*m5*x5*cos(e5)*sin(e4) + d4*m6*x6*cos(e4)*sin(e6) - I6xx*cos(e5)*cos(e6)^2*sin(e4)*sin(e5) + I6yy*cos(e5)*cos(e6)^2*sin(e4)*sin(e5) - m5*y5*z5*cos(e4)*cos(e5) - d4*m5*y5*sin(e4)*sin(e5) - d4*m6*z6*sin(e4)*sin(e5) - m6*x6*y6*cos(e4)*sin(e5) - m5*x5*z5*cos(e4)*sin(e5) - m6*x6*z6*cos(e6)*sin(e4) + m6*y6*z6*sin(e4)*sin(e6) + 2*m5*x5*y5*cos(e5)^2*sin(e4) - I6xx*cos(e4)*cos(e6)*sin(e5)*sin(e6) + I6yy*cos(e4)*cos(e6)*sin(e5)*sin(e6) + d4*m6*x6*cos(e5)*cos(e6)*sin(e4) + m6*y6*z6*cos(e4)*cos(e5)*cos(e6) - d4*m6*y6*cos(e5)*sin(e4)*sin(e6) + m6*x6*z6*cos(e4)*cos(e5)*sin(e6) + m6*x6^2*cos(e5)*cos(e6)^2*sin(e4)*sin(e5) - m6*y6^2*cos(e5)*cos(e6)^2*sin(e4)*sin(e5) + 2*m6*x6*y6*cos(e4)*cos(e6)^2*sin(e5) + 2*m6*x6*z6*cos(e5)^2*cos(e6)*sin(e4) - 2*m6*y6*z6*cos(e5)^2*sin(e4)*sin(e6) + m6*x6^2*cos(e4)*cos(e6)*sin(e5)*sin(e6) - m6*y6^2*cos(e4)*cos(e6)*sin(e5)*sin(e6) - 2*m6*x6*y6*cos(e5)*cos(e6)*sin(e4)*sin(e5)*sin(e6),I6xx*cos(e4) + I5zz*cos(e4) + m5*x5^2*cos(e4) + m5*y5^2*cos(e4) + m6*y6^2*cos(e4) + m6*z6^2*cos(e4) - I6xx*cos(e4)*cos(e6)^2 + I6yy*cos(e4)*cos(e6)^2 + a3*m5*x5*cos(e5) - a3*m5*y5*sin(e5) - a3*m6*z6*sin(e5) + m6*x6^2*cos(e4)*cos(e6)^2 - m6*y6^2*cos(e4)*cos(e6)^2 + a3*m6*x6*cos(e5)*cos(e6) + d4*m5*y5*cos(e4)*cos(e5) + d4*m6*z6*cos(e4)*cos(e5) - a3*m6*y6*cos(e5)*sin(e6) + d4*m5*x5*cos(e4)*sin(e5) + m6*x6*y6*cos(e5)*sin(e4) + m5*x5*z5*cos(e5)*sin(e4) - m5*y5*z5*sin(e4)*sin(e5) + I6xx*cos(e5)*cos(e6)*sin(e4)*sin(e6) - I6yy*cos(e5)*cos(e6)*sin(e4)*sin(e6) + d4*m6*x6*cos(e4)*cos(e6)*sin(e5) - d4*m6*y6*cos(e4)*sin(e5)*sin(e6) - 2*m6*x6*y6*cos(e4)*cos(e6)*sin(e6) + m6*y6*z6*cos(e6)*sin(e4)*sin(e5) + m6*x6*z6*sin(e4)*sin(e5)*sin(e6) - 2*m6*x6*y6*cos(e5)*cos(e6)^2*sin(e4) - m6*x6^2*cos(e5)*cos(e6)*sin(e4)*sin(e6) + m6*y6^2*cos(e5)*cos(e6)*sin(e4)*sin(e6),I6zz*sin(e4)*sin(e5) + m6*x6^2*sin(e4)*sin(e5) + m6*y6^2*sin(e4)*sin(e5) - a3*m6*y6*cos(e6)*sin(e5) + d4*m6*x6*cos(e6)*sin(e4) + m6*y6*z6*cos(e4)*cos(e6) - a3*m6*x6*sin(e5)*sin(e6) - d4*m6*y6*sin(e4)*sin(e6) + m6*x6*z6*cos(e4)*sin(e6) + d4*m6*y6*cos(e4)*cos(e5)*cos(e6) + d4*m6*x6*cos(e4)*cos(e5)*sin(e6) + m6*x6*z6*cos(e5)*cos(e6)*sin(e4) - m6*y6*z6*cos(e5)*sin(e4)*sin(e6);
 I5xx*cos(e2)*cos(e5)^2*sin(e3) - I5xx*cos(e3)*sin(e2) - I6yy*cos(e2)*sin(e3) - I6yy*cos(e3)*sin(e2) - I4zz*cos(e2)*sin(e3) - I4zz*cos(e3)*sin(e2) - m4*x4^2*cos(e2)*sin(e3) - m4*x4^2*cos(e3)*sin(e2) - m6*x6^2*cos(e2)*sin(e3) - m6*x6^2*cos(e3)*sin(e2) - m4*y4^2*cos(e2)*sin(e3) - m4*y4^2*cos(e3)*sin(e2) - m5*y5^2*cos(e2)*sin(e3) - m5*y5^2*cos(e3)*sin(e2) - m5*z5^2*cos(e2)*sin(e3) - m5*z5^2*cos(e3)*sin(e2) - m6*z6^2*cos(e2)*sin(e3) - m6*z6^2*cos(e3)*sin(e2) - a1*m4*x4*cos(e4) - I5xx*cos(e2)*sin(e3) + I5xx*cos(e3)*cos(e5)^2*sin(e2) - I6xx*cos(e2)*cos(e6)^2*sin(e3) - I6xx*cos(e3)*cos(e6)^2*sin(e2) - I5yy*cos(e2)*cos(e5)^2*sin(e3) - I5yy*cos(e3)*cos(e5)^2*sin(e2) + I6yy*cos(e2)*cos(e5)^2*sin(e3) + I6yy*cos(e3)*cos(e5)^2*sin(e2) + I6yy*cos(e2)*cos(e6)^2*sin(e3) + I6yy*cos(e3)*cos(e6)^2*sin(e2) - I6zz*cos(e2)*cos(e5)^2*sin(e3) - I6zz*cos(e3)*cos(e5)^2*sin(e2) + a1*m4*y4*sin(e4) - a1*m5*z5*sin(e4) - a1*m5*x5*cos(e4)*cos(e5) - a2*m4*x4*cos(e4)*sin(e2) + a1*m5*y5*cos(e4)*sin(e5) + a1*m6*y6*cos(e6)*sin(e4) + a1*m6*z6*cos(e4)*sin(e5) + a1*m6*x6*sin(e4)*sin(e6) + a2*m4*y4*sin(e2)*sin(e4) - a2*m5*z5*sin(e2)*sin(e4) - m5*x5^2*cos(e2)*cos(e5)^2*sin(e3) - m5*x5^2*cos(e3)*cos(e5)^2*sin(e2) + m6*x6^2*cos(e2)*cos(e6)^2*sin(e3) + m6*x6^2*cos(e3)*cos(e6)^2*sin(e2) + m5*y5^2*cos(e2)*cos(e5)^2*sin(e3) + m5*y5^2*cos(e3)*cos(e5)^2*sin(e2) - m6*y6^2*cos(e2)*cos(e5)^2*sin(e3) - m6*y6^2*cos(e3)*cos(e5)^2*sin(e2) - m6*y6^2*cos(e2)*cos(e6)^2*sin(e3) - m6*y6^2*cos(e3)*cos(e6)^2*sin(e2) + m6*z6^2*cos(e2)*cos(e5)^2*sin(e3) + m6*z6^2*cos(e3)*cos(e5)^2*sin(e2) + I6xx*cos(e2)*cos(e5)^2*cos(e6)^2*sin(e3) + I6xx*cos(e3)*cos(e5)^2*cos(e6)^2*sin(e2) - I6yy*cos(e2)*cos(e5)^2*cos(e6)^2*sin(e3) - I6yy*cos(e3)*cos(e5)^2*cos(e6)^2*sin(e2) - d4*m4*x4*cos(e2)*cos(e3)*cos(e4) - a3*m4*x4*cos(e2)*cos(e4)*sin(e3) - a3*m4*x4*cos(e3)*cos(e4)*sin(e2) - a2*m5*x5*cos(e4)*cos(e5)*sin(e2) + a1*m6*y6*cos(e4)*cos(e5)*sin(e6) + d4*m4*y4*cos(e2)*cos(e3)*sin(e4) - d4*m5*z5*cos(e2)*cos(e3)*sin(e4) + m5*x5*y5*cos(e2)*cos(e3)*cos(e4) - m4*x4*z4*cos(e2)*cos(e3)*cos(e4) + a3*m4*y4*cos(e2)*sin(e3)*sin(e4) + a3*m4*y4*cos(e3)*sin(e2)*sin(e4) + a2*m5*y5*cos(e4)*sin(e2)*sin(e5) + a2*m6*y6*cos(e6)*sin(e2)*sin(e4) - a3*m5*z5*cos(e2)*sin(e3)*sin(e4) - a3*m5*z5*cos(e3)*sin(e2)*sin(e4) + a2*m6*z6*cos(e4)*sin(e2)*sin(e5) + d4*m4*x4*cos(e4)*sin(e2)*sin(e3) + m4*y4*z4*cos(e2)*cos(e3)*sin(e4) + a2*m6*x6*sin(e2)*sin(e4)*sin(e6) - d4*m4*y4*sin(e2)*sin(e3)*sin(e4) + d4*m5*z5*sin(e2)*sin(e3)*sin(e4) - m5*x5*y5*cos(e4)*sin(e2)*sin(e3) + m4*x4*z4*cos(e4)*sin(e2)*sin(e3) - m4*y4*z4*sin(e2)*sin(e3)*sin(e4) - m6*x6^2*cos(e2)*cos(e5)^2*cos(e6)^2*sin(e3) - m6*x6^2*cos(e3)*cos(e5)^2*cos(e6)^2*sin(e2) + m6*y6^2*cos(e2)*cos(e5)^2*cos(e6)^2*sin(e3) + m6*y6^2*cos(e3)*cos(e5)^2*cos(e6)^2*sin(e2) + I5xx*cos(e2)*cos(e3)*cos(e4)*cos(e5)*sin(e5) - I5yy*cos(e2)*cos(e3)*cos(e4)*cos(e5)*sin(e5) + I6yy*cos(e2)*cos(e3)*cos(e4)*cos(e5)*sin(e5) - I6zz*cos(e2)*cos(e3)*cos(e4)*cos(e5)*sin(e5) - I5xx*cos(e4)*cos(e5)*sin(e2)*sin(e3)*sin(e5) + I5yy*cos(e4)*cos(e5)*sin(e2)*sin(e3)*sin(e5) - I6yy*cos(e4)*cos(e5)*sin(e2)*sin(e3)*sin(e5) + I6zz*cos(e4)*cos(e5)*sin(e2)*sin(e3)*sin(e5) - a1*m6*x6*cos(e4)*cos(e5)*cos(e6) - m5*x5*z5*cos(e2)*cos(e3)*sin(e4)*sin(e5) - m6*x6*z6*cos(e4)*cos(e6)*sin(e2)*sin(e3) - d4*m6*x6*sin(e2)*sin(e3)*sin(e4)*sin(e6) + m5*y5*z5*cos(e5)*sin(e2)*sin(e3)*sin(e4) + m6*y6*z6*cos(e4)*sin(e2)*sin(e3)*sin(e6) + m6*x6*y6*sin(e2)*sin(e3)*sin(e4)*sin(e5) + m5*x5*z5*sin(e2)*sin(e3)*sin(e4)*sin(e5) - 2*m5*x5*y5*cos(e2)*cos(e3)*cos(e4)*cos(e5)^2 + 2*m5*x5*y5*cos(e4)*cos(e5)^2*sin(e2)*sin(e3) - I6xx*cos(e2)*cos(e3)*cos(e6)*sin(e4)*sin(e5)*sin(e6) + I6yy*cos(e2)*cos(e3)*cos(e6)*sin(e4)*sin(e5)*sin(e6) - m5*x5^2*cos(e2)*cos(e3)*cos(e4)*cos(e5)*sin(e5) + m5*y5^2*cos(e2)*cos(e3)*cos(e4)*cos(e5)*sin(e5) - m6*y6^2*cos(e2)*cos(e3)*cos(e4)*cos(e5)*sin(e5) + m6*z6^2*cos(e2)*cos(e3)*cos(e4)*cos(e5)*sin(e5) + I6xx*cos(e6)*sin(e2)*sin(e3)*sin(e4)*sin(e5)*sin(e6) - I6yy*cos(e6)*sin(e2)*sin(e3)*sin(e4)*sin(e5)*sin(e6) + m5*x5^2*cos(e4)*cos(e5)*sin(e2)*sin(e3)*sin(e5) - m5*y5^2*cos(e4)*cos(e5)*sin(e2)*sin(e3)*sin(e5) + m6*y6^2*cos(e4)*cos(e5)*sin(e2)*sin(e3)*sin(e5) - m6*z6^2*cos(e4)*cos(e5)*sin(e2)*sin(e3)*sin(e5) - d4*m5*x5*cos(e2)*cos(e3)*cos(e4)*cos(e5) + I6xx*cos(e2)*cos(e3)*cos(e4)*cos(e5)*cos(e6)^2*sin(e5) - I6yy*cos(e2)*cos(e3)*cos(e4)*cos(e5)*cos(e6)^2*sin(e5) - a3*m5*x5*cos(e2)*cos(e4)*cos(e5)*sin(e3) - a3*m5*x5*cos(e3)*cos(e4)*cos(e5)*sin(e2) - a2*m6*x6*cos(e4)*cos(e5)*cos(e6)*sin(e2) + d4*m5*y5*cos(e2)*cos(e3)*cos(e4)*sin(e5) + d4*m6*y6*cos(e2)*cos(e3)*cos(e6)*sin(e4) + d4*m6*z6*cos(e2)*cos(e3)*cos(e4)*sin(e5) + m6*x6*z6*cos(e2)*cos(e3)*cos(e4)*cos(e6) + a3*m5*y5*cos(e2)*cos(e4)*sin(e3)*sin(e5) + a3*m5*y5*cos(e3)*cos(e4)*sin(e2)*sin(e5) + a3*m6*y6*cos(e2)*cos(e6)*sin(e3)*sin(e4) + a3*m6*y6*cos(e3)*cos(e6)*sin(e2)*sin(e4) + a2*m6*y6*cos(e4)*cos(e5)*sin(e2)*sin(e6) + a3*m6*z6*cos(e2)*cos(e4)*sin(e3)*sin(e5) + a3*m6*z6*cos(e3)*cos(e4)*sin(e2)*sin(e5) + d4*m5*x5*cos(e4)*cos(e5)*sin(e2)*sin(e3) + d4*m6*x6*cos(e2)*cos(e3)*sin(e4)*sin(e6) - I6xx*cos(e4)*cos(e5)*cos(e6)^2*sin(e2)*sin(e3)*sin(e5) + I6yy*cos(e4)*cos(e5)*cos(e6)^2*sin(e2)*sin(e3)*sin(e5) - m5*y5*z5*cos(e2)*cos(e3)*cos(e5)*sin(e4) - m6*y6*z6*cos(e2)*cos(e3)*cos(e4)*sin(e6) + a3*m6*x6*cos(e2)*sin(e3)*sin(e4)*sin(e6) + a3*m6*x6*cos(e3)*sin(e2)*sin(e4)*sin(e6) - d4*m5*y5*cos(e4)*sin(e2)*sin(e3)*sin(e5) - d4*m6*y6*cos(e6)*sin(e2)*sin(e3)*sin(e4) - d4*m6*z6*cos(e4)*sin(e2)*sin(e3)*sin(e5) + 2*m5*x5*y5*cos(e2)*cos(e5)*sin(e3)*sin(e5) + 2*m5*x5*y5*cos(e3)*cos(e5)*sin(e2)*sin(e5) - m6*x6*y6*cos(e2)*cos(e3)*sin(e4)*sin(e5) - 2*m6*x6*y6*cos(e2)*cos(e6)*sin(e3)*sin(e6) - 2*m6*x6*y6*cos(e3)*cos(e6)*sin(e2)*sin(e6) - 2*m6*x6*z6*cos(e2)*cos(e3)*cos(e4)*cos(e5)^2*cos(e6) + 2*m6*y6*z6*cos(e2)*cos(e3)*cos(e4)*cos(e5)^2*sin(e6) + 2*m6*x6*y6*cos(e2)*cos(e3)*cos(e6)^2*sin(e4)*sin(e5) + 2*m6*x6*y6*cos(e2)*cos(e5)^2*cos(e6)*sin(e3)*sin(e6) + 2*m6*x6*y6*cos(e3)*cos(e5)^2*cos(e6)*sin(e2)*sin(e6) + 2*m6*x6*z6*cos(e4)*cos(e5)^2*cos(e6)*sin(e2)*sin(e3) - 2*m6*y6*z6*cos(e4)*cos(e5)^2*sin(e2)*sin(e3)*sin(e6) - 2*m6*x6*y6*cos(e6)^2*sin(e2)*sin(e3)*sin(e4)*sin(e5) + m6*x6^2*cos(e2)*cos(e3)*cos(e6)*sin(e4)*sin(e5)*sin(e6) - m6*y6^2*cos(e2)*cos(e3)*cos(e6)*sin(e4)*sin(e5)*sin(e6) - d4*m6*x6*cos(e2)*cos(e3)*cos(e4)*cos(e5)*cos(e6) - a3*m6*x6*cos(e2)*cos(e4)*cos(e5)*cos(e6)*sin(e3) - a3*m6*x6*cos(e3)*cos(e4)*cos(e5)*cos(e6)*sin(e2) + d4*m6*y6*cos(e2)*cos(e3)*cos(e4)*cos(e5)*sin(e6) - m6*x6^2*cos(e6)*sin(e2)*sin(e3)*sin(e4)*sin(e5)*sin(e6) + m6*y6^2*cos(e6)*sin(e2)*sin(e3)*sin(e4)*sin(e5)*sin(e6) + a3*m6*y6*cos(e2)*cos(e4)*cos(e5)*sin(e3)*sin(e6) + a3*m6*y6*cos(e3)*cos(e4)*cos(e5)*sin(e2)*sin(e6) + d4*m6*x6*cos(e4)*cos(e5)*cos(e6)*sin(e2)*sin(e3) + m6*y6*z6*cos(e2)*cos(e3)*cos(e5)*cos(e6)*sin(e4) - d4*m6*y6*cos(e4)*cos(e5)*sin(e2)*sin(e3)*sin(e6) - m6*x6^2*cos(e2)*cos(e3)*cos(e4)*cos(e5)*cos(e6)^2*sin(e5) + m6*y6^2*cos(e2)*cos(e3)*cos(e4)*cos(e5)*cos(e6)^2*sin(e5) + m6*x6*z6*cos(e2)*cos(e3)*cos(e5)*sin(e4)*sin(e6) + 2*m6*x6*z6*cos(e2)*cos(e5)*cos(e6)*sin(e3)*sin(e5) + 2*m6*x6*z6*cos(e3)*cos(e5)*cos(e6)*sin(e2)*sin(e5) - m6*y6*z6*cos(e5)*cos(e6)*sin(e2)*sin(e3)*sin(e4) - 2*m6*y6*z6*cos(e2)*cos(e5)*sin(e3)*sin(e5)*sin(e6) - 2*m6*y6*z6*cos(e3)*cos(e5)*sin(e2)*sin(e5)*sin(e6) + m6*x6^2*cos(e4)*cos(e5)*cos(e6)^2*sin(e2)*sin(e3)*sin(e5) - m6*y6^2*cos(e4)*cos(e5)*cos(e6)^2*sin(e2)*sin(e3)*sin(e5) - m6*x6*z6*cos(e5)*sin(e2)*sin(e3)*sin(e4)*sin(e6) + 2*m6*x6*y6*cos(e2)*cos(e3)*cos(e4)*cos(e5)*cos(e6)*sin(e5)*sin(e6) - 2*m6*x6*y6*cos(e4)*cos(e5)*cos(e6)*sin(e2)*sin(e3)*sin(e5)*sin(e6),I5yy*cos(e5)*sin(e4)*sin(e5) - I5xx*cos(e5)*sin(e4)*sin(e5) - I6yy*cos(e5)*sin(e4)*sin(e5) + I6zz*cos(e5)*sin(e4)*sin(e5) + d4*m4*y4*cos(e4) - d4*m5*z5*cos(e4) + d4*m4*x4*sin(e4) + m4*y4*z4*cos(e4) - m5*x5*y5*sin(e4) + m4*x4*z4*sin(e4) + m5*x5^2*cos(e5)*sin(e4)*sin(e5) - m5*y5^2*cos(e5)*sin(e4)*sin(e5) + m6*y6^2*cos(e5)*sin(e4)*sin(e5) - m6*z6^2*cos(e5)*sin(e4)*sin(e5) + d4*m6*y6*cos(e4)*cos(e6) - a2*m4*y4*cos(e4)*sin(e3) + a2*m5*z5*cos(e4)*sin(e3) + d4*m5*x5*cos(e5)*sin(e4) + d4*m6*x6*cos(e4)*sin(e6) - I6xx*cos(e5)*cos(e6)^2*sin(e4)*sin(e5) + I6yy*cos(e5)*cos(e6)^2*sin(e4)*sin(e5) - m5*y5*z5*cos(e4)*cos(e5) - a2*m4*x4*sin(e3)*sin(e4) - d4*m5*y5*sin(e4)*sin(e5) - d4*m6*z6*sin(e4)*sin(e5) - m6*x6*y6*cos(e4)*sin(e5) - m5*x5*z5*cos(e4)*sin(e5) - m6*x6*z6*cos(e6)*sin(e4) + m6*y6*z6*sin(e4)*sin(e6) + 2*m5*x5*y5*cos(e5)^2*sin(e4) - I6xx*cos(e4)*cos(e6)*sin(e5)*sin(e6) + I6yy*cos(e4)*cos(e6)*sin(e5)*sin(e6) - a2*m6*y6*cos(e4)*cos(e6)*sin(e3) + d4*m6*x6*cos(e5)*cos(e6)*sin(e4) + m6*y6*z6*cos(e4)*cos(e5)*cos(e6) - a2*m5*x5*cos(e5)*sin(e3)*sin(e4) - a2*m6*x6*cos(e4)*sin(e3)*sin(e6) - d4*m6*y6*cos(e5)*sin(e4)*sin(e6) + m6*x6*z6*cos(e4)*cos(e5)*sin(e6) + a2*m5*y5*sin(e3)*sin(e4)*sin(e5) + a2*m6*z6*sin(e3)*sin(e4)*sin(e5) + m6*x6^2*cos(e5)*cos(e6)^2*sin(e4)*sin(e5) - m6*y6^2*cos(e5)*cos(e6)^2*sin(e4)*sin(e5) + 2*m6*x6*y6*cos(e4)*cos(e6)^2*sin(e5) + 2*m6*x6*z6*cos(e5)^2*cos(e6)*sin(e4) - 2*m6*y6*z6*cos(e5)^2*sin(e4)*sin(e6) + m6*x6^2*cos(e4)*cos(e6)*sin(e5)*sin(e6) - m6*y6^2*cos(e4)*cos(e6)*sin(e5)*sin(e6) - a2*m6*x6*cos(e5)*cos(e6)*sin(e3)*sin(e4) + a2*m6*y6*cos(e5)*sin(e3)*sin(e4)*sin(e6) - 2*m6*x6*y6*cos(e5)*cos(e6)*sin(e4)*sin(e5)*sin(e6),I5yy*cos(e5)*sin(e4)*sin(e5) - I5xx*cos(e5)*sin(e4)*sin(e5) - I6yy*cos(e5)*sin(e4)*sin(e5) + I6zz*cos(e5)*sin(e4)*sin(e5) + d4*m4*y4*cos(e4) - d4*m5*z5*cos(e4) + d4*m4*x4*sin(e4) + m4*y4*z4*cos(e4) - m5*x5*y5*sin(e4) + m4*x4*z4*sin(e4) + m5*x5^2*cos(e5)*sin(e4)*sin(e5) - m5*y5^2*cos(e5)*sin(e4)*sin(e5) + m6*y6^2*cos(e5)*sin(e4)*sin(e5) - m6*z6^2*cos(e5)*sin(e4)*sin(e5) + d4*m6*y6*cos(e4)*cos(e6) + d4*m5*x5*cos(e5)*sin(e4) + d4*m6*x6*cos(e4)*sin(e6) - I6xx*cos(e5)*cos(e6)^2*sin(e4)*sin(e5) + I6yy*cos(e5)*cos(e6)^2*sin(e4)*sin(e5) - m5*y5*z5*cos(e4)*cos(e5) - d4*m5*y5*sin(e4)*sin(e5) - d4*m6*z6*sin(e4)*sin(e5) - m6*x6*y6*cos(e4)*sin(e5) - m5*x5*z5*cos(e4)*sin(e5) - m6*x6*z6*cos(e6)*sin(e4) + m6*y6*z6*sin(e4)*sin(e6) + 2*m5*x5*y5*cos(e5)^2*sin(e4) - I6xx*cos(e4)*cos(e6)*sin(e5)*sin(e6) + I6yy*cos(e4)*cos(e6)*sin(e5)*sin(e6) + d4*m6*x6*cos(e5)*cos(e6)*sin(e4) + m6*y6*z6*cos(e4)*cos(e5)*cos(e6) - d4*m6*y6*cos(e5)*sin(e4)*sin(e6) + m6*x6*z6*cos(e4)*cos(e5)*sin(e6) + m6*x6^2*cos(e5)*cos(e6)^2*sin(e4)*sin(e5) - m6*y6^2*cos(e5)*cos(e6)^2*sin(e4)*sin(e5) + 2*m6*x6*y6*cos(e4)*cos(e6)^2*sin(e5) + 2*m6*x6*z6*cos(e5)^2*cos(e6)*sin(e4) - 2*m6*y6*z6*cos(e5)^2*sin(e4)*sin(e6) + m6*x6^2*cos(e4)*cos(e6)*sin(e5)*sin(e6) - m6*y6^2*cos(e4)*cos(e6)*sin(e5)*sin(e6) - 2*m6*x6*y6*cos(e5)*cos(e6)*sin(e4)*sin(e5)*sin(e6),I5xx/2 + I5yy/2 + I6yy/2 + I4zz + I6zz/2 + m4*x4^2 + (m5*x5^2)/2 + m6*x6^2 + m4*y4^2 + (m5*y5^2)/2 + (m6*y6^2)/2 + m5*z5^2 + (m6*z6^2)/2 - (I5xx*cos(2*e5))/2 + (I5yy*cos(2*e5))/2 - (I6yy*cos(2*e5))/2 + (I6zz*cos(2*e5))/2 + (I6xx*cos(e6)^2)/2 - (I6yy*cos(e6)^2)/2 + (m5*x5^2*cos(2*e5))/2 - (m6*x6^2*cos(e6)^2)/2 - (m5*y5^2*cos(2*e5))/2 + (m6*y6^2*cos(2*e5))/2 + (m6*y6^2*cos(e6)^2)/2 - (m6*z6^2*cos(2*e5))/2 - (I6xx*cos(2*e5)*cos(e6)^2)/2 + (I6yy*cos(2*e5)*cos(e6)^2)/2 + (m6*x6^2*cos(2*e5)*cos(e6)^2)/2 - (m6*y6^2*cos(2*e5)*cos(e6)^2)/2 - m5*x5*y5*sin(2*e5) + (m6*x6*y6*sin(2*e6))/2 - m6*x6*z6*sin(2*e5)*cos(e6) + m6*y6*z6*sin(2*e5)*sin(e6) - m6*x6*y6*cos(2*e5)*cos(e6)*sin(e6),I6yy*cos(e6)*sin(e5)*sin(e6) - I6xx*cos(e6)*sin(e5)*sin(e6) - m5*y5*z5*cos(e5) - m6*x6*y6*sin(e5) - m5*x5*z5*sin(e5) + m6*x6^2*cos(e6)*sin(e5)*sin(e6) - m6*y6^2*cos(e6)*sin(e5)*sin(e6) + m6*y6*z6*cos(e5)*cos(e6) + m6*x6*z6*cos(e5)*sin(e6) + 2*m6*x6*y6*cos(e6)^2*sin(e5),I6zz*cos(e5) + m6*x6^2*cos(e5) + m6*y6^2*cos(e5) - m6*x6*z6*cos(e6)*sin(e5) + m6*y6*z6*sin(e5)*sin(e6);
 I6xx*cos(e2)*cos(e3)*sin(e4) + I5zz*cos(e2)*cos(e3)*sin(e4) - I6xx*sin(e2)*sin(e3)*sin(e4) - I5zz*sin(e2)*sin(e3)*sin(e4) + m5*x5^2*cos(e2)*cos(e3)*sin(e4) + m5*y5^2*cos(e2)*cos(e3)*sin(e4) + m6*y6^2*cos(e2)*cos(e3)*sin(e4) + m6*z6^2*cos(e2)*cos(e3)*sin(e4) - m5*x5^2*sin(e2)*sin(e3)*sin(e4) - m5*y5^2*sin(e2)*sin(e3)*sin(e4) - m6*y6^2*sin(e2)*sin(e3)*sin(e4) - m6*z6^2*sin(e2)*sin(e3)*sin(e4) - I6xx*cos(e2)*cos(e3)*cos(e6)^2*sin(e4) + I6yy*cos(e2)*cos(e3)*cos(e6)^2*sin(e4) + a1*m5*y5*cos(e5)*sin(e4) + a1*m6*z6*cos(e5)*sin(e4) + a1*m5*x5*sin(e4)*sin(e5) + I6xx*cos(e6)^2*sin(e2)*sin(e3)*sin(e4) - I6yy*cos(e6)^2*sin(e2)*sin(e3)*sin(e4) + a1*m6*x6*cos(e6)*sin(e4)*sin(e5) + a2*m5*y5*cos(e5)*sin(e2)*sin(e4) + a2*m6*z6*cos(e5)*sin(e2)*sin(e4) + m5*y5*z5*cos(e2)*cos(e5)*sin(e3) + m5*y5*z5*cos(e3)*cos(e5)*sin(e2) + a2*m5*x5*sin(e2)*sin(e4)*sin(e5) - a1*m6*y6*sin(e4)*sin(e5)*sin(e6) + m6*x6^2*cos(e2)*cos(e3)*cos(e6)^2*sin(e4) - m6*y6^2*cos(e2)*cos(e3)*cos(e6)^2*sin(e4) + m6*x6*y6*cos(e2)*sin(e3)*sin(e5) + m6*x6*y6*cos(e3)*sin(e2)*sin(e5) + m5*x5*z5*cos(e2)*sin(e3)*sin(e5) + m5*x5*z5*cos(e3)*sin(e2)*sin(e5) - m6*x6^2*cos(e6)^2*sin(e2)*sin(e3)*sin(e4) + m6*y6^2*cos(e6)^2*sin(e2)*sin(e3)*sin(e4) + I6xx*cos(e2)*cos(e6)*sin(e3)*sin(e5)*sin(e6) + I6xx*cos(e3)*cos(e6)*sin(e2)*sin(e5)*sin(e6) - I6yy*cos(e2)*cos(e6)*sin(e3)*sin(e5)*sin(e6) - I6yy*cos(e3)*cos(e6)*sin(e2)*sin(e5)*sin(e6) + m5*x5*z5*cos(e4)*cos(e5)*sin(e2)*sin(e3) - m6*x6*z6*cos(e2)*cos(e5)*sin(e3)*sin(e6) - m6*x6*z6*cos(e3)*cos(e5)*sin(e2)*sin(e6) - a2*m6*y6*sin(e2)*sin(e4)*sin(e5)*sin(e6) - d4*m5*x5*sin(e2)*sin(e3)*sin(e4)*sin(e5) - m5*y5*z5*cos(e4)*sin(e2)*sin(e3)*sin(e5) - 2*m6*x6*y6*cos(e2)*cos(e6)^2*sin(e3)*sin(e5) - 2*m6*x6*y6*cos(e3)*cos(e6)^2*sin(e2)*sin(e5) - I6xx*cos(e2)*cos(e3)*cos(e4)*cos(e5)*cos(e6)*sin(e6) + I6yy*cos(e2)*cos(e3)*cos(e4)*cos(e5)*cos(e6)*sin(e6) + I6xx*cos(e4)*cos(e5)*cos(e6)*sin(e2)*sin(e3)*sin(e6) - I6yy*cos(e4)*cos(e5)*cos(e6)*sin(e2)*sin(e3)*sin(e6) - m6*x6^2*cos(e2)*cos(e6)*sin(e3)*sin(e5)*sin(e6) - m6*x6^2*cos(e3)*cos(e6)*sin(e2)*sin(e5)*sin(e6) + m6*y6^2*cos(e2)*cos(e6)*sin(e3)*sin(e5)*sin(e6) + m6*y6^2*cos(e3)*cos(e6)*sin(e2)*sin(e5)*sin(e6) + d4*m5*y5*cos(e2)*cos(e3)*cos(e5)*sin(e4) + d4*m6*z6*cos(e2)*cos(e3)*cos(e5)*sin(e4) - m6*x6*y6*cos(e2)*cos(e3)*cos(e4)*cos(e5) - m5*x5*z5*cos(e2)*cos(e3)*cos(e4)*cos(e5) + a3*m5*y5*cos(e2)*cos(e5)*sin(e3)*sin(e4) + a3*m5*y5*cos(e3)*cos(e5)*sin(e2)*sin(e4) + a3*m6*z6*cos(e2)*cos(e5)*sin(e3)*sin(e4) + a3*m6*z6*cos(e3)*cos(e5)*sin(e2)*sin(e4) + d4*m5*x5*cos(e2)*cos(e3)*sin(e4)*sin(e5) + m5*y5*z5*cos(e2)*cos(e3)*cos(e4)*sin(e5) - m6*y6*z6*cos(e2)*cos(e5)*cos(e6)*sin(e3) - m6*y6*z6*cos(e3)*cos(e5)*cos(e6)*sin(e2) + a3*m5*x5*cos(e2)*sin(e3)*sin(e4)*sin(e5) + a3*m5*x5*cos(e3)*sin(e2)*sin(e4)*sin(e5) + a2*m6*x6*cos(e6)*sin(e2)*sin(e4)*sin(e5) - d4*m5*y5*cos(e5)*sin(e2)*sin(e3)*sin(e4) - d4*m6*z6*cos(e5)*sin(e2)*sin(e3)*sin(e4) + m6*x6*y6*cos(e4)*cos(e5)*sin(e2)*sin(e3) + 2*m6*x6*y6*cos(e2)*cos(e3)*cos(e4)*cos(e5)*cos(e6)^2 - 2*m6*x6*y6*cos(e4)*cos(e5)*cos(e6)^2*sin(e2)*sin(e3) + m6*x6^2*cos(e2)*cos(e3)*cos(e4)*cos(e5)*cos(e6)*sin(e6) - m6*y6^2*cos(e2)*cos(e3)*cos(e4)*cos(e5)*cos(e6)*sin(e6) - m6*x6^2*cos(e4)*cos(e5)*cos(e6)*sin(e2)*sin(e3)*sin(e6) + m6*y6^2*cos(e4)*cos(e5)*cos(e6)*sin(e2)*sin(e3)*sin(e6) + d4*m6*x6*cos(e2)*cos(e3)*cos(e6)*sin(e4)*sin(e5) - m6*y6*z6*cos(e2)*cos(e3)*cos(e4)*cos(e6)*sin(e5) + a3*m6*x6*cos(e2)*cos(e6)*sin(e3)*sin(e4)*sin(e5) + a3*m6*x6*cos(e3)*cos(e6)*sin(e2)*sin(e4)*sin(e5) - d4*m6*y6*cos(e2)*cos(e3)*sin(e4)*sin(e5)*sin(e6) - 2*m6*x6*y6*cos(e2)*cos(e3)*cos(e6)*sin(e4)*sin(e6) - m6*x6*z6*cos(e2)*cos(e3)*cos(e4)*sin(e5)*sin(e6) - a3*m6*y6*cos(e2)*sin(e3)*sin(e4)*sin(e5)*sin(e6) - a3*m6*y6*cos(e3)*sin(e2)*sin(e4)*sin(e5)*sin(e6) - d4*m6*x6*cos(e6)*sin(e2)*sin(e3)*sin(e4)*sin(e5) + m6*y6*z6*cos(e4)*cos(e6)*sin(e2)*sin(e3)*sin(e5) + d4*m6*y6*sin(e2)*sin(e3)*sin(e4)*sin(e5)*sin(e6) + 2*m6*x6*y6*cos(e6)*sin(e2)*sin(e3)*sin(e4)*sin(e6) + m6*x6*z6*cos(e4)*sin(e2)*sin(e3)*sin(e5)*sin(e6),I6xx*cos(e4) + I5zz*cos(e4) + m5*x5^2*cos(e4) + m5*y5^2*cos(e4) + m6*y6^2*cos(e4) + m6*z6^2*cos(e4) - I6xx*cos(e4)*cos(e6)^2 + I6yy*cos(e4)*cos(e6)^2 + a3*m5*x5*cos(e5) - a3*m5*y5*sin(e5) - a3*m6*z6*sin(e5) + m6*x6^2*cos(e4)*cos(e6)^2 - m6*y6^2*cos(e4)*cos(e6)^2 + a2*m5*x5*cos(e3)*cos(e5) + a3*m6*x6*cos(e5)*cos(e6) + d4*m5*y5*cos(e4)*cos(e5) + d4*m6*z6*cos(e4)*cos(e5) - a2*m5*y5*cos(e3)*sin(e5) - a3*m6*y6*cos(e5)*sin(e6) - a2*m6*z6*cos(e3)*sin(e5) + d4*m5*x5*cos(e4)*sin(e5) + m6*x6*y6*cos(e5)*sin(e4) + m5*x5*z5*cos(e5)*sin(e4) - m5*y5*z5*sin(e4)*sin(e5) + I6xx*cos(e5)*cos(e6)*sin(e4)*sin(e6) - I6yy*cos(e5)*cos(e6)*sin(e4)*sin(e6) - a2*m5*y5*cos(e4)*cos(e5)*sin(e3) - a2*m6*y6*cos(e3)*cos(e5)*sin(e6) - a2*m6*z6*cos(e4)*cos(e5)*sin(e3) + d4*m6*x6*cos(e4)*cos(e6)*sin(e5) - a2*m5*x5*cos(e4)*sin(e3)*sin(e5) - d4*m6*y6*cos(e4)*sin(e5)*sin(e6) - 2*m6*x6*y6*cos(e4)*cos(e6)*sin(e6) + m6*y6*z6*cos(e6)*sin(e4)*sin(e5) + m6*x6*z6*sin(e4)*sin(e5)*sin(e6) - 2*m6*x6*y6*cos(e5)*cos(e6)^2*sin(e4) - m6*x6^2*cos(e5)*cos(e6)*sin(e4)*sin(e6) + m6*y6^2*cos(e5)*cos(e6)*sin(e4)*sin(e6) + a2*m6*x6*cos(e3)*cos(e5)*cos(e6) - a2*m6*x6*cos(e4)*cos(e6)*sin(e3)*sin(e5) + a2*m6*y6*cos(e4)*sin(e3)*sin(e5)*sin(e6),I6xx*cos(e4) + I5zz*cos(e4) + m5*x5^2*cos(e4) + m5*y5^2*cos(e4) + m6*y6^2*cos(e4) + m6*z6^2*cos(e4) - I6xx*cos(e4)*cos(e6)^2 + I6yy*cos(e4)*cos(e6)^2 + a3*m5*x5*cos(e5) - a3*m5*y5*sin(e5) - a3*m6*z6*sin(e5) + m6*x6^2*cos(e4)*cos(e6)^2 - m6*y6^2*cos(e4)*cos(e6)^2 + a3*m6*x6*cos(e5)*cos(e6) + d4*m5*y5*cos(e4)*cos(e5) + d4*m6*z6*cos(e4)*cos(e5) - a3*m6*y6*cos(e5)*sin(e6) + d4*m5*x5*cos(e4)*sin(e5) + m6*x6*y6*cos(e5)*sin(e4) + m5*x5*z5*cos(e5)*sin(e4) - m5*y5*z5*sin(e4)*sin(e5) + I6xx*cos(e5)*cos(e6)*sin(e4)*sin(e6) - I6yy*cos(e5)*cos(e6)*sin(e4)*sin(e6) + d4*m6*x6*cos(e4)*cos(e6)*sin(e5) - d4*m6*y6*cos(e4)*sin(e5)*sin(e6) - 2*m6*x6*y6*cos(e4)*cos(e6)*sin(e6) + m6*y6*z6*cos(e6)*sin(e4)*sin(e5) + m6*x6*z6*sin(e4)*sin(e5)*sin(e6) - 2*m6*x6*y6*cos(e5)*cos(e6)^2*sin(e4) - m6*x6^2*cos(e5)*cos(e6)*sin(e4)*sin(e6) + m6*y6^2*cos(e5)*cos(e6)*sin(e4)*sin(e6),I6yy*cos(e6)*sin(e5)*sin(e6) - I6xx*cos(e6)*sin(e5)*sin(e6) - m5*y5*z5*cos(e5) - m6*x6*y6*sin(e5) - m5*x5*z5*sin(e5) + m6*x6^2*cos(e6)*sin(e5)*sin(e6) - m6*y6^2*cos(e6)*sin(e5)*sin(e6) + m6*y6*z6*cos(e5)*cos(e6) + m6*x6*z6*cos(e5)*sin(e6) + 2*m6*x6*y6*cos(e6)^2*sin(e5),I6xx/2 + I6yy/2 + I5zz + m5*x5^2 + (m6*x6^2)/2 + m5*y5^2 + (m6*y6^2)/2 + m6*z6^2 - (I6xx*cos(2*e6))/2 + (I6yy*cos(2*e6))/2 + (m6*x6^2*cos(2*e6))/2 - (m6*y6^2*cos(2*e6))/2 - m6*x6*y6*sin(2*e6),m6*z6*(y6*cos(e6) + x6*sin(e6));
 a1*m6*y6*cos(e4)*sin(e6) - I6zz*cos(e3)*cos(e5)*sin(e2) - m6*x6^2*cos(e2)*cos(e5)*sin(e3) - m6*x6^2*cos(e3)*cos(e5)*sin(e2) - m6*y6^2*cos(e2)*cos(e5)*sin(e3) - m6*y6^2*cos(e3)*cos(e5)*sin(e2) - a1*m6*x6*cos(e4)*cos(e6) - I6zz*cos(e2)*cos(e5)*sin(e3) - I6zz*cos(e2)*cos(e3)*cos(e4)*sin(e5) + I6zz*cos(e4)*sin(e2)*sin(e3)*sin(e5) - a2*m6*x6*cos(e4)*cos(e6)*sin(e2) + a1*m6*y6*cos(e5)*cos(e6)*sin(e4) + a1*m6*x6*cos(e5)*sin(e4)*sin(e6) + a2*m6*y6*cos(e4)*sin(e2)*sin(e6) - m6*x6^2*cos(e2)*cos(e3)*cos(e4)*sin(e5) - m6*y6^2*cos(e2)*cos(e3)*cos(e4)*sin(e5) + m6*x6^2*cos(e4)*sin(e2)*sin(e3)*sin(e5) + m6*y6^2*cos(e4)*sin(e2)*sin(e3)*sin(e5) + m6*x6*z6*cos(e2)*cos(e3)*sin(e4)*sin(e6) + m6*x6*z6*cos(e2)*cos(e6)*sin(e3)*sin(e5) + m6*x6*z6*cos(e3)*cos(e6)*sin(e2)*sin(e5) - m6*y6*z6*cos(e6)*sin(e2)*sin(e3)*sin(e4) - m6*y6*z6*cos(e2)*sin(e3)*sin(e5)*sin(e6) - m6*y6*z6*cos(e3)*sin(e2)*sin(e5)*sin(e6) - m6*x6*z6*sin(e2)*sin(e3)*sin(e4)*sin(e6) - d4*m6*x6*cos(e2)*cos(e3)*cos(e4)*cos(e6) - a3*m6*x6*cos(e2)*cos(e4)*cos(e6)*sin(e3) - a3*m6*x6*cos(e3)*cos(e4)*cos(e6)*sin(e2) + d4*m6*y6*cos(e2)*cos(e3)*cos(e4)*sin(e6) + a3*m6*y6*cos(e2)*cos(e4)*sin(e3)*sin(e6) + a3*m6*y6*cos(e3)*cos(e4)*sin(e2)*sin(e6) + a2*m6*y6*cos(e5)*cos(e6)*sin(e2)*sin(e4) + d4*m6*x6*cos(e4)*cos(e6)*sin(e2)*sin(e3) + m6*y6*z6*cos(e2)*cos(e3)*cos(e6)*sin(e4) + a2*m6*x6*cos(e5)*sin(e2)*sin(e4)*sin(e6) - d4*m6*y6*cos(e4)*sin(e2)*sin(e3)*sin(e6) + d4*m6*y6*cos(e2)*cos(e3)*cos(e5)*cos(e6)*sin(e4) - m6*x6*z6*cos(e2)*cos(e3)*cos(e4)*cos(e5)*cos(e6) + a3*m6*y6*cos(e2)*cos(e5)*cos(e6)*sin(e3)*sin(e4) + a3*m6*y6*cos(e3)*cos(e5)*cos(e6)*sin(e2)*sin(e4) + d4*m6*x6*cos(e2)*cos(e3)*cos(e5)*sin(e4)*sin(e6) + m6*y6*z6*cos(e2)*cos(e3)*cos(e4)*cos(e5)*sin(e6) + a3*m6*x6*cos(e2)*cos(e5)*sin(e3)*sin(e4)*sin(e6) + a3*m6*x6*cos(e3)*cos(e5)*sin(e2)*sin(e4)*sin(e6) - d4*m6*y6*cos(e5)*cos(e6)*sin(e2)*sin(e3)*sin(e4) + m6*x6*z6*cos(e4)*cos(e5)*cos(e6)*sin(e2)*sin(e3) - d4*m6*x6*cos(e5)*sin(e2)*sin(e3)*sin(e4)*sin(e6) - m6*y6*z6*cos(e4)*cos(e5)*sin(e2)*sin(e3)*sin(e6),I6zz*sin(e4)*sin(e5) + m6*x6^2*sin(e4)*sin(e5) + m6*y6^2*sin(e4)*sin(e5) - a3*m6*y6*cos(e6)*sin(e5) + d4*m6*x6*cos(e6)*sin(e4) + m6*y6*z6*cos(e4)*cos(e6) - a3*m6*x6*sin(e5)*sin(e6) - d4*m6*y6*sin(e4)*sin(e6) + m6*x6*z6*cos(e4)*sin(e6) + d4*m6*y6*cos(e4)*cos(e5)*cos(e6) - a2*m6*y6*cos(e3)*cos(e6)*sin(e5) + d4*m6*x6*cos(e4)*cos(e5)*sin(e6) - a2*m6*x6*cos(e6)*sin(e3)*sin(e4) - a2*m6*x6*cos(e3)*sin(e5)*sin(e6) + m6*x6*z6*cos(e5)*cos(e6)*sin(e4) + a2*m6*y6*sin(e3)*sin(e4)*sin(e6) - m6*y6*z6*cos(e5)*sin(e4)*sin(e6) - a2*m6*y6*cos(e4)*cos(e5)*cos(e6)*sin(e3) - a2*m6*x6*cos(e4)*cos(e5)*sin(e3)*sin(e6),I6zz*sin(e4)*sin(e5) + m6*x6^2*sin(e4)*sin(e5) + m6*y6^2*sin(e4)*sin(e5) - a3*m6*y6*cos(e6)*sin(e5) + d4*m6*x6*cos(e6)*sin(e4) + m6*y6*z6*cos(e4)*cos(e6) - a3*m6*x6*sin(e5)*sin(e6) - d4*m6*y6*sin(e4)*sin(e6) + m6*x6*z6*cos(e4)*sin(e6) + d4*m6*y6*cos(e4)*cos(e5)*cos(e6) + d4*m6*x6*cos(e4)*cos(e5)*sin(e6) + m6*x6*z6*cos(e5)*cos(e6)*sin(e4) - m6*y6*z6*cos(e5)*sin(e4)*sin(e6),I6zz*cos(e5) + m6*x6^2*cos(e5) + m6*y6^2*cos(e5) - m6*x6*z6*cos(e6)*sin(e5) + m6*y6*z6*sin(e5)*sin(e6),m6*z6*(y6*cos(e6) + x6*sin(e6)),I6zz + m6*x6^2 + m6*y6^2];


C11 = de6*(2*m6*(x6*cos(e1)*cos(e4)*cos(e6) - y6*cos(e1)*cos(e4)*sin(e6) - y6*cos(e1)*cos(e5)*cos(e6)*sin(e4) - x6*cos(e1)*cos(e5)*sin(e4)*sin(e6) - y6*cos(e2)*sin(e1)*sin(e3)*sin(e4)*sin(e6) - y6*cos(e3)*sin(e1)*sin(e2)*sin(e4)*sin(e6) - y6*cos(e6)*sin(e1)*sin(e2)*sin(e3)*sin(e5) - x6*sin(e1)*sin(e2)*sin(e3)*sin(e5)*sin(e6) + y6*cos(e2)*cos(e3)*cos(e6)*sin(e1)*sin(e5) + x6*cos(e2)*cos(e6)*sin(e1)*sin(e3)*sin(e4) + x6*cos(e3)*cos(e6)*sin(e1)*sin(e2)*sin(e4) + x6*cos(e2)*cos(e3)*sin(e1)*sin(e5)*sin(e6) + y6*cos(e2)*cos(e4)*cos(e5)*cos(e6)*sin(e1)*sin(e3) + y6*cos(e3)*cos(e4)*cos(e5)*cos(e6)*sin(e1)*sin(e2) + x6*cos(e2)*cos(e4)*cos(e5)*sin(e1)*sin(e3)*sin(e6) + x6*cos(e3)*cos(e4)*cos(e5)*sin(e1)*sin(e2)*sin(e6))*(y6*cos(e1)*cos(e4)*cos(e6) - a2*sin(e1)*sin(e2) - d4*cos(e2)*cos(e3)*sin(e1) - a1*sin(e1) - a3*cos(e2)*sin(e1)*sin(e3) - a3*cos(e3)*sin(e1)*sin(e2) + x6*cos(e1)*cos(e4)*sin(e6) + d4*sin(e1)*sin(e2)*sin(e3) - z6*cos(e1)*sin(e4)*sin(e5) + x6*cos(e1)*cos(e5)*cos(e6)*sin(e4) - z6*cos(e2)*cos(e3)*cos(e5)*sin(e1) - y6*cos(e1)*cos(e5)*sin(e4)*sin(e6) + z6*cos(e5)*sin(e1)*sin(e2)*sin(e3) + x6*cos(e2)*sin(e1)*sin(e3)*sin(e4)*sin(e6) + x6*cos(e3)*sin(e1)*sin(e2)*sin(e4)*sin(e6) + x6*cos(e6)*sin(e1)*sin(e2)*sin(e3)*sin(e5) - y6*sin(e1)*sin(e2)*sin(e3)*sin(e5)*sin(e6) - x6*cos(e2)*cos(e3)*cos(e6)*sin(e1)*sin(e5) + y6*cos(e2)*cos(e6)*sin(e1)*sin(e3)*sin(e4) + y6*cos(e3)*cos(e6)*sin(e1)*sin(e2)*sin(e4) + y6*cos(e2)*cos(e3)*sin(e1)*sin(e5)*sin(e6) + z6*cos(e2)*cos(e4)*sin(e1)*sin(e3)*sin(e5) + z6*cos(e3)*cos(e4)*sin(e1)*sin(e2)*sin(e5) - x6*cos(e2)*cos(e4)*cos(e5)*cos(e6)*sin(e1)*sin(e3) - x6*cos(e3)*cos(e4)*cos(e5)*cos(e6)*sin(e1)*sin(e2) + y6*cos(e2)*cos(e4)*cos(e5)*sin(e1)*sin(e3)*sin(e6) + y6*cos(e3)*cos(e4)*cos(e5)*sin(e1)*sin(e2)*sin(e6)) + 2*I6xx*(cos(e2 + e3)*sin(e4)*sin(e6) + sin(e2 + e3)*cos(e6)*sin(e5) - cos(e2 + e3)*cos(e4)*cos(e5)*cos(e6))*(cos(e2 + e3)*cos(e6)*sin(e4) - sin(e2 + e3)*sin(e5)*sin(e6) + cos(e2 + e3)*cos(e4)*cos(e5)*sin(e6)) - 2*I6yy*(cos(e2 + e3)*sin(e4)*sin(e6) + sin(e2 + e3)*cos(e6)*sin(e5) - cos(e2 + e3)*cos(e4)*cos(e5)*cos(e6))*(cos(e2 + e3)*cos(e6)*sin(e4) - sin(e2 + e3)*sin(e5)*sin(e6) + cos(e2 + e3)*cos(e4)*cos(e5)*sin(e6)) + 2*m6*(y6*cos(e4)*sin(e1)*sin(e6) - x6*cos(e4)*cos(e6)*sin(e1) + y6*cos(e5)*cos(e6)*sin(e1)*sin(e4) + x6*cos(e5)*sin(e1)*sin(e4)*sin(e6) - x6*cos(e1)*sin(e2)*sin(e3)*sin(e5)*sin(e6) + y6*cos(e1)*cos(e2)*cos(e3)*cos(e6)*sin(e5) + x6*cos(e1)*cos(e2)*cos(e6)*sin(e3)*sin(e4) + x6*cos(e1)*cos(e3)*cos(e6)*sin(e2)*sin(e4) + x6*cos(e1)*cos(e2)*cos(e3)*sin(e5)*sin(e6) - y6*cos(e1)*cos(e2)*sin(e3)*sin(e4)*sin(e6) - y6*cos(e1)*cos(e3)*sin(e2)*sin(e4)*sin(e6) - y6*cos(e1)*cos(e6)*sin(e2)*sin(e3)*sin(e5) + y6*cos(e1)*cos(e2)*cos(e4)*cos(e5)*cos(e6)*sin(e3) + y6*cos(e1)*cos(e3)*cos(e4)*cos(e5)*cos(e6)*sin(e2) + x6*cos(e1)*cos(e2)*cos(e4)*cos(e5)*sin(e3)*sin(e6) + x6*cos(e1)*cos(e3)*cos(e4)*cos(e5)*sin(e2)*sin(e6))*(d4*cos(e1)*sin(e2)*sin(e3) - a2*cos(e1)*sin(e2) - d4*cos(e1)*cos(e2)*cos(e3) - a3*cos(e1)*cos(e2)*sin(e3) - a3*cos(e1)*cos(e3)*sin(e2) - a1*cos(e1) - y6*cos(e4)*cos(e6)*sin(e1) - x6*cos(e4)*sin(e1)*sin(e6) + z6*sin(e1)*sin(e4)*sin(e5) - x6*cos(e5)*cos(e6)*sin(e1)*sin(e4) + z6*cos(e1)*cos(e5)*sin(e2)*sin(e3) + y6*cos(e5)*sin(e1)*sin(e4)*sin(e6) - z6*cos(e1)*cos(e2)*cos(e3)*cos(e5) - y6*cos(e1)*sin(e2)*sin(e3)*sin(e5)*sin(e6) - x6*cos(e1)*cos(e2)*cos(e3)*cos(e6)*sin(e5) + y6*cos(e1)*cos(e2)*cos(e6)*sin(e3)*sin(e4) + y6*cos(e1)*cos(e3)*cos(e6)*sin(e2)*sin(e4) + y6*cos(e1)*cos(e2)*cos(e3)*sin(e5)*sin(e6) + z6*cos(e1)*cos(e2)*cos(e4)*sin(e3)*sin(e5) + z6*cos(e1)*cos(e3)*cos(e4)*sin(e2)*sin(e5) + x6*cos(e1)*cos(e2)*sin(e3)*sin(e4)*sin(e6) + x6*cos(e1)*cos(e3)*sin(e2)*sin(e4)*sin(e6) + x6*cos(e1)*cos(e6)*sin(e2)*sin(e3)*sin(e5) - x6*cos(e1)*cos(e2)*cos(e4)*cos(e5)*cos(e6)*sin(e3) - x6*cos(e1)*cos(e3)*cos(e4)*cos(e5)*cos(e6)*sin(e2) + y6*cos(e1)*cos(e2)*cos(e4)*cos(e5)*sin(e3)*sin(e6) + y6*cos(e1)*cos(e3)*cos(e4)*cos(e5)*sin(e2)*sin(e6))) - de5*(2*I5yy*(sin(e2 + e3)*cos(e5) + cos(e2 + e3)*cos(e4)*sin(e5))*(sin(e2 + e3)*sin(e5) - cos(e2 + e3)*cos(e4)*cos(e5)) - 2*I5xx*(sin(e2 + e3)*cos(e5) + cos(e2 + e3)*cos(e4)*sin(e5))*(sin(e2 + e3)*sin(e5) - cos(e2 + e3)*cos(e4)*cos(e5)) + 2*I6zz*(sin(e2 + e3)*cos(e5) + cos(e2 + e3)*cos(e4)*sin(e5))*(sin(e2 + e3)*sin(e5) - cos(e2 + e3)*cos(e4)*cos(e5)) - 2*m6*(z6*cos(e2)*cos(e3)*sin(e1)*sin(e5) - x6*cos(e1)*cos(e6)*sin(e4)*sin(e5) - z6*cos(e1)*cos(e5)*sin(e4) + y6*cos(e1)*sin(e4)*sin(e5)*sin(e6) - z6*sin(e1)*sin(e2)*sin(e3)*sin(e5) - y6*cos(e5)*sin(e1)*sin(e2)*sin(e3)*sin(e6) - x6*cos(e2)*cos(e3)*cos(e5)*cos(e6)*sin(e1) + y6*cos(e2)*cos(e3)*cos(e5)*sin(e1)*sin(e6) + z6*cos(e2)*cos(e4)*cos(e5)*sin(e1)*sin(e3) + z6*cos(e3)*cos(e4)*cos(e5)*sin(e1)*sin(e2) + x6*cos(e5)*cos(e6)*sin(e1)*sin(e2)*sin(e3) + x6*cos(e2)*cos(e4)*cos(e6)*sin(e1)*sin(e3)*sin(e5) + x6*cos(e3)*cos(e4)*cos(e6)*sin(e1)*sin(e2)*sin(e5) - y6*cos(e2)*cos(e4)*sin(e1)*sin(e3)*sin(e5)*sin(e6) - y6*cos(e3)*cos(e4)*sin(e1)*sin(e2)*sin(e5)*sin(e6))*(y6*cos(e1)*cos(e4)*cos(e6) - a2*sin(e1)*sin(e2) - d4*cos(e2)*cos(e3)*sin(e1) - a1*sin(e1) - a3*cos(e2)*sin(e1)*sin(e3) - a3*cos(e3)*sin(e1)*sin(e2) + x6*cos(e1)*cos(e4)*sin(e6) + d4*sin(e1)*sin(e2)*sin(e3) - z6*cos(e1)*sin(e4)*sin(e5) + x6*cos(e1)*cos(e5)*cos(e6)*sin(e4) - z6*cos(e2)*cos(e3)*cos(e5)*sin(e1) - y6*cos(e1)*cos(e5)*sin(e4)*sin(e6) + z6*cos(e5)*sin(e1)*sin(e2)*sin(e3) + x6*cos(e2)*sin(e1)*sin(e3)*sin(e4)*sin(e6) + x6*cos(e3)*sin(e1)*sin(e2)*sin(e4)*sin(e6) + x6*cos(e6)*sin(e1)*sin(e2)*sin(e3)*sin(e5) - y6*sin(e1)*sin(e2)*sin(e3)*sin(e5)*sin(e6) - x6*cos(e2)*cos(e3)*cos(e6)*sin(e1)*sin(e5) + y6*cos(e2)*cos(e6)*sin(e1)*sin(e3)*sin(e4) + y6*cos(e3)*cos(e6)*sin(e1)*sin(e2)*sin(e4) + y6*cos(e2)*cos(e3)*sin(e1)*sin(e5)*sin(e6) + z6*cos(e2)*cos(e4)*sin(e1)*sin(e3)*sin(e5) + z6*cos(e3)*cos(e4)*sin(e1)*sin(e2)*sin(e5) - x6*cos(e2)*cos(e4)*cos(e5)*cos(e6)*sin(e1)*sin(e3) - x6*cos(e3)*cos(e4)*cos(e5)*cos(e6)*sin(e1)*sin(e2) + y6*cos(e2)*cos(e4)*cos(e5)*sin(e1)*sin(e3)*sin(e6) + y6*cos(e3)*cos(e4)*cos(e5)*sin(e1)*sin(e2)*sin(e6)) + 2*m5*(y5*cos(e5)*sin(e1)*sin(e4) + x5*sin(e1)*sin(e4)*sin(e5) + y5*cos(e1)*cos(e2)*cos(e3)*sin(e5) + x5*cos(e1)*cos(e5)*sin(e2)*sin(e3) - y5*cos(e1)*sin(e2)*sin(e3)*sin(e5) - x5*cos(e1)*cos(e2)*cos(e3)*cos(e5) + y5*cos(e1)*cos(e2)*cos(e4)*cos(e5)*sin(e3) + y5*cos(e1)*cos(e3)*cos(e4)*cos(e5)*sin(e2) + x5*cos(e1)*cos(e2)*cos(e4)*sin(e3)*sin(e5) + x5*cos(e1)*cos(e3)*cos(e4)*sin(e2)*sin(e5))*(a1*cos(e1) + a2*cos(e1)*sin(e2) - z5*cos(e4)*sin(e1) + d4*cos(e1)*cos(e2)*cos(e3) + a3*cos(e1)*cos(e2)*sin(e3) + a3*cos(e1)*cos(e3)*sin(e2) - d4*cos(e1)*sin(e2)*sin(e3) + x5*cos(e5)*sin(e1)*sin(e4) - y5*sin(e1)*sin(e4)*sin(e5) + x5*cos(e1)*cos(e2)*cos(e3)*sin(e5) - y5*cos(e1)*cos(e5)*sin(e2)*sin(e3) + z5*cos(e1)*cos(e2)*sin(e3)*sin(e4) + z5*cos(e1)*cos(e3)*sin(e2)*sin(e4) - x5*cos(e1)*sin(e2)*sin(e3)*sin(e5) + y5*cos(e1)*cos(e2)*cos(e3)*cos(e5) + x5*cos(e1)*cos(e2)*cos(e4)*cos(e5)*sin(e3) + x5*cos(e1)*cos(e3)*cos(e4)*cos(e5)*sin(e2) - y5*cos(e1)*cos(e2)*cos(e4)*sin(e3)*sin(e5) - y5*cos(e1)*cos(e3)*cos(e4)*sin(e2)*sin(e5)) + 2*m5*(y5*cos(e2)*cos(e3)*sin(e1)*sin(e5) - x5*cos(e1)*sin(e4)*sin(e5) - x5*cos(e2)*cos(e3)*cos(e5)*sin(e1) - y5*cos(e1)*cos(e5)*sin(e4) + x5*cos(e5)*sin(e1)*sin(e2)*sin(e3) - y5*sin(e1)*sin(e2)*sin(e3)*sin(e5) + y5*cos(e2)*cos(e4)*cos(e5)*sin(e1)*sin(e3) + y5*cos(e3)*cos(e4)*cos(e5)*sin(e1)*sin(e2) + x5*cos(e2)*cos(e4)*sin(e1)*sin(e3)*sin(e5) + x5*cos(e3)*cos(e4)*sin(e1)*sin(e2)*sin(e5))*(a1*sin(e1) + z5*cos(e1)*cos(e4) + a2*sin(e1)*sin(e2) + d4*cos(e2)*cos(e3)*sin(e1) + a3*cos(e2)*sin(e1)*sin(e3) + a3*cos(e3)*sin(e1)*sin(e2) - x5*cos(e1)*cos(e5)*sin(e4) - d4*sin(e1)*sin(e2)*sin(e3) + y5*cos(e1)*sin(e4)*sin(e5) + y5*cos(e2)*cos(e3)*cos(e5)*sin(e1) + x5*cos(e2)*cos(e3)*sin(e1)*sin(e5) - y5*cos(e5)*sin(e1)*sin(e2)*sin(e3) + z5*cos(e2)*sin(e1)*sin(e3)*sin(e4) + z5*cos(e3)*sin(e1)*sin(e2)*sin(e4) - x5*sin(e1)*sin(e2)*sin(e3)*sin(e5) + x5*cos(e2)*cos(e4)*cos(e5)*sin(e1)*sin(e3) + x5*cos(e3)*cos(e4)*cos(e5)*sin(e1)*sin(e2) - y5*cos(e2)*cos(e4)*sin(e1)*sin(e3)*sin(e5) - y5*cos(e3)*cos(e4)*sin(e1)*sin(e2)*sin(e5)) - 2*m6*(z6*cos(e5)*sin(e1)*sin(e4) + z6*cos(e1)*cos(e2)*cos(e3)*sin(e5) + x6*cos(e6)*sin(e1)*sin(e4)*sin(e5) - z6*cos(e1)*sin(e2)*sin(e3)*sin(e5) - y6*sin(e1)*sin(e4)*sin(e5)*sin(e6) - x6*cos(e1)*cos(e2)*cos(e3)*cos(e5)*cos(e6) + y6*cos(e1)*cos(e2)*cos(e3)*cos(e5)*sin(e6) + z6*cos(e1)*cos(e2)*cos(e4)*cos(e5)*sin(e3) + z6*cos(e1)*cos(e3)*cos(e4)*cos(e5)*sin(e2) + x6*cos(e1)*cos(e5)*cos(e6)*sin(e2)*sin(e3) - y6*cos(e1)*cos(e5)*sin(e2)*sin(e3)*sin(e6) + x6*cos(e1)*cos(e2)*cos(e4)*cos(e6)*sin(e3)*sin(e5) + x6*cos(e1)*cos(e3)*cos(e4)*cos(e6)*sin(e2)*sin(e5) - y6*cos(e1)*cos(e2)*cos(e4)*sin(e3)*sin(e5)*sin(e6) - y6*cos(e1)*cos(e3)*cos(e4)*sin(e2)*sin(e5)*sin(e6))*(d4*cos(e1)*sin(e2)*sin(e3) - a2*cos(e1)*sin(e2) - d4*cos(e1)*cos(e2)*cos(e3) - a3*cos(e1)*cos(e2)*sin(e3) - a3*cos(e1)*cos(e3)*sin(e2) - a1*cos(e1) - y6*cos(e4)*cos(e6)*sin(e1) - x6*cos(e4)*sin(e1)*sin(e6) + z6*sin(e1)*sin(e4)*sin(e5) - x6*cos(e5)*cos(e6)*sin(e1)*sin(e4) + z6*cos(e1)*cos(e5)*sin(e2)*sin(e3) + y6*cos(e5)*sin(e1)*sin(e4)*sin(e6) - z6*cos(e1)*cos(e2)*cos(e3)*cos(e5) - y6*cos(e1)*sin(e2)*sin(e3)*sin(e5)*sin(e6) - x6*cos(e1)*cos(e2)*cos(e3)*cos(e6)*sin(e5) + y6*cos(e1)*cos(e2)*cos(e6)*sin(e3)*sin(e4) + y6*cos(e1)*cos(e3)*cos(e6)*sin(e2)*sin(e4) + y6*cos(e1)*cos(e2)*cos(e3)*sin(e5)*sin(e6) + z6*cos(e1)*cos(e2)*cos(e4)*sin(e3)*sin(e5) + z6*cos(e1)*cos(e3)*cos(e4)*sin(e2)*sin(e5) + x6*cos(e1)*cos(e2)*sin(e3)*sin(e4)*sin(e6) + x6*cos(e1)*cos(e3)*sin(e2)*sin(e4)*sin(e6) + x6*cos(e1)*cos(e6)*sin(e2)*sin(e3)*sin(e5) - x6*cos(e1)*cos(e2)*cos(e4)*cos(e5)*cos(e6)*sin(e3) - x6*cos(e1)*cos(e3)*cos(e4)*cos(e5)*cos(e6)*sin(e2) + y6*cos(e1)*cos(e2)*cos(e4)*cos(e5)*sin(e3)*sin(e6) + y6*cos(e1)*cos(e3)*cos(e4)*cos(e5)*sin(e2)*sin(e6)) - 2*I6xx*cos(e6)*(sin(e2 + e3)*cos(e5) + cos(e2 + e3)*cos(e4)*sin(e5))*(cos(e2 + e3)*sin(e4)*sin(e6) + sin(e2 + e3)*cos(e6)*sin(e5) - cos(e2 + e3)*cos(e4)*cos(e5)*cos(e6)) + 2*I6yy*sin(e6)*(sin(e2 + e3)*cos(e5) + cos(e2 + e3)*cos(e4)*sin(e5))*(cos(e2 + e3)*cos(e6)*sin(e4) - sin(e2 + e3)*sin(e5)*sin(e6) + cos(e2 + e3)*cos(e4)*cos(e5)*sin(e6))) + de4*(2*m5*(y5*cos(e1)*cos(e4)*sin(e5) - x5*cos(e1)*cos(e4)*cos(e5) - z5*cos(e1)*sin(e4) + z5*cos(e2)*cos(e4)*sin(e1)*sin(e3) + z5*cos(e3)*cos(e4)*sin(e1)*sin(e2) + y5*cos(e2)*sin(e1)*sin(e3)*sin(e4)*sin(e5) + y5*cos(e3)*sin(e1)*sin(e2)*sin(e4)*sin(e5) - x5*cos(e2)*cos(e5)*sin(e1)*sin(e3)*sin(e4) - x5*cos(e3)*cos(e5)*sin(e1)*sin(e2)*sin(e4))*(a1*sin(e1) + z5*cos(e1)*cos(e4) + a2*sin(e1)*sin(e2) + d4*cos(e2)*cos(e3)*sin(e1) + a3*cos(e2)*sin(e1)*sin(e3) + a3*cos(e3)*sin(e1)*sin(e2) - x5*cos(e1)*cos(e5)*sin(e4) - d4*sin(e1)*sin(e2)*sin(e3) + y5*cos(e1)*sin(e4)*sin(e5) + y5*cos(e2)*cos(e3)*cos(e5)*sin(e1) + x5*cos(e2)*cos(e3)*sin(e1)*sin(e5) - y5*cos(e5)*sin(e1)*sin(e2)*sin(e3) + z5*cos(e2)*sin(e1)*sin(e3)*sin(e4) + z5*cos(e3)*sin(e1)*sin(e2)*sin(e4) - x5*sin(e1)*sin(e2)*sin(e3)*sin(e5) + x5*cos(e2)*cos(e4)*cos(e5)*sin(e1)*sin(e3) + x5*cos(e3)*cos(e4)*cos(e5)*sin(e1)*sin(e2) - y5*cos(e2)*cos(e4)*sin(e1)*sin(e3)*sin(e5) - y5*cos(e3)*cos(e4)*sin(e1)*sin(e2)*sin(e5)) + 2*m5*(z5*sin(e1)*sin(e4) + x5*cos(e4)*cos(e5)*sin(e1) - y5*cos(e4)*sin(e1)*sin(e5) + z5*cos(e1)*cos(e2)*cos(e4)*sin(e3) + z5*cos(e1)*cos(e3)*cos(e4)*sin(e2) - x5*cos(e1)*cos(e2)*cos(e5)*sin(e3)*sin(e4) - x5*cos(e1)*cos(e3)*cos(e5)*sin(e2)*sin(e4) + y5*cos(e1)*cos(e2)*sin(e3)*sin(e4)*sin(e5) + y5*cos(e1)*cos(e3)*sin(e2)*sin(e4)*sin(e5))*(a1*cos(e1) + a2*cos(e1)*sin(e2) - z5*cos(e4)*sin(e1) + d4*cos(e1)*cos(e2)*cos(e3) + a3*cos(e1)*cos(e2)*sin(e3) + a3*cos(e1)*cos(e3)*sin(e2) - d4*cos(e1)*sin(e2)*sin(e3) + x5*cos(e5)*sin(e1)*sin(e4) - y5*sin(e1)*sin(e4)*sin(e5) + x5*cos(e1)*cos(e2)*cos(e3)*sin(e5) - y5*cos(e1)*cos(e5)*sin(e2)*sin(e3) + z5*cos(e1)*cos(e2)*sin(e3)*sin(e4) + z5*cos(e1)*cos(e3)*sin(e2)*sin(e4) - x5*cos(e1)*sin(e2)*sin(e3)*sin(e5) + y5*cos(e1)*cos(e2)*cos(e3)*cos(e5) + x5*cos(e1)*cos(e2)*cos(e4)*cos(e5)*sin(e3) + x5*cos(e1)*cos(e3)*cos(e4)*cos(e5)*sin(e2) - y5*cos(e1)*cos(e2)*cos(e4)*sin(e3)*sin(e5) - y5*cos(e1)*cos(e3)*cos(e4)*sin(e2)*sin(e5)) - 2*m4*(y4*sin(e1)*sin(e4) - x4*cos(e4)*sin(e1) + y4*cos(e1)*cos(e2)*cos(e4)*sin(e3) + y4*cos(e1)*cos(e3)*cos(e4)*sin(e2) + x4*cos(e1)*cos(e2)*sin(e3)*sin(e4) + x4*cos(e1)*cos(e3)*sin(e2)*sin(e4))*(a1*cos(e1) + a2*cos(e1)*sin(e2) + y4*cos(e4)*sin(e1) + x4*sin(e1)*sin(e4) + d4*cos(e1)*cos(e2)*cos(e3) + a3*cos(e1)*cos(e2)*sin(e3) + a3*cos(e1)*cos(e3)*sin(e2) + z4*cos(e1)*cos(e2)*cos(e3) - d4*cos(e1)*sin(e2)*sin(e3) - z4*cos(e1)*sin(e2)*sin(e3) + x4*cos(e1)*cos(e2)*cos(e4)*sin(e3) + x4*cos(e1)*cos(e3)*cos(e4)*sin(e2) - y4*cos(e1)*cos(e2)*sin(e3)*sin(e4) - y4*cos(e1)*cos(e3)*sin(e2)*sin(e4)) + 2*m6*(y6*cos(e6)*sin(e1)*sin(e4) + z6*cos(e4)*sin(e1)*sin(e5) + x6*sin(e1)*sin(e4)*sin(e6) - x6*cos(e4)*cos(e5)*cos(e6)*sin(e1) + y6*cos(e4)*cos(e5)*sin(e1)*sin(e6) + y6*cos(e1)*cos(e2)*cos(e4)*cos(e6)*sin(e3) + y6*cos(e1)*cos(e3)*cos(e4)*cos(e6)*sin(e2) + x6*cos(e1)*cos(e2)*cos(e4)*sin(e3)*sin(e6) + x6*cos(e1)*cos(e3)*cos(e4)*sin(e2)*sin(e6) - z6*cos(e1)*cos(e2)*sin(e3)*sin(e4)*sin(e5) - z6*cos(e1)*cos(e3)*sin(e2)*sin(e4)*sin(e5) + x6*cos(e1)*cos(e2)*cos(e5)*cos(e6)*sin(e3)*sin(e4) + x6*cos(e1)*cos(e3)*cos(e5)*cos(e6)*sin(e2)*sin(e4) - y6*cos(e1)*cos(e2)*cos(e5)*sin(e3)*sin(e4)*sin(e6) - y6*cos(e1)*cos(e3)*cos(e5)*sin(e2)*sin(e4)*sin(e6))*(d4*cos(e1)*sin(e2)*sin(e3) - a2*cos(e1)*sin(e2) - d4*cos(e1)*cos(e2)*cos(e3) - a3*cos(e1)*cos(e2)*sin(e3) - a3*cos(e1)*cos(e3)*sin(e2) - a1*cos(e1) - y6*cos(e4)*cos(e6)*sin(e1) - x6*cos(e4)*sin(e1)*sin(e6) + z6*sin(e1)*sin(e4)*sin(e5) - x6*cos(e5)*cos(e6)*sin(e1)*sin(e4) + z6*cos(e1)*cos(e5)*sin(e2)*sin(e3) + y6*cos(e5)*sin(e1)*sin(e4)*sin(e6) - z6*cos(e1)*cos(e2)*cos(e3)*cos(e5) - y6*cos(e1)*sin(e2)*sin(e3)*sin(e5)*sin(e6) - x6*cos(e1)*cos(e2)*cos(e3)*cos(e6)*sin(e5) + y6*cos(e1)*cos(e2)*cos(e6)*sin(e3)*sin(e4) + y6*cos(e1)*cos(e3)*cos(e6)*sin(e2)*sin(e4) + y6*cos(e1)*cos(e2)*cos(e3)*sin(e5)*sin(e6) + z6*cos(e1)*cos(e2)*cos(e4)*sin(e3)*sin(e5) + z6*cos(e1)*cos(e3)*cos(e4)*sin(e2)*sin(e5) + x6*cos(e1)*cos(e2)*sin(e3)*sin(e4)*sin(e6) + x6*cos(e1)*cos(e3)*sin(e2)*sin(e4)*sin(e6) + x6*cos(e1)*cos(e6)*sin(e2)*sin(e3)*sin(e5) - x6*cos(e1)*cos(e2)*cos(e4)*cos(e5)*cos(e6)*sin(e3) - x6*cos(e1)*cos(e3)*cos(e4)*cos(e5)*cos(e6)*sin(e2) + y6*cos(e1)*cos(e2)*cos(e4)*cos(e5)*sin(e3)*sin(e6) + y6*cos(e1)*cos(e3)*cos(e4)*cos(e5)*sin(e2)*sin(e6)) - 2*m6*(y6*cos(e1)*cos(e6)*sin(e4) + z6*cos(e1)*cos(e4)*sin(e5) + x6*cos(e1)*sin(e4)*sin(e6) + y6*cos(e1)*cos(e4)*cos(e5)*sin(e6) - x6*cos(e1)*cos(e4)*cos(e5)*cos(e6) + z6*cos(e2)*sin(e1)*sin(e3)*sin(e4)*sin(e5) + z6*cos(e3)*sin(e1)*sin(e2)*sin(e4)*sin(e5) - y6*cos(e2)*cos(e4)*cos(e6)*sin(e1)*sin(e3) - y6*cos(e3)*cos(e4)*cos(e6)*sin(e1)*sin(e2) - x6*cos(e2)*cos(e4)*sin(e1)*sin(e3)*sin(e6) - x6*cos(e3)*cos(e4)*sin(e1)*sin(e2)*sin(e6) - x6*cos(e2)*cos(e5)*cos(e6)*sin(e1)*sin(e3)*sin(e4) - x6*cos(e3)*cos(e5)*cos(e6)*sin(e1)*sin(e2)*sin(e4) + y6*cos(e2)*cos(e5)*sin(e1)*sin(e3)*sin(e4)*sin(e6) + y6*cos(e3)*cos(e5)*sin(e1)*sin(e2)*sin(e4)*sin(e6))*(y6*cos(e1)*cos(e4)*cos(e6) - a2*sin(e1)*sin(e2) - d4*cos(e2)*cos(e3)*sin(e1) - a1*sin(e1) - a3*cos(e2)*sin(e1)*sin(e3) - a3*cos(e3)*sin(e1)*sin(e2) + x6*cos(e1)*cos(e4)*sin(e6) + d4*sin(e1)*sin(e2)*sin(e3) - z6*cos(e1)*sin(e4)*sin(e5) + x6*cos(e1)*cos(e5)*cos(e6)*sin(e4) - z6*cos(e2)*cos(e3)*cos(e5)*sin(e1) - y6*cos(e1)*cos(e5)*sin(e4)*sin(e6) + z6*cos(e5)*sin(e1)*sin(e2)*sin(e3) + x6*cos(e2)*sin(e1)*sin(e3)*sin(e4)*sin(e6) + x6*cos(e3)*sin(e1)*sin(e2)*sin(e4)*sin(e6) + x6*cos(e6)*sin(e1)*sin(e2)*sin(e3)*sin(e5) - y6*sin(e1)*sin(e2)*sin(e3)*sin(e5)*sin(e6) - x6*cos(e2)*cos(e3)*cos(e6)*sin(e1)*sin(e5) + y6*cos(e2)*cos(e6)*sin(e1)*sin(e3)*sin(e4) + y6*cos(e3)*cos(e6)*sin(e1)*sin(e2)*sin(e4) + y6*cos(e2)*cos(e3)*sin(e1)*sin(e5)*sin(e6) + z6*cos(e2)*cos(e4)*sin(e1)*sin(e3)*sin(e5) + z6*cos(e3)*cos(e4)*sin(e1)*sin(e2)*sin(e5) - x6*cos(e2)*cos(e4)*cos(e5)*cos(e6)*sin(e1)*sin(e3) - x6*cos(e3)*cos(e4)*cos(e5)*cos(e6)*sin(e1)*sin(e2) + y6*cos(e2)*cos(e4)*cos(e5)*sin(e1)*sin(e3)*sin(e6) + y6*cos(e3)*cos(e4)*cos(e5)*sin(e1)*sin(e2)*sin(e6)) - 2*m4*(x4*cos(e1)*cos(e4) - y4*cos(e1)*sin(e4) + y4*cos(e2)*cos(e4)*sin(e1)*sin(e3) + y4*cos(e3)*cos(e4)*sin(e1)*sin(e2) + x4*cos(e2)*sin(e1)*sin(e3)*sin(e4) + x4*cos(e3)*sin(e1)*sin(e2)*sin(e4))*(a1*sin(e1) - y4*cos(e1)*cos(e4) + a2*sin(e1)*sin(e2) - x4*cos(e1)*sin(e4) + d4*cos(e2)*cos(e3)*sin(e1) + a3*cos(e2)*sin(e1)*sin(e3) + a3*cos(e3)*sin(e1)*sin(e2) + z4*cos(e2)*cos(e3)*sin(e1) - d4*sin(e1)*sin(e2)*sin(e3) - z4*sin(e1)*sin(e2)*sin(e3) + x4*cos(e2)*cos(e4)*sin(e1)*sin(e3) + x4*cos(e3)*cos(e4)*sin(e1)*sin(e2) - y4*cos(e2)*sin(e1)*sin(e3)*sin(e4) - y4*cos(e3)*sin(e1)*sin(e2)*sin(e4)) - 2*I4xx*cos(e2 + e3)^2*cos(e4)*sin(e4) + 2*I4yy*cos(e2 + e3)^2*cos(e4)*sin(e4) + 2*I5zz*cos(e2 + e3)^2*cos(e4)*sin(e4) + 2*I6xx*cos(e2 + e3)*(cos(e4)*sin(e6) + cos(e5)*cos(e6)*sin(e4))*(cos(e2 + e3)*sin(e4)*sin(e6) + sin(e2 + e3)*cos(e6)*sin(e5) - cos(e2 + e3)*cos(e4)*cos(e5)*cos(e6)) + 2*I6yy*cos(e2 + e3)*(cos(e4)*cos(e6) - cos(e5)*sin(e4)*sin(e6))*(cos(e2 + e3)*cos(e6)*sin(e4) - sin(e2 + e3)*sin(e5)*sin(e6) + cos(e2 + e3)*cos(e4)*cos(e5)*sin(e6)) + 2*I5xx*cos(e2 + e3)*cos(e5)*sin(e4)*(sin(e2 + e3)*sin(e5) - cos(e2 + e3)*cos(e4)*cos(e5)) - 2*I5yy*cos(e2 + e3)*sin(e4)*sin(e5)*(sin(e2 + e3)*cos(e5) + cos(e2 + e3)*cos(e4)*sin(e5)) - 2*I6zz*cos(e2 + e3)*sin(e4)*sin(e5)*(sin(e2 + e3)*cos(e5) + cos(e2 + e3)*cos(e4)*sin(e5))) + de2*(I3yy*sin(2*e2 + 2*e3) - I3xx*sin(2*e2 + 2*e3) + I4zz*sin(2*e2 + 2*e3) - I2xx*sin(2*e2) + I2yy*sin(2*e2) + 2*I5xx*(cos(e2 + e3)*sin(e5) + sin(e2 + e3)*cos(e4)*cos(e5))*(sin(e2 + e3)*sin(e5) - cos(e2 + e3)*cos(e4)*cos(e5)) + 2*I5yy*(sin(e2 + e3)*cos(e5) + cos(e2 + e3)*cos(e4)*sin(e5))*(cos(e2 + e3)*cos(e5) - sin(e2 + e3)*cos(e4)*sin(e5)) + 2*I6zz*(sin(e2 + e3)*cos(e5) + cos(e2 + e3)*cos(e4)*sin(e5))*(cos(e2 + e3)*cos(e5) - sin(e2 + e3)*cos(e4)*sin(e5)) + 2*I6xx*(cos(e2 + e3)*sin(e4)*sin(e6) + sin(e2 + e3)*cos(e6)*sin(e5) - cos(e2 + e3)*cos(e4)*cos(e5)*cos(e6))*(cos(e2 + e3)*cos(e6)*sin(e5) - sin(e2 + e3)*sin(e4)*sin(e6) + sin(e2 + e3)*cos(e4)*cos(e5)*cos(e6)) - 2*I6yy*(cos(e2 + e3)*cos(e6)*sin(e4) - sin(e2 + e3)*sin(e5)*sin(e6) + cos(e2 + e3)*cos(e4)*cos(e5)*sin(e6))*(sin(e2 + e3)*cos(e6)*sin(e4) + cos(e2 + e3)*sin(e5)*sin(e6) + sin(e2 + e3)*cos(e4)*cos(e5)*sin(e6)) - 2*m5*sin(e1)*(d4*cos(e2)*sin(e3) - a3*cos(e2)*cos(e3) - a2*cos(e2) + d4*cos(e3)*sin(e2) + a3*sin(e2)*sin(e3) + y5*cos(e2)*cos(e5)*sin(e3) + y5*cos(e3)*cos(e5)*sin(e2) - z5*cos(e2)*cos(e3)*sin(e4) + x5*cos(e2)*sin(e3)*sin(e5) + x5*cos(e3)*sin(e2)*sin(e5) + z5*sin(e2)*sin(e3)*sin(e4) + y5*cos(e2)*cos(e3)*cos(e4)*sin(e5) + x5*cos(e4)*cos(e5)*sin(e2)*sin(e3) - y5*cos(e4)*sin(e2)*sin(e3)*sin(e5) - x5*cos(e2)*cos(e3)*cos(e4)*cos(e5))*(a1*sin(e1) + z5*cos(e1)*cos(e4) + a2*sin(e1)*sin(e2) + d4*cos(e2)*cos(e3)*sin(e1) + a3*cos(e2)*sin(e1)*sin(e3) + a3*cos(e3)*sin(e1)*sin(e2) - x5*cos(e1)*cos(e5)*sin(e4) - d4*sin(e1)*sin(e2)*sin(e3) + y5*cos(e1)*sin(e4)*sin(e5) + y5*cos(e2)*cos(e3)*cos(e5)*sin(e1) + x5*cos(e2)*cos(e3)*sin(e1)*sin(e5) - y5*cos(e5)*sin(e1)*sin(e2)*sin(e3) + z5*cos(e2)*sin(e1)*sin(e3)*sin(e4) + z5*cos(e3)*sin(e1)*sin(e2)*sin(e4) - x5*sin(e1)*sin(e2)*sin(e3)*sin(e5) + x5*cos(e2)*cos(e4)*cos(e5)*sin(e1)*sin(e3) + x5*cos(e3)*cos(e4)*cos(e5)*sin(e1)*sin(e2) - y5*cos(e2)*cos(e4)*sin(e1)*sin(e3)*sin(e5) - y5*cos(e3)*cos(e4)*sin(e1)*sin(e2)*sin(e5)) - 2*I4yy*cos(e2 + e3)*sin(e2 + e3)*sin(e4)^2 - 2*I5zz*cos(e2 + e3)*sin(e2 + e3)*sin(e4)^2 + 2*m4*sin(e1)*((x4*cos(e2 + e3 - e4))/2 + (y4*sin(e2 + e3 - e4))/2 + a3*cos(e2 + e3) - d4*sin(e2 + e3) - z4*sin(e2 + e3) + a2*cos(e2) + (x4*cos(e2 + e3 + e4))/2 - (y4*sin(e2 + e3 + e4))/2)*(a1*sin(e1) - y4*cos(e1)*cos(e4) + a2*sin(e1)*sin(e2) - x4*cos(e1)*sin(e4) + d4*cos(e2)*cos(e3)*sin(e1) + a3*cos(e2)*sin(e1)*sin(e3) + a3*cos(e3)*sin(e1)*sin(e2) + z4*cos(e2)*cos(e3)*sin(e1) - d4*sin(e1)*sin(e2)*sin(e3) - z4*sin(e1)*sin(e2)*sin(e3) + x4*cos(e2)*cos(e4)*sin(e1)*sin(e3) + x4*cos(e3)*cos(e4)*sin(e1)*sin(e2) - y4*cos(e2)*sin(e1)*sin(e3)*sin(e4) - y4*cos(e3)*sin(e1)*sin(e2)*sin(e4)) + 2*m6*cos(e1)*(d4*cos(e2)*sin(e3) - a3*cos(e2)*cos(e3) - a2*cos(e2) + d4*cos(e3)*sin(e2) + a3*sin(e2)*sin(e3) + z6*cos(e2)*cos(e5)*sin(e3) + z6*cos(e3)*cos(e5)*sin(e2) + y6*cos(e2)*cos(e3)*cos(e6)*sin(e4) + z6*cos(e2)*cos(e3)*cos(e4)*sin(e5) + x6*cos(e2)*cos(e3)*sin(e4)*sin(e6) + x6*cos(e2)*cos(e6)*sin(e3)*sin(e5) + x6*cos(e3)*cos(e6)*sin(e2)*sin(e5) - y6*cos(e6)*sin(e2)*sin(e3)*sin(e4) - y6*cos(e2)*sin(e3)*sin(e5)*sin(e6) - y6*cos(e3)*sin(e2)*sin(e5)*sin(e6) - z6*cos(e4)*sin(e2)*sin(e3)*sin(e5) - x6*sin(e2)*sin(e3)*sin(e4)*sin(e6) - x6*cos(e2)*cos(e3)*cos(e4)*cos(e5)*cos(e6) + y6*cos(e2)*cos(e3)*cos(e4)*cos(e5)*sin(e6) + x6*cos(e4)*cos(e5)*cos(e6)*sin(e2)*sin(e3) - y6*cos(e4)*cos(e5)*sin(e2)*sin(e3)*sin(e6))*(d4*cos(e1)*sin(e2)*sin(e3) - a2*cos(e1)*sin(e2) - d4*cos(e1)*cos(e2)*cos(e3) - a3*cos(e1)*cos(e2)*sin(e3) - a3*cos(e1)*cos(e3)*sin(e2) - a1*cos(e1) - y6*cos(e4)*cos(e6)*sin(e1) - x6*cos(e4)*sin(e1)*sin(e6) + z6*sin(e1)*sin(e4)*sin(e5) - x6*cos(e5)*cos(e6)*sin(e1)*sin(e4) + z6*cos(e1)*cos(e5)*sin(e2)*sin(e3) + y6*cos(e5)*sin(e1)*sin(e4)*sin(e6) - z6*cos(e1)*cos(e2)*cos(e3)*cos(e5) - y6*cos(e1)*sin(e2)*sin(e3)*sin(e5)*sin(e6) - x6*cos(e1)*cos(e2)*cos(e3)*cos(e6)*sin(e5) + y6*cos(e1)*cos(e2)*cos(e6)*sin(e3)*sin(e4) + y6*cos(e1)*cos(e3)*cos(e6)*sin(e2)*sin(e4) + y6*cos(e1)*cos(e2)*cos(e3)*sin(e5)*sin(e6) + z6*cos(e1)*cos(e2)*cos(e4)*sin(e3)*sin(e5) + z6*cos(e1)*cos(e3)*cos(e4)*sin(e2)*sin(e5) + x6*cos(e1)*cos(e2)*sin(e3)*sin(e4)*sin(e6) + x6*cos(e1)*cos(e3)*sin(e2)*sin(e4)*sin(e6) + x6*cos(e1)*cos(e6)*sin(e2)*sin(e3)*sin(e5) - x6*cos(e1)*cos(e2)*cos(e4)*cos(e5)*cos(e6)*sin(e3) - x6*cos(e1)*cos(e3)*cos(e4)*cos(e5)*cos(e6)*sin(e2) + y6*cos(e1)*cos(e2)*cos(e4)*cos(e5)*sin(e3)*sin(e6) + y6*cos(e1)*cos(e3)*cos(e4)*cos(e5)*sin(e2)*sin(e6)) - 2*m5*cos(e1)*(d4*cos(e2)*sin(e3) - a3*cos(e2)*cos(e3) - a2*cos(e2) + d4*cos(e3)*sin(e2) + a3*sin(e2)*sin(e3) + y5*cos(e2)*cos(e5)*sin(e3) + y5*cos(e3)*cos(e5)*sin(e2) - z5*cos(e2)*cos(e3)*sin(e4) + x5*cos(e2)*sin(e3)*sin(e5) + x5*cos(e3)*sin(e2)*sin(e5) + z5*sin(e2)*sin(e3)*sin(e4) + y5*cos(e2)*cos(e3)*cos(e4)*sin(e5) + x5*cos(e4)*cos(e5)*sin(e2)*sin(e3) - y5*cos(e4)*sin(e2)*sin(e3)*sin(e5) - x5*cos(e2)*cos(e3)*cos(e4)*cos(e5))*(a1*cos(e1) + a2*cos(e1)*sin(e2) - z5*cos(e4)*sin(e1) + d4*cos(e1)*cos(e2)*cos(e3) + a3*cos(e1)*cos(e2)*sin(e3) + a3*cos(e1)*cos(e3)*sin(e2) - d4*cos(e1)*sin(e2)*sin(e3) + x5*cos(e5)*sin(e1)*sin(e4) - y5*sin(e1)*sin(e4)*sin(e5) + x5*cos(e1)*cos(e2)*cos(e3)*sin(e5) - y5*cos(e1)*cos(e5)*sin(e2)*sin(e3) + z5*cos(e1)*cos(e2)*sin(e3)*sin(e4) + z5*cos(e1)*cos(e3)*sin(e2)*sin(e4) - x5*cos(e1)*sin(e2)*sin(e3)*sin(e5) + y5*cos(e1)*cos(e2)*cos(e3)*cos(e5) + x5*cos(e1)*cos(e2)*cos(e4)*cos(e5)*sin(e3) + x5*cos(e1)*cos(e3)*cos(e4)*cos(e5)*sin(e2) - y5*cos(e1)*cos(e2)*cos(e4)*sin(e3)*sin(e5) - y5*cos(e1)*cos(e3)*cos(e4)*sin(e2)*sin(e5)) + 2*m6*sin(e1)*(d4*cos(e2)*sin(e3) - a3*cos(e2)*cos(e3) - a2*cos(e2) + d4*cos(e3)*sin(e2) + a3*sin(e2)*sin(e3) + z6*cos(e2)*cos(e5)*sin(e3) + z6*cos(e3)*cos(e5)*sin(e2) + y6*cos(e2)*cos(e3)*cos(e6)*sin(e4) + z6*cos(e2)*cos(e3)*cos(e4)*sin(e5) + x6*cos(e2)*cos(e3)*sin(e4)*sin(e6) + x6*cos(e2)*cos(e6)*sin(e3)*sin(e5) + x6*cos(e3)*cos(e6)*sin(e2)*sin(e5) - y6*cos(e6)*sin(e2)*sin(e3)*sin(e4) - y6*cos(e2)*sin(e3)*sin(e5)*sin(e6) - y6*cos(e3)*sin(e2)*sin(e5)*sin(e6) - z6*cos(e4)*sin(e2)*sin(e3)*sin(e5) - x6*sin(e2)*sin(e3)*sin(e4)*sin(e6) - x6*cos(e2)*cos(e3)*cos(e4)*cos(e5)*cos(e6) + y6*cos(e2)*cos(e3)*cos(e4)*cos(e5)*sin(e6) + x6*cos(e4)*cos(e5)*cos(e6)*sin(e2)*sin(e3) - y6*cos(e4)*cos(e5)*sin(e2)*sin(e3)*sin(e6))*(y6*cos(e1)*cos(e4)*cos(e6) - a2*sin(e1)*sin(e2) - d4*cos(e2)*cos(e3)*sin(e1) - a1*sin(e1) - a3*cos(e2)*sin(e1)*sin(e3) - a3*cos(e3)*sin(e1)*sin(e2) + x6*cos(e1)*cos(e4)*sin(e6) + d4*sin(e1)*sin(e2)*sin(e3) - z6*cos(e1)*sin(e4)*sin(e5) + x6*cos(e1)*cos(e5)*cos(e6)*sin(e4) - z6*cos(e2)*cos(e3)*cos(e5)*sin(e1) - y6*cos(e1)*cos(e5)*sin(e4)*sin(e6) + z6*cos(e5)*sin(e1)*sin(e2)*sin(e3) + x6*cos(e2)*sin(e1)*sin(e3)*sin(e4)*sin(e6) + x6*cos(e3)*sin(e1)*sin(e2)*sin(e4)*sin(e6) + x6*cos(e6)*sin(e1)*sin(e2)*sin(e3)*sin(e5) - y6*sin(e1)*sin(e2)*sin(e3)*sin(e5)*sin(e6) - x6*cos(e2)*cos(e3)*cos(e6)*sin(e1)*sin(e5) + y6*cos(e2)*cos(e6)*sin(e1)*sin(e3)*sin(e4) + y6*cos(e3)*cos(e6)*sin(e1)*sin(e2)*sin(e4) + y6*cos(e2)*cos(e3)*sin(e1)*sin(e5)*sin(e6) + z6*cos(e2)*cos(e4)*sin(e1)*sin(e3)*sin(e5) + z6*cos(e3)*cos(e4)*sin(e1)*sin(e2)*sin(e5) - x6*cos(e2)*cos(e4)*cos(e5)*cos(e6)*sin(e1)*sin(e3) - x6*cos(e3)*cos(e4)*cos(e5)*cos(e6)*sin(e1)*sin(e2) + y6*cos(e2)*cos(e4)*cos(e5)*sin(e1)*sin(e3)*sin(e6) + y6*cos(e3)*cos(e4)*cos(e5)*sin(e1)*sin(e2)*sin(e6)) + 2*m3*sin(e1)*(x3*cos(e2 + e3) - y3*sin(e2 + e3) + a2*cos(e2))*(sin(e1)*(a1 + y3*cos(e2 + e3) + x3*sin(e2 + e3) + a2*sin(e2)) + z3*cos(e2 + e3)^2*cos(e1) + z3*sin(e2 + e3)^2*cos(e1)) - 2*m3*cos(e1)*(z3*cos(e2 + e3)^2*sin(e1) - cos(e1)*(a1 + y3*cos(e2 + e3) + x3*sin(e2 + e3) + a2*sin(e2)) + z3*sin(e2 + e3)^2*sin(e1))*(x3*cos(e2 + e3) - y3*sin(e2 + e3) + a2*cos(e2)) + 2*m4*cos(e1)*((x4*cos(e2 + e3 - e4))/2 + (y4*sin(e2 + e3 - e4))/2 + a3*cos(e2 + e3) - d4*sin(e2 + e3) - z4*sin(e2 + e3) + a2*cos(e2) + (x4*cos(e2 + e3 + e4))/2 - (y4*sin(e2 + e3 + e4))/2)*(a1*cos(e1) + a2*cos(e1)*sin(e2) + y4*cos(e4)*sin(e1) + x4*sin(e1)*sin(e4) + d4*cos(e1)*cos(e2)*cos(e3) + a3*cos(e1)*cos(e2)*sin(e3) + a3*cos(e1)*cos(e3)*sin(e2) + z4*cos(e1)*cos(e2)*cos(e3) - d4*cos(e1)*sin(e2)*sin(e3) - z4*cos(e1)*sin(e2)*sin(e3) + x4*cos(e1)*cos(e2)*cos(e4)*sin(e3) + x4*cos(e1)*cos(e3)*cos(e4)*sin(e2) - y4*cos(e1)*cos(e2)*sin(e3)*sin(e4) - y4*cos(e1)*cos(e3)*sin(e2)*sin(e4)) + 2*m2*cos(e1)*(x2*cos(e2) - y2*sin(e2))*(a1*cos(e1) - z2*sin(e1) + y2*cos(e1)*cos(e2) + x2*cos(e1)*sin(e2)) + 2*m2*sin(e1)*(x2*cos(e2) - y2*sin(e2))*(a1*sin(e1) + z2*cos(e1) + y2*cos(e2)*sin(e1) + x2*sin(e1)*sin(e2)) - 2*I4xx*cos(e2 + e3)*sin(e2 + e3)*cos(e4)^2) + de3*(I3yy*sin(2*e2 + 2*e3) - I3xx*sin(2*e2 + 2*e3) + I4zz*sin(2*e2 + 2*e3) + 2*I5xx*(cos(e2 + e3)*sin(e5) + sin(e2 + e3)*cos(e4)*cos(e5))*(sin(e2 + e3)*sin(e5) - cos(e2 + e3)*cos(e4)*cos(e5)) + 2*I5yy*(sin(e2 + e3)*cos(e5) + cos(e2 + e3)*cos(e4)*sin(e5))*(cos(e2 + e3)*cos(e5) - sin(e2 + e3)*cos(e4)*sin(e5)) + 2*I6zz*(sin(e2 + e3)*cos(e5) + cos(e2 + e3)*cos(e4)*sin(e5))*(cos(e2 + e3)*cos(e5) - sin(e2 + e3)*cos(e4)*sin(e5)) + 2*I6xx*(cos(e2 + e3)*sin(e4)*sin(e6) + sin(e2 + e3)*cos(e6)*sin(e5) - cos(e2 + e3)*cos(e4)*cos(e5)*cos(e6))*(cos(e2 + e3)*cos(e6)*sin(e5) - sin(e2 + e3)*sin(e4)*sin(e6) + sin(e2 + e3)*cos(e4)*cos(e5)*cos(e6)) - 2*I6yy*(cos(e2 + e3)*cos(e6)*sin(e4) - sin(e2 + e3)*sin(e5)*sin(e6) + cos(e2 + e3)*cos(e4)*cos(e5)*sin(e6))*(sin(e2 + e3)*cos(e6)*sin(e4) + cos(e2 + e3)*sin(e5)*sin(e6) + sin(e2 + e3)*cos(e4)*cos(e5)*sin(e6)) - 2*I4yy*cos(e2 + e3)*sin(e2 + e3)*sin(e4)^2 - 2*I5zz*cos(e2 + e3)*sin(e2 + e3)*sin(e4)^2 - 2*m5*sin(e1)*(d4*cos(e2)*sin(e3) - a3*cos(e2)*cos(e3) + d4*cos(e3)*sin(e2) + a3*sin(e2)*sin(e3) + y5*cos(e2)*cos(e5)*sin(e3) + y5*cos(e3)*cos(e5)*sin(e2) - z5*cos(e2)*cos(e3)*sin(e4) + x5*cos(e2)*sin(e3)*sin(e5) + x5*cos(e3)*sin(e2)*sin(e5) + z5*sin(e2)*sin(e3)*sin(e4) + y5*cos(e2)*cos(e3)*cos(e4)*sin(e5) + x5*cos(e4)*cos(e5)*sin(e2)*sin(e3) - y5*cos(e4)*sin(e2)*sin(e3)*sin(e5) - x5*cos(e2)*cos(e3)*cos(e4)*cos(e5))*(a1*sin(e1) + z5*cos(e1)*cos(e4) + a2*sin(e1)*sin(e2) + d4*cos(e2)*cos(e3)*sin(e1) + a3*cos(e2)*sin(e1)*sin(e3) + a3*cos(e3)*sin(e1)*sin(e2) - x5*cos(e1)*cos(e5)*sin(e4) - d4*sin(e1)*sin(e2)*sin(e3) + y5*cos(e1)*sin(e4)*sin(e5) + y5*cos(e2)*cos(e3)*cos(e5)*sin(e1) + x5*cos(e2)*cos(e3)*sin(e1)*sin(e5) - y5*cos(e5)*sin(e1)*sin(e2)*sin(e3) + z5*cos(e2)*sin(e1)*sin(e3)*sin(e4) + z5*cos(e3)*sin(e1)*sin(e2)*sin(e4) - x5*sin(e1)*sin(e2)*sin(e3)*sin(e5) + x5*cos(e2)*cos(e4)*cos(e5)*sin(e1)*sin(e3) + x5*cos(e3)*cos(e4)*cos(e5)*sin(e1)*sin(e2) - y5*cos(e2)*cos(e4)*sin(e1)*sin(e3)*sin(e5) - y5*cos(e3)*cos(e4)*sin(e1)*sin(e2)*sin(e5)) + 2*m4*sin(e1)*((x4*cos(e2 + e3 - e4))/2 + (y4*sin(e2 + e3 - e4))/2 + a3*cos(e2 + e3) - d4*sin(e2 + e3) - z4*sin(e2 + e3) + (x4*cos(e2 + e3 + e4))/2 - (y4*sin(e2 + e3 + e4))/2)*(a1*sin(e1) - y4*cos(e1)*cos(e4) + a2*sin(e1)*sin(e2) - x4*cos(e1)*sin(e4) + d4*cos(e2)*cos(e3)*sin(e1) + a3*cos(e2)*sin(e1)*sin(e3) + a3*cos(e3)*sin(e1)*sin(e2) + z4*cos(e2)*cos(e3)*sin(e1) - d4*sin(e1)*sin(e2)*sin(e3) - z4*sin(e1)*sin(e2)*sin(e3) + x4*cos(e2)*cos(e4)*sin(e1)*sin(e3) + x4*cos(e3)*cos(e4)*sin(e1)*sin(e2) - y4*cos(e2)*sin(e1)*sin(e3)*sin(e4) - y4*cos(e3)*sin(e1)*sin(e2)*sin(e4)) + 2*m6*cos(e1)*(d4*cos(e2)*sin(e3) - a3*cos(e2)*cos(e3) + d4*cos(e3)*sin(e2) + a3*sin(e2)*sin(e3) + z6*cos(e2)*cos(e5)*sin(e3) + z6*cos(e3)*cos(e5)*sin(e2) + y6*cos(e2)*cos(e3)*cos(e6)*sin(e4) + z6*cos(e2)*cos(e3)*cos(e4)*sin(e5) + x6*cos(e2)*cos(e3)*sin(e4)*sin(e6) + x6*cos(e2)*cos(e6)*sin(e3)*sin(e5) + x6*cos(e3)*cos(e6)*sin(e2)*sin(e5) - y6*cos(e6)*sin(e2)*sin(e3)*sin(e4) - y6*cos(e2)*sin(e3)*sin(e5)*sin(e6) - y6*cos(e3)*sin(e2)*sin(e5)*sin(e6) - z6*cos(e4)*sin(e2)*sin(e3)*sin(e5) - x6*sin(e2)*sin(e3)*sin(e4)*sin(e6) - x6*cos(e2)*cos(e3)*cos(e4)*cos(e5)*cos(e6) + y6*cos(e2)*cos(e3)*cos(e4)*cos(e5)*sin(e6) + x6*cos(e4)*cos(e5)*cos(e6)*sin(e2)*sin(e3) - y6*cos(e4)*cos(e5)*sin(e2)*sin(e3)*sin(e6))*(d4*cos(e1)*sin(e2)*sin(e3) - a2*cos(e1)*sin(e2) - d4*cos(e1)*cos(e2)*cos(e3) - a3*cos(e1)*cos(e2)*sin(e3) - a3*cos(e1)*cos(e3)*sin(e2) - a1*cos(e1) - y6*cos(e4)*cos(e6)*sin(e1) - x6*cos(e4)*sin(e1)*sin(e6) + z6*sin(e1)*sin(e4)*sin(e5) - x6*cos(e5)*cos(e6)*sin(e1)*sin(e4) + z6*cos(e1)*cos(e5)*sin(e2)*sin(e3) + y6*cos(e5)*sin(e1)*sin(e4)*sin(e6) - z6*cos(e1)*cos(e2)*cos(e3)*cos(e5) - y6*cos(e1)*sin(e2)*sin(e3)*sin(e5)*sin(e6) - x6*cos(e1)*cos(e2)*cos(e3)*cos(e6)*sin(e5) + y6*cos(e1)*cos(e2)*cos(e6)*sin(e3)*sin(e4) + y6*cos(e1)*cos(e3)*cos(e6)*sin(e2)*sin(e4) + y6*cos(e1)*cos(e2)*cos(e3)*sin(e5)*sin(e6) + z6*cos(e1)*cos(e2)*cos(e4)*sin(e3)*sin(e5) + z6*cos(e1)*cos(e3)*cos(e4)*sin(e2)*sin(e5) + x6*cos(e1)*cos(e2)*sin(e3)*sin(e4)*sin(e6) + x6*cos(e1)*cos(e3)*sin(e2)*sin(e4)*sin(e6) + x6*cos(e1)*cos(e6)*sin(e2)*sin(e3)*sin(e5) - x6*cos(e1)*cos(e2)*cos(e4)*cos(e5)*cos(e6)*sin(e3) - x6*cos(e1)*cos(e3)*cos(e4)*cos(e5)*cos(e6)*sin(e2) + y6*cos(e1)*cos(e2)*cos(e4)*cos(e5)*sin(e3)*sin(e6) + y6*cos(e1)*cos(e3)*cos(e4)*cos(e5)*sin(e2)*sin(e6)) - 2*m5*cos(e1)*(d4*cos(e2)*sin(e3) - a3*cos(e2)*cos(e3) + d4*cos(e3)*sin(e2) + a3*sin(e2)*sin(e3) + y5*cos(e2)*cos(e5)*sin(e3) + y5*cos(e3)*cos(e5)*sin(e2) - z5*cos(e2)*cos(e3)*sin(e4) + x5*cos(e2)*sin(e3)*sin(e5) + x5*cos(e3)*sin(e2)*sin(e5) + z5*sin(e2)*sin(e3)*sin(e4) + y5*cos(e2)*cos(e3)*cos(e4)*sin(e5) + x5*cos(e4)*cos(e5)*sin(e2)*sin(e3) - y5*cos(e4)*sin(e2)*sin(e3)*sin(e5) - x5*cos(e2)*cos(e3)*cos(e4)*cos(e5))*(a1*cos(e1) + a2*cos(e1)*sin(e2) - z5*cos(e4)*sin(e1) + d4*cos(e1)*cos(e2)*cos(e3) + a3*cos(e1)*cos(e2)*sin(e3) + a3*cos(e1)*cos(e3)*sin(e2) - d4*cos(e1)*sin(e2)*sin(e3) + x5*cos(e5)*sin(e1)*sin(e4) - y5*sin(e1)*sin(e4)*sin(e5) + x5*cos(e1)*cos(e2)*cos(e3)*sin(e5) - y5*cos(e1)*cos(e5)*sin(e2)*sin(e3) + z5*cos(e1)*cos(e2)*sin(e3)*sin(e4) + z5*cos(e1)*cos(e3)*sin(e2)*sin(e4) - x5*cos(e1)*sin(e2)*sin(e3)*sin(e5) + y5*cos(e1)*cos(e2)*cos(e3)*cos(e5) + x5*cos(e1)*cos(e2)*cos(e4)*cos(e5)*sin(e3) + x5*cos(e1)*cos(e3)*cos(e4)*cos(e5)*sin(e2) - y5*cos(e1)*cos(e2)*cos(e4)*sin(e3)*sin(e5) - y5*cos(e1)*cos(e3)*cos(e4)*sin(e2)*sin(e5)) + 2*m6*sin(e1)*(d4*cos(e2)*sin(e3) - a3*cos(e2)*cos(e3) + d4*cos(e3)*sin(e2) + a3*sin(e2)*sin(e3) + z6*cos(e2)*cos(e5)*sin(e3) + z6*cos(e3)*cos(e5)*sin(e2) + y6*cos(e2)*cos(e3)*cos(e6)*sin(e4) + z6*cos(e2)*cos(e3)*cos(e4)*sin(e5) + x6*cos(e2)*cos(e3)*sin(e4)*sin(e6) + x6*cos(e2)*cos(e6)*sin(e3)*sin(e5) + x6*cos(e3)*cos(e6)*sin(e2)*sin(e5) - y6*cos(e6)*sin(e2)*sin(e3)*sin(e4) - y6*cos(e2)*sin(e3)*sin(e5)*sin(e6) - y6*cos(e3)*sin(e2)*sin(e5)*sin(e6) - z6*cos(e4)*sin(e2)*sin(e3)*sin(e5) - x6*sin(e2)*sin(e3)*sin(e4)*sin(e6) - x6*cos(e2)*cos(e3)*cos(e4)*cos(e5)*cos(e6) + y6*cos(e2)*cos(e3)*cos(e4)*cos(e5)*sin(e6) + x6*cos(e4)*cos(e5)*cos(e6)*sin(e2)*sin(e3) - y6*cos(e4)*cos(e5)*sin(e2)*sin(e3)*sin(e6))*(y6*cos(e1)*cos(e4)*cos(e6) - a2*sin(e1)*sin(e2) - d4*cos(e2)*cos(e3)*sin(e1) - a1*sin(e1) - a3*cos(e2)*sin(e1)*sin(e3) - a3*cos(e3)*sin(e1)*sin(e2) + x6*cos(e1)*cos(e4)*sin(e6) + d4*sin(e1)*sin(e2)*sin(e3) - z6*cos(e1)*sin(e4)*sin(e5) + x6*cos(e1)*cos(e5)*cos(e6)*sin(e4) - z6*cos(e2)*cos(e3)*cos(e5)*sin(e1) - y6*cos(e1)*cos(e5)*sin(e4)*sin(e6) + z6*cos(e5)*sin(e1)*sin(e2)*sin(e3) + x6*cos(e2)*sin(e1)*sin(e3)*sin(e4)*sin(e6) + x6*cos(e3)*sin(e1)*sin(e2)*sin(e4)*sin(e6) + x6*cos(e6)*sin(e1)*sin(e2)*sin(e3)*sin(e5) - y6*sin(e1)*sin(e2)*sin(e3)*sin(e5)*sin(e6) - x6*cos(e2)*cos(e3)*cos(e6)*sin(e1)*sin(e5) + y6*cos(e2)*cos(e6)*sin(e1)*sin(e3)*sin(e4) + y6*cos(e3)*cos(e6)*sin(e1)*sin(e2)*sin(e4) + y6*cos(e2)*cos(e3)*sin(e1)*sin(e5)*sin(e6) + z6*cos(e2)*cos(e4)*sin(e1)*sin(e3)*sin(e5) + z6*cos(e3)*cos(e4)*sin(e1)*sin(e2)*sin(e5) - x6*cos(e2)*cos(e4)*cos(e5)*cos(e6)*sin(e1)*sin(e3) - x6*cos(e3)*cos(e4)*cos(e5)*cos(e6)*sin(e1)*sin(e2) + y6*cos(e2)*cos(e4)*cos(e5)*sin(e1)*sin(e3)*sin(e6) + y6*cos(e3)*cos(e4)*cos(e5)*sin(e1)*sin(e2)*sin(e6)) + 2*m3*sin(e1)*(x3*cos(e2 + e3) - y3*sin(e2 + e3))*(sin(e1)*(a1 + y3*cos(e2 + e3) + x3*sin(e2 + e3) + a2*sin(e2)) + z3*cos(e2 + e3)^2*cos(e1) + z3*sin(e2 + e3)^2*cos(e1)) - 2*m3*cos(e1)*(x3*cos(e2 + e3) - y3*sin(e2 + e3))*(z3*cos(e2 + e3)^2*sin(e1) - cos(e1)*(a1 + y3*cos(e2 + e3) + x3*sin(e2 + e3) + a2*sin(e2)) + z3*sin(e2 + e3)^2*sin(e1)) + 2*m4*cos(e1)*((x4*cos(e2 + e3 - e4))/2 + (y4*sin(e2 + e3 - e4))/2 + a3*cos(e2 + e3) - d4*sin(e2 + e3) - z4*sin(e2 + e3) + (x4*cos(e2 + e3 + e4))/2 - (y4*sin(e2 + e3 + e4))/2)*(a1*cos(e1) + a2*cos(e1)*sin(e2) + y4*cos(e4)*sin(e1) + x4*sin(e1)*sin(e4) + d4*cos(e1)*cos(e2)*cos(e3) + a3*cos(e1)*cos(e2)*sin(e3) + a3*cos(e1)*cos(e3)*sin(e2) + z4*cos(e1)*cos(e2)*cos(e3) - d4*cos(e1)*sin(e2)*sin(e3) - z4*cos(e1)*sin(e2)*sin(e3) + x4*cos(e1)*cos(e2)*cos(e4)*sin(e3) + x4*cos(e1)*cos(e3)*cos(e4)*sin(e2) - y4*cos(e1)*cos(e2)*sin(e3)*sin(e4) - y4*cos(e1)*cos(e3)*sin(e2)*sin(e4)) - 2*I4xx*cos(e2 + e3)*sin(e2 + e3)*cos(e4)^2);
